simulink model "RB_KAIROS_ArmOnly"  (R2020b)
(part 7 of 17)

t16181 = t3764+t3803+t3810+t3948+t4046+t4050+t4085+t4119+t4165+t4176+t4208+t4212+t4219+t4891+t4926+t4971+t5056+t5175+t5372+t5398+t5435+t5678+t5816+t5817+t6021+t6040+t6076+t6086+t6176+t6724+t6737+t6766+t6881+t6904+t7297+t7298+t7325+t7333+t7439+t7441+t7695+t7716+t7729+t7766+t7770+t7775+t8247+t8476+t8744+t9023+t9032+t9189+t9280+t9289+t9472+t9487+t9501+t9516+t9517+t9646+t9671+t9683+t10139+t10140;
t16199 = q2d.*t16197;
t16214 = t3314+t3315+t3427+t3482+t4058+t4077+t4567+t4627+t4680+t4712+t5459+t5460+t5960+t5966+t5967+t5982+t5983+t5985+t6049+t6067+t6799+t6800+t6849+t6850+t6973+t7051+t7182+t7187+t7194+t7196+t7830+t7883+t8123+t8126+t8203+t8215+t9704+t9713+t9722+t9734+t9976+t9977+t11086+t11087+t11091+t11095+t11106+t11107+t12225+t12226+t12670+t12678+t12680+t12681;
t16218 = q2d.*t16217;
t16236 = t3357+t3450+t3475+t3557+t3579+t3599+t3661+t3722+t3729+t3737+t3906+t3994+t4041+t4051+t4096+t4548+t4568+t4707+t4734+t4818+t4820+t4827+t4853+t4866+t4875+t4912+t4918+t4919+t4920+t5000+t5060+t5416+t5432+t5743+t5753+t5962+t5968+t5970+t5992+t6010+t6020+t6022+t6028+t6093+t6094+t6098+t6127+t6144+t6178+t6189+t6201+t6208+t6279+t6296+t6531+t6656+t6659+t6736+t6765+t6785+t6817+t6954+t7044+t7146+t7222+t7244+t7331+t7334+t7466+t7560+t7689+t7701+t7707+t7713+t8133+t8154+t8198+t8248+t8665+t8757+t8764+t9071+t9188+t9731+t9735+t9782+t9816+t9847+t9867+t10001+t10004+t10038+t10117+t10134+t10178+t10374+t10396;
t16238 = q3d.*t16237;
t16242 = t7826+t8162+t8296+t9175+t9204+t15016+t15218+t16107+t16108+t16109+t16111;
t16254 = t4446+t4631+t4668+t4758+t4768+t5004+t5033+t5197+t5236+t5240+t5250+t7135+t7185+t8618+t8671+t9067+t9259+t13711+t13717+t14544+t14866+t15496+t15502+t15557+t15559+t15561+t15564+t15663+t15664;
t16255 = t4446+t4631+t4668+t4758+t4796+t5004+t5033+t5186+t5242+t5249+t5260+t7125+t7190+t8614+t8666+t9074+t9268+t13711+t13717+t14543+t14862+t15500+t15501+t15556+t15560+t15562+t15563+t15662+t15665;
t16256 = -phid.*(-t4446-t4631-t4668-t4758+t4796+t5014+t5186+t5242+t5249+t5260+t7125+t7190+t8614+t8666+t9074+t9268-t13711+t13715+t14543+t14862+t15500+t15501+t15556+t15560+t15562+t15563+t15662+t15665+t9.*(t348-t525).*8.36241330891889e-4);
t16257 = t4001+t4040+t4652+t4658+t4762+t4785+t4804+t4825+t5253+t5305+t5766+t5791+t7139+t7199+t7204+t8632+t8677+t8904+t9266+t12013+t12015+t12020+t12023+t14555+t14872+t15553+t15555+t15600+t15602+t15607+t15609+t15671+t15672;
t16262 = q2d.*t16261;
t16264 = phid.*t16263;
t16265 = t4407+t4421+t4425+t4429+t4481+t4483+t4903+t4904+t6045+t6411+t6493+t6980+t7029+t7229+t7257+t7327+t8679+t8729+t9991+t9999+t10137+t10723+t12542+t12543+t14808+t14997+t15641+t15646+t15655+t15657+t15682+t15684+t15712+t15714;
t16270 = t4279+t4301+t4305+t4485+t4490+t4518+t4805+t4821+t6374+t6610+t6717+t7397+t7407+t7467+t7795+t7880+t8771+t8847+t10399+t10786+t10943+t10951+t12578+t12579+t14854+t15028+t15692+t15694+t15717+t15718+t15730+t15731+t15751+t15756;
t16271 = phid.*t16269;
t16284 = t3023+t3028+t3789+t3832+t3838+t3847+t3862+t3952+t3954+t3962+t4074+t4086+t4088+t4114+t4156+t4256+t4304+t4824+t4869+t4965+t5075+t5155+t5189+t5271+t5301+t5332+t5335+t5388+t5710+t5794+t5863+t5878+t5886+t6132+t6219+t6237+t6421+t6617+t6657+t6791+t6880+t6898+t6940+t6942+t6963+t6986+t7009+t7100+t7180+t7242+t7299+t7471+t7508+t7570+t7578+t7688+t7733+t7813+t7862+t7863+t7994+t8010+t8089+t8261+t8305+t8565+t8567+t8581+t8839+t8853+t9132+t9211+t9234+t9241+t9250+t9260+t9299+t9328+t9357+t9385+t9409+t9786+t9798+t9947+t10016+t10021+t10168+t10239+t10256+t10679+t10848+t11021+t11028+t11033+t11124+t11334+t11342+t11499+t11500+t11512+t11558+t11577+t11788+t11807;
t16285 = t2955+t2968+t3789+t3801+t3811+t3834+t3896+t3931+t3952+t3962+t4069+t4098+t4107+t4147+t4195+t4280+t4287+t4824+t4869+t4965+t5063+t5155+t5189+t5271+t5311+t5335+t5343+t5388+t5710+t5794+t5863+t5878+t5886+t6132+t6219+t6237+t6421+t6617+t6657+t6791+t6898+t6903+t6940+t6942+t6943+t6986+t7009+t7100+t7180+t7242+t7299+t7476+t7495+t7578+t7585+t7688+t7733+t7813+t7862+t7863+t7984+t8029+t8089+t8261+t8305+t8565+t8572+t8581+t8839+t8853+t9132+t9211+t9234+t9241+t9250+t9260+t9299+t9328+t9345+t9392+t9395+t9786+t9798+t9954+t10016+t10021+t10168+t10243+t10247+t10656+t10848+t11026+t11027+t11033+t11124+t11334+t11342+t11499+t11500+t11512+t11558+t11577+t11788+t11807;
t16325 = t2162+t2193+t2295+t2486+t2503+t2521+t3273+t3298+t3526+t3558+t3662+t3664+t3705+t3754+t3946+t4045+t4647+t4661+t4710+t4733+t4735+t4761+t4789+t4791+t4811+t4815+t4833+t4839+t4850+t4858+t4871+t4979+t4986+t5073+t5103+t5247+t5304+t5650+t5665+t5779+t5809+t5857+t5887+t5945+t6034+t6148+t6171+t6232+t6235+t6313+t6315+t6320+t6330+t6333+t6335+t6351+t6490+t6512+t6536+t6567+t6581+t6777+t6789+t6926+t6977+t7028+t7053+t7077+t7119+t7163+t7168+t7202+t7206+t7209+t7359+t7404+t7480+t7517+t7629+t7685+t7704+t7730+t7866+t7922+t8011+t8012+t8066+t8084+t8088+t8328+t8330+t8541+t8556+t8975+t9053+t9059+t9135+t9137+t9220+t9224+t9373+t9423+t9533+t9535+t9781+t9832+t9907+t9913+t10045+t10054+t10087+t10107+t10205+t10225+t10669+t10781+t10918+t11072+t11151+t11292+t11298+t11311+t11493+t11495+t11514+t11582+t11590+t11612+t11613+t11957+t11963+t11971+t11973;
t16327 = t2162+t2193+t2295+t2502+t2526+t2555+t3273+t3298+t3454+t3606+t3609+t3691+t3705+t3754+t3946+t4027+t4610+t4678+t4694+t4709+t4750+t4790+t4807+t4810+t4819+t4828+t4829+t4842+t4848+t4858+t4859+t4977+t4991+t5073+t5103+t5259+t5295+t5663+t5677+t5779+t5793+t5857+t5876+t5921+t6015+t6128+t6152+t6244+t6248+t6314+t6318+t6320+t6329+t6331+t6350+t6366+t6490+t6523+t6536+t6567+t6581+t6789+t6790+t6926+t6977+t7034+t7047+t7063+t7127+t7147+t7177+t7212+t7218+t7221+t7378+t7416+t7473+t7517+t7629+t7670+t7687+t7730+t7881+t7934+t8030+t8031+t8083+t8084+t8106+t8323+t8338+t8541+t8556+t8975+t9045+t9064+t9130+t9135+t9227+t9238+t9373+t9423+t9545+t9546+t9794+t9821+t9907+t9913+t10033+t10054+t10072+t10093+t10211+t10220+t10647+t10785+t10926+t11072+t11158+t11292+t11298+t11311+t11493+t11495+t11518+t11589+t11597+t11607+t11608+t11952+t11955+t11958+t11964;
t10434 = -t10423;
t10522 = -t10515;
t10601 = -t10592;
t10636 = -t10625;
t10855 = -t10853;
t11011 = -t11004;
t11169 = -t11156;
t11289 = -t11280;
t11406 = -t11395;
t11656 = -t11643;
t11703 = -t11695;
t11828 = -t11823;
t11879 = -t11876;
t11936 = -t11932;
t11998 = -t11992;
t12085 = -t12081;
t12099 = -t12096;
t12121 = -t12115;
t12156 = -t12149;
t12172 = -t12166;
t12285 = -t12282;
t12383 = -t12381;
t12428 = -t12424;
t12434 = t12332.*7.35522e-1;
t12435 = t12333.*7.35522e-1;
t12444 = -t12440;
t12481 = -t12478;
t12488 = t8533+t10393;
t12491 = t8539+t10395;
t12497 = -t12494;
t12498 = -t12495;
t12499 = -t12496;
t12521 = t12333.*3.867742437e-3;
t12523 = t12332.*1.563719772e-3;
t12526 = -t12522;
t12580 = -t12570;
t12581 = -t12571;
t12592 = t16.*t12487.*2.62925e-3;
t12610 = t8.*t12508.*2.62925e-3;
t12611 = -t12607;
t12663 = -t12653;
t12666 = -t12656;
t12684 = (t2501.*t12487)./4.0;
t12723 = -t12720;
t12726 = (t2520.*t12508)./4.0;
t12754 = -t12748;
t12767 = -t12762;
t12769 = t12484.*(t701-t775).*(-1.0./4.0);
t12770 = -t12765;
t12771 = -t12766;
t12777 = (t3365.*t12484)./4.0;
t12778 = (t3455.*t12484)./4.0;
t12779 = (t3421.*t12484)./4.0;
t12785 = (t3489.*t12484)./4.0;
t12797 = -t12794;
t12799 = -t12795;
t12802 = -t12798;
t12803 = (t3732.*t12487)./4.0;
t12804 = -t12800;
t12805 = -t12801;
t12806 = (t3421.*t12506)./4.0;
t12817 = -t12812;
t12831 = -t12829;
t12840 = (t3780.*t12508)./4.0;
t12846 = (t4021.*t12487)./4.0;
t12847 = (t4024.*t12487)./4.0;
t12861 = -t12851;
t12875 = (t4152.*t12484)./4.0;
t12876 = -t12873;
t12877 = (t4021.*t12508)./4.0;
t12879 = -t12874;
t12880 = (t4024.*t12508)./4.0;
t12896 = -t12892;
t12912 = -t12907;
t12913 = -t12908;
t12918 = (t4489.*t12487)./4.0;
t12921 = (t4498.*t12487)./4.0;
t12942 = -t12938;
t12949 = -t12941;
t12957 = (t4509.*t12508)./4.0;
t12959 = (t4514.*t12508)./4.0;
t12989 = -t12984;
t12994 = -t12990;
t12999 = -t12995;
t13003 = -t12997;
t13009 = -t13004;
t13020 = (t4964.*t12484)./4.0;
t13037 = -t13033;
t13041 = (t5007.*t12487)./4.0;
t13046 = -t13044;
t13061 = -t13057;
t13066 = (t5050.*t12508)./4.0;
t13069 = -t13062;
t13070 = -t13063;
t13071 = -t13064;
t13078 = -t13075;
t13081 = (t5234.*t12487)./4.0;
t13082 = (t5235.*t12487)./4.0;
t13096 = t9.*t12945.*1.539925e-2;
t13097 = -t13094;
t13100 = t17.*t12953.*1.539925e-2;
t13102 = -t13099;
t13105 = (t5290.*t12484)./4.0;
t13109 = -t13104;
t13110 = (t5234.*t12508)./4.0;
t13111 = -t13106;
t13112 = (t5235.*t12508)./4.0;
t13160 = (t5524.*t12484)./4.0;
t13166 = (t5552.*t12484)./4.0;
t13172 = t10161+t10206;
t13178 = t9248+t10989;
t13179 = -t13176;
t13180 = (t5696.*t12484)./4.0;
t13193 = -t13192;
t13194 = (t5696.*t12506)./4.0;
t13206 = -t13204;
t13222 = (t5929.*t12487)./4.0;
t13225 = (t5947.*t12487)./4.0;
t13226 = (t5951.*t12487)./4.0;
t13238 = (t3738.*t12945)./4.0;
t13244 = (t3743.*t12953)./4.0;
t13246 = -t13239;
t13247 = -t13241;
t13249 = (t5923.*t12508)./4.0;
t13258 = -t13250;
t13259 = -t13253;
t13260 = (t5952.*t12508)./4.0;
t13263 = (t6096.*t12484)./4.0;
t13272 = (t6014.*t12508)./4.0;
t13283 = (t6158.*t12484)./4.0;
t13286 = -t13282;
t13292 = -t13287;
t13294 = -t13289;
t13299 = -t13298;
t13303 = -t13300;
t13304 = t12484.*(-t2149+t2205+t693.*(t48-t349)+t784.*(t48-t349)).*(-1.0./4.0);
t13306 = (t12484.*(-t2149+t2205+t693.*(t48-t349)+t784.*(t48-t349)))./4.0;
t13308 = (t6302.*t12484)./4.0;
t13318 = -t13316;
t13319 = (t6302.*t12506)./4.0;
t13325 = -t13322;
t13328 = -t13324;
t13329 = t12484.*(t624+t2511-t3502-t9.*t439.*4.252e-3).*(-1.0./4.0);
t13330 = -t13327;
t13332 = (t12484.*(t624+t2511-t3502-t9.*t439.*4.252e-3))./4.0;
t13334 = -t13331;
t13357 = t10379+t10410;
t13371 = t9554+t11157;
t13375 = t17.*t13167.*1.13264871585e-2;
t13389 = t17.*t13175.*1.13264871585e-2;
t13403 = -t13400;
t13418 = -t13417;
t13421 = -t13419;
t13425 = (t6729.*t12487)./4.0;
t13426 = -t13422;
t13434 = -t13429;
t13435 = -t13430;
t13450 = -t13447;
t13455 = (t6744.*t12508)./4.0;
t13457 = t12487.*(-t1540+t2091+t2579+t8.*(t260+t468+t570+t2298)).*(-1.0./4.0);
t13461 = (t12487.*(-t1540+t2091+t2579+t8.*(t260+t468+t570+t2298)))./4.0;
t13473 = -t13468;
t13474 = -t13469;
t13475 = (t6995.*t12487)./4.0;
t13493 = -t13489;
t13494 = (t6957.*t12508)./4.0;
t13499 = (t7066.*t12487)./4.0;
t13506 = (t7079.*t12487)./4.0;
t13511 = -t13505;
t13516 = t9.*t13386.*1.539925e-2;
t13517 = -t13510;
t13525 = -t13520;
t13526 = t12508.*(t1492+t2158+t2696-t4727).*(-1.0./4.0);
t13527 = (t7116.*t12487)./4.0;
t13534 = (t7128.*t12484)./4.0;
t13535 = (t7130.*t12484)./4.0;
t13546 = -t13544;
t13547 = (t7079.*t12508)./4.0;
t13550 = (t7105.*t12508)./4.0;
t13553 = -t13549;
t13554 = (t7116.*t12508)./4.0;
t13556 = -t13552;
t13561 = -t13558;
t13589 = -t13583;
t13598 = (t7336.*t12484)./4.0;
t13601 = (t7402.*t12487)./4.0;
t13626 = (t7434.*t12508)./4.0;
t13643 = -t13642;
t13646 = -t13644;
t13647 = (t7654.*t12484)./4.0;
t13663 = -t13659;
t13666 = -t13662;
t13671 = -t13667;
t13681 = (t3738.*t13386)./4.0;
t13682 = -t13677;
t13695 = -t13690;
t13696 = -t13691;
t13744 = (t8063.*t12484)./4.0;
t13757 = (t5433.*t13175)./4.0;
t13767 = (t8178.*t12487)./4.0;
t13776 = (t8191.*t12484)./4.0;
t13789 = -t13777;
t13790 = (t8227.*t12487)./4.0;
t13799 = t12487.*(-t1476-t1540+t2091+t2165+t2579+t8.*(t260+t468+t570+t2298)).*(-1.0./4.0);
t13803 = (t12487.*(-t1476-t1540+t2091+t2165+t2579+t8.*(t260+t468+t570+t2298)))./4.0;
t13810 = -t13804;
t13819 = -t13815;
t13820 = (t8191.*t12506)./4.0;
t13825 = -t13821;
t13826 = (t8227.*t12508)./4.0;
t13832 = t12508.*(-t1476-t1540+t2091+t2165+t2579+t8.*(t260+t468+t570+t2298)).*(-1.0./4.0);
t13836 = (t8253.*t12508)./4.0;
t13838 = (t12508.*(-t1476-t1540+t2091+t2165+t2579+t8.*(t260+t468+t570+t2298)))./4.0;
t13850 = (t8433.*t12484)./4.0;
t13856 = -t13854;
t13860 = -t13858;
t13868 = -t13865;
t13873 = (t6761.*t12953)./4.0;
t13877 = (t6811.*t12945)./4.0;
t13890 = (t8628.*t12484)./4.0;
t13896 = -t13892;
t13897 = -t13893;
t13904 = -t13900;
t13911 = -t13907;
t13913 = -t13910;
t13925 = -t13922;
t13927 = -t13923;
t13935 = (t8693.*t12484)./4.0;
t13950 = (t5329.*t13386)./4.0;
t13955 = -t13951;
t13957 = -t13952;
t13966 = -t13958;
t13968 = -t13962;
t13970 = -t13965;
t13998 = -t13995;
t14001 = -t14000;
t14040 = (t9196.*t12484)./4.0;
t14062 = t12484.*(t249-t391.*(1.1e+1./1.25e+2)-t1912.*4.252e-3+t3505+t5357+t693.*(t71-t391)+t784.*(t71-t391)).*(-1.0./4.0);
t14070 = -t14065;
t14081 = -t14076;
t14092 = t12506.*(t249-t391.*(1.1e+1./1.25e+2)-t1912.*4.252e-3+t3505+t5357+t693.*(t71-t391)+t784.*(t71-t391)).*(-1.0./4.0);
t14093 = (t12506.*(t249-t391.*(1.1e+1./1.25e+2)-t1912.*4.252e-3+t3505+t5357+t693.*(t71-t391)+t784.*(t71-t391)))./4.0;
t14116 = (t7797.*t13167)./4.0;
t14120 = -t14117;
t14128 = (t7797.*t13175)./4.0;
t14130 = -t14127;
t14144 = -t14141;
t14165 = -t14163;
t14178 = -t14176;
t14184 = -t14183;
t14207 = -t14203;
t14209 = t10208+t12333;
t14213 = t10218+t12332;
t14217 = (t8979.*t12945)./4.0;
t14219 = (t8981.*t12953)./4.0;
t14232 = -t14229;
t14238 = -t14233;
t14245 = -t14242;
t14251 = -t14249;
t14252 = -t14250;
t14283 = t10407+t12414;
t14289 = t17.*t14185.*1.13264871585e-2;
t14345 = t17.*t14280.*1.539925e-2;
t14361 = (t4300.*t14185)./4.0;
t14368 = (t9185.*t13167)./4.0;
t14369 = (t2054.*t14280)./4.0;
t14424 = (t8979.*t13386)./4.0;
t14426 = -t14423;
t14431 = -t14428;
t14434 = -t14430;
t14446 = (t3738.*t14280)./4.0;
t14447 = (t3743.*t14280)./4.0;
t14452 = (t3767.*t14280)./4.0;
t14462 = -t14460;
t14478 = -t14473;
t14482 = -t14480;
t14483 = -t14481;
t14492 = (t5433.*t14185)./4.0;
t14493 = (t5434.*t14185)./4.0;
t14496 = (t5448.*t14185)./4.0;
t14506 = -t14504;
t14508 = (t10149.*t12953)./4.0;
t14510 = (t4517.*t14280)./4.0;
t14511 = t12945.*(t1987-t2621+t3452-t4730+t5359+t9.*(t71-t391).*6.1597e-2+t17.*(t426-t581)).*(-1.0./4.0);
t14530 = (t4772.*t14280)./4.0;
t14566 = -t14563;
t14570 = -t14569;
t14579 = -t14576;
t14584 = (t5217.*t14280)./4.0;
t14589 = (t3738.*t14413)./4.0;
t14591 = -t14588;
t14599 = (t5329.*t14280)./4.0;
t14605 = (t5345.*t14280)./4.0;
t14618 = (t6408.*t14185)./4.0;
t14622 = -t14619;
t14649 = (t5719.*t14280)./4.0;
t14653 = (t5760.*t14280)./4.0;
t14664 = -t14661;
t14684 = (t6781.*t14185)./4.0;
t14690 = (t6038.*t14280)./4.0;
t14699 = (t10469.*t13167)./4.0;
t14711 = (t10469.*t13175)./4.0;
t14720 = -t14718;
t14730 = (t5329.*t14413)./4.0;
t14737 = t13386.*(t1987-t2621+t3452-t4730+t5359+t9.*(t71-t391).*6.1597e-2+t17.*(t426-t581)).*(-1.0./4.0);
t14738 = (t6526.*t14280)./4.0;
t14754 = (t7540.*t14185)./4.0;
t14767 = -t14761;
t14768 = -t14765;
t14774 = -t14771;
t14775 = (t6761.*t14280)./4.0;
t14784 = (t6811.*t14280)./4.0;
t14797 = (t7796.*t14185)./4.0;
t14798 = (t7797.*t14185)./4.0;
t14819 = (t7856.*t14185)./4.0;
t14828 = (t7901.*t14185)./4.0;
t14859 = (t7348.*t14280)./4.0;
t14867 = -t14863;
t14881 = t11165+t13148;
t14884 = (t8464.*t14185)./4.0;
t14885 = -t14883;
t14905 = -t14903;
t14910 = (t14280.*(t2056+t2203+t2351+t3433+t3503+t16.*t389.*(1.1e+1./1.25e+2)))./4.0;
t14932 = (t6811.*t14413)./4.0;
t14934 = (t7940.*t14280)./4.0;
t14941 = (t7982.*t14280)./4.0;
t14949 = t17.*t14879.*1.539925e-2;
t14978 = t12487.*(t1292+t2073+t2694+t11671).*(-1.0./4.0);
t14979 = (t11470.*t13167)./4.0;
t14980 = (t12487.*(t1292+t2073+t2694+t11671))./4.0;
t14984 = (t11470.*t13175)./4.0;
t14991 = (t12392.*t12508)./4.0;
t14995 = (t9049.*t14185)./4.0;
t14996 = (t9050.*t14185)./4.0;
t15020 = (t3743.*t14879)./4.0;
t15027 = (t9185.*t14185)./4.0;
t15030 = (t9194.*t14185)./4.0;
t15034 = (t8725.*t14280)./4.0;
t15068 = -t15067;
t15069 = (t9362.*t14185)./4.0;
t15070 = (t8979.*t14280)./4.0;
t15072 = (t8981.*t14280)./4.0;
t15084 = (t9001.*t14280)./4.0;
t15111 = -t15105;
t15116 = (t9538.*t14185)./4.0;
t15134 = t14280.*(-t2550+t2696+t2698+t4771+t9.*(t260+t468+t570+t2298)+t147.*(t71-t391)).*(-1.0./4.0);
t15135 = (t14280.*(-t2550+t2696+t2698+t4771+t9.*(t260+t468+t570+t2298)+t147.*(t71-t391)))./4.0;
t15137 = (t12487.*t12667)./4.0;
t15143 = (t9197.*t14280)./4.0;
t15147 = -t15146;
t15149 = (t9233.*t14280)./4.0;
t15153 = (t12508.*t12696)./4.0;
t15162 = (t5345.*t14879)./4.0;
t15165 = t14280.*(t3452-t4730+t5359+t9.*(t71-t391).*6.1597e-2+t17.*(t426-t581)).*(-1.0./4.0);
t15167 = (t14280.*(t3452-t4730+t5359+t9.*(t71-t391).*6.1597e-2+t17.*(t426-t581)))./4.0;
t15171 = (t9887.*t14185)./4.0;
t15185 = (t9922.*t14185)./4.0;
t15199 = (t8979.*t14413)./4.0;
t15211 = (t12487.*t12860)./4.0;
t15212 = (t12484.*t12866)./4.0;
t15226 = -t15224;
t15227 = (t12508.*t12867)./4.0;
t15232 = (t12487.*t13005)./4.0;
t15234 = (t12484.*t13005)./4.0;
t15246 = (t12487.*t13019)./4.0;
t15252 = -t15247;
t15254 = -t15249;
t15259 = (t12508.*t13013)./4.0;
t15263 = -t15260;
t15265 = (t12508.*t13038)./4.0;
t15271 = t14185.*(t4324-t5228+t5802+t9.*(t71-t391).*4.5305948634e-2+t17.*(t426-t581).*7.35522e-1).*(-1.0./4.0);
t15272 = (t14185.*(t4324-t5228+t5802+t9.*(t71-t391).*4.5305948634e-2+t17.*(t426-t581).*7.35522e-1))./4.0;
t15274 = (t10468.*t14185)./4.0;
t15275 = (t10469.*t14185)./4.0;
t15283 = (t10485.*t14185)./4.0;
t15285 = t14185.*(-t3823+t3970+t5243+t9.*(t260+t468+t570+t2298).*7.35522e-1+t972.*(t71-t391)+t2777.*(t71-t391)).*(-1.0./4.0);
t15288 = (t14185.*(-t3823+t3970+t5243+t9.*(t260+t468+t570+t2298).*7.35522e-1+t972.*(t71-t391)+t2777.*(t71-t391)))./4.0;
t15294 = (t6761.*t14879)./4.0;
t15299 = (t12484.*t13150)./4.0;
t15316 = -t15313;
t15318 = -t15314;
t15327 = (t10149.*t14280)./4.0;
t15328 = t14280.*(t1987-t2621+t3452-t4730+t5359+t9.*(t71-t391).*6.1597e-2+t17.*(t426-t581)).*(-1.0./4.0);
t15338 = -t15334;
t15344 = (t10180.*t14280)./4.0;
t15378 = (t10763.*t14185)./4.0;
t15380 = (t10783.*t14185)./4.0;
t15390 = (t12484.*t13273)./4.0;
t15399 = (t12484.*t13313)./4.0;
t15404 = -t15403;
t15407 = -t15405;
t15421 = -t15420;
t15434 = -t15432;
t15437 = t14413.*(t1987-t2621+t3452-t4730+t5359+t9.*(t71-t391).*6.1597e-2+t17.*(t426-t581)).*(-1.0./4.0);
t15440 = (t14413.*(t1987-t2621+t3452-t4730+t5359+t9.*(t71-t391).*6.1597e-2+t17.*(t426-t581)))./4.0;
t15443 = -t15442;
t15453 = -t15452;
t15456 = -t15454;
t15464 = t14185.*(t3418-t3879+t4324-t5228+t5802+t9.*(t71-t391).*4.5305948634e-2+t17.*(t426-t581).*7.35522e-1).*(-1.0./4.0);
t15465 = (t11470.*t14185)./4.0;
t15469 = (t11484.*t14185)./4.0;
t15480 = (t8981.*t14879)./4.0;
t15516 = (t12487.*t13876)./4.0;
t15521 = -t15520;
t15522 = (t12508.*t13879)./4.0;
t15537 = t12484.*(t3625+t3660+t9166-t11658).*(-1.0./4.0);
t15538 = (t12484.*(t3625+t3660+t9166-t11658))./4.0;
t15540 = -t15539;
t15548 = -t15547;
t15565 = (t12487.*t14057)./4.0;
t15566 = (t12487.*(-t1476+t2165+t13876))./4.0;
t15574 = -t15571;
t15579 = (t12508.*t14057)./4.0;
t15581 = -t15578;
t15582 = (t12508.*(-t1476+t2165+t13876))./4.0;
t15624 = -t15622;
t15625 = -t15623;
t15630 = t12484.*(t249-t391.*(1.1e+1./1.25e+2)-t1912.*4.252e-3+t3505+t13496+t693.*(t71-t391)+t784.*(t71-t391)).*(-1.0./4.0);
t15633 = (t12484.*(t249-t391.*(1.1e+1./1.25e+2)-t1912.*4.252e-3+t3505+t13496+t693.*(t71-t391)+t784.*(t71-t391)))./4.0;
t15636 = -t15634;
t15639 = -t15637;
t15642 = t12506.*(t249-t391.*(1.1e+1./1.25e+2)-t1912.*4.252e-3+t3505+t13496+t693.*(t71-t391)+t784.*(t71-t391)).*(-1.0./4.0);
t15644 = (t12506.*(t249-t391.*(1.1e+1./1.25e+2)-t1912.*4.252e-3+t3505+t13496+t693.*(t71-t391)+t784.*(t71-t391)))./4.0;
t15675 = -t15673;
t15679 = -t15676;
t15723 = -t15722;
t15867 = (t14156.*t14280)./4.0;
t15882 = (t14185.*t14411)./4.0;
t15884 = t14413.*(t10174+t9.*(t10158+t16.*(t4542-t6448))).*(-1.0./4.0);
t15885 = (t14413.*(t10174+t9.*(t10158+t16.*(t4542-t6448))))./4.0;
t15894 = t14280.*(t2189+t2495+t2635+t2646+t3580+t9.*(t258+t2289+t5392+t7559)+t17.*(t7693+t9904)).*(-1.0./4.0);
t15895 = (t14280.*(t2189+t2495+t2635+t2646+t3580+t9.*(t258+t2289+t5392+t7559)+t17.*(t7693+t9904)))./4.0;
t15901 = (t14280.*t14542)./4.0;
t15921 = (t14280.*t14752)./4.0;
t15922 = (t14185.*t14879)./4.0;
t15927 = t14280.*(-t2550+t2696+t2698+t11659+t8.*t11672+t147.*(t71-t391)).*(-1.0./4.0);
t15929 = (t14280.*(-t2550+t2696+t2698+t11659+t8.*t11672+t147.*(t71-t391)))./4.0;
t15933 = t14185.*(t3471+t3796+t3914+t3942+t4358+t9.*(t258+t2289+t5392+t7559).*7.35522e-1+t17.*(t7693+t9904).*7.35522e-1).*(-1.0./4.0);
t15936 = (t14185.*(t3471+t3796+t3914+t3942+t4358+t9.*(t258+t2289+t5392+t7559).*7.35522e-1+t17.*(t7693+t9904).*7.35522e-1))./4.0;
t15947 = (t14280.*t14823)./4.0;
t15949 = (t14185.*t14919)./4.0;
t15962 = t12953.*(t2091+t2497+t2579+t2680+t3516+t9.*(t210+t2107+t7423+t9121)+t17.*(t9166-t11658)).*(-1.0./4.0);
t15963 = t12945.*(t1987-t2621+t3452+t11654+t9.*(t71-t391).*6.1597e-2+t17.*(t426-t581)+t9.*(t9166-t11658)).*(-1.0./4.0);
t15976 = t14185.*(-t3823+t3970+t11861+t8.*t11864+t972.*(t71-t391)+t2777.*(t71-t391)).*(-1.0./4.0);
t15977 = (t14185.*(-t3823+t3970+t11861+t8.*t11864+t972.*(t71-t391)+t2777.*(t71-t391)))./4.0;
t15988 = (t14185.*t15156)./4.0;
t16003 = t13386.*(t1987-t2621+t3452+t11654+t9.*(t71-t391).*6.1597e-2+t17.*(t426-t581)+t9.*(t9166-t11658)).*(-1.0./4.0);
t16014 = t13167.*(t3423+t3845+t3888+t3925+t4339+t9.*(t210+t2107+t7423+t9121).*7.35522e-1+t17.*(t9166-t11658).*7.35522e-1).*(-1.0./4.0);
t16015 = (t13167.*(t3423+t3845+t3888+t3925+t4339+t9.*(t210+t2107+t7423+t9121).*7.35522e-1+t17.*(t9166-t11658).*7.35522e-1))./4.0;
t16017 = t13175.*(t3423+t3845+t3888+t3925+t4339+t9.*(t210+t2107+t7423+t9121).*7.35522e-1+t17.*(t9166-t11658).*7.35522e-1).*(-1.0./4.0);
t16019 = (t13175.*(t3423+t3845+t3888+t3925+t4339+t9.*(t210+t2107+t7423+t9121).*7.35522e-1+t17.*(t9166-t11658).*7.35522e-1))./4.0;
t16029 = t14280.*(t3452+t11654+t9.*(t71-t391).*6.1597e-2+t17.*(t426-t581)+t9.*(t9166-t11658)).*(-1.0./4.0);
t16030 = (t14280.*(t3452+t11654+t9.*(t71-t391).*6.1597e-2+t17.*(t426-t581)+t9.*(t9166-t11658)))./4.0;
t16034 = t14185.*(t4324+t11855+t9.*(t71-t391).*4.5305948634e-2+t17.*(t426-t581).*7.35522e-1+t9.*(t9166-t11658).*7.35522e-1).*(-1.0./4.0);
t16036 = (t14185.*(t4324+t11855+t9.*(t71-t391).*4.5305948634e-2+t17.*(t426-t581).*7.35522e-1+t9.*(t9166-t11658).*7.35522e-1))./4.0;
t16040 = t14280.*(t2091+t2497+t2579+t2680+t3516+t9.*(t210+t2107+t7423+t9121)+t17.*(t9166-t11658)).*(-1.0./4.0);
t16041 = t14280.*(t1987-t2621+t3452+t11654+t9.*(t71-t391).*6.1597e-2+t17.*(t426-t581)+t9.*(t9166-t11658)).*(-1.0./4.0);
t16043 = (t14280.*(t2091+t2497+t2579+t2680+t3516+t9.*(t210+t2107+t7423+t9121)+t17.*(t9166-t11658)))./4.0;
t16045 = -t16042;
t16046 = -t16044;
t16053 = t14413.*(t1987-t2621+t3452+t11654+t9.*(t71-t391).*6.1597e-2+t17.*(t426-t581)+t9.*(t9166-t11658)).*(-1.0./2.0);
t16054 = (t14413.*(t1987-t2621+t3452+t11654+t9.*(t71-t391).*6.1597e-2+t17.*(t426-t581)+t9.*(t9166-t11658)))./2.0;
t16058 = t14185.*(t3423+t3845+t3888+t3925+t4339+t9.*(t210+t2107+t7423+t9121).*7.35522e-1+t17.*(t9166-t11658).*7.35522e-1).*(-1.0./4.0);
t16059 = t14185.*(t3418-t3879+t4324+t11855+t9.*(t71-t391).*4.5305948634e-2+t17.*(t426-t581).*7.35522e-1+t9.*(t9166-t11658).*7.35522e-1).*(-1.0./4.0);
t16060 = (t14185.*(t3423+t3845+t3888+t3925+t4339+t9.*(t210+t2107+t7423+t9121).*7.35522e-1+t17.*(t9166-t11658).*7.35522e-1))./4.0;
t16073 = t12511+t12518+t12774+t12790;
t16074 = t12513+t12515+t12774+t12790;
t16076 = t14879.*(t2091+t2497+t2579+t2680+t3516+t9.*(t210+t2107+t7423+t9121)+t17.*(t9166-t11658)).*(-1.0./2.0);
t16077 = (t14879.*(t2091+t2497+t2579+t2680+t3516+t9.*(t210+t2107+t7423+t9121)+t17.*(t9166-t11658)))./2.0;
t16105 = q3d.*t16104;
t16135 = t7826+t8162+t8296+t9175+t9204+t11975+t12458+t13276+t13278+t13456+t13466;
t16136 = -q1d.*(t7842+t8174+t8286+t9182+t9210+t11967+t12455+t13269+t13460+(t9292.*(t3418-t3879+t4324-t5228+t5802+t9.*(t71-t391).*4.5305948634e-2+t17.*(t426-t581).*7.35522e-1))./2.0+(t10446.*(t1987-t2621+t3452-t4730+t5359+t9.*(t71-t391).*6.1597e-2+t17.*(t426-t581)))./2.0);
t16139 = q3d.*t16138;
t16145 = t4446+t4631+t4668+t4758+t4768+t5004+t5033+t5197+t5236+t5240+t5250+t6377+t6404+t7135+t7185+t8618+t8671+t9067+t9259+t9893+t9895+t10310+t10592+t10596+t10715+t10718+t11444+t11694+t11695;
t16156 = t4001+t4040+t4652+t4658+t4762+t4785+t4804+t4825+t5253+t5305+t5649+t5661+t5698+t5701+t5766+t5791+t7139+t7199+t7204+t8632+t8677+t8904+t9266+t10330+t10589+t10591+t10853+t10861+t10967+t10977+t11455+t11823+t11832;
t16163 = q2d.*t16162;
t16166 = t4407+t4421+t4425+t4429+t4481+t4483+t4903+t4904+t5100+t5108+t5590+t5596+t6045+t6411+t6493+t6980+t7029+t7229+t7257+t7327+t8679+t8729+t10137+t10723+t11197+t11467+t11468+t11605+t11609+t11876+t11887+t11909+t12115+t12123;
t16173 = t4279+t4301+t4305+t4485+t4490+t4518+t4805+t4821+t5206+t5225+t5813+t5844+t6374+t6610+t6717+t7397+t7407+t7467+t7795+t7880+t8771+t8847+t10399+t10786+t11350+t12022+t12035+t12047+t12143+t12149+t12294+t12304+t12421+t12424;
t16179 = -q1d.*(t4484+t4576+t4580+t4749+t4773+t4786+t5002+t5030+t5643+t5658+t6384+t6387-t6965+t7258-t7472-t7744-t8540-t8593+t9003-t11218+t11611-t11933+t12178-t12640+t12643+t12748-t12895+t12899+t12984+(t6276.*(t1918+t9.*(t71-t391)))./4.0+(t8622.*(t395+t9.*(t48-t349)))./4.0+(t7949.*(t3418-t3879+t4324-t5228+t5802+t9.*(t71-t391).*4.5305948634e-2+t17.*(t426-t581).*7.35522e-1))./4.0+(t9361.*(t1987-t2621+t3452-t4730+t5359+t9.*(t71-t391).*6.1597e-2+t17.*(t426-t581)))./4.0+(t1907.*(t1912.*(-1.0027e-2)+t2709+t3492+t751.*(t71-t391)))./4.0);
t16206 = t5871+t5932+t6011+t6547+t6771+t6825+t7106+t7173+t7872+t7979+t7989+t8234+t8523+t8627+t8915+t9073+t9097+t9579+t10144+t10314+t10343+t10747+t10764+t11189+t11200+t11212+t11544+t11561+t11587+t12768+t12889+t13302+t13305+t13407+t13409;
t16215 = q2d.*t16214;
t16245 = t3953+t4000+t4379+t4397+t4412+t4427+t4435+t4440+t4492+t4826+t4836+t4921+t4940+t5074+t5099+t5338+t5379+t5403+t5811+t5893+t6326+t6378+t6416+t6528+t6532+t6575+t7027+t7140+t7189+t7610+t7619+t8021+t8164+t8580+t8645+t8663+t8691+t8880+t9199+t9283+t9291+t9324+t9330+t9544+t9558+t9714+t9751+t9840+t10186+t10200+t10440+t10525+t10672+t10841+t10889+t10894+t10915+t11004+t11007+t11123+t11136+t11573+t11639+t11643+t12089+t12096;
t16266 = t4225+t4232+t4268+t4409+t4413+t4417+t4698+t4715+t4813+t5184+t5238+t5651+t5684+t6075+t6379+t6394+t6485+t6572+t6618+t6635+t7123+t7183+t7243+t7432+t7449+t7565+t7640+t7921+t7941+t8134+t8184+t8284+t8579+t8659+t8767+t8814+t8909+t10120+t10431+t10482+t10638+t10645+t10739+t10749+t10790+t10796+t10856+t11051+t11054+t11105+t11115+t11137+t11423+t11491+t11699+t11718+t11725+t12093+t12254+t12431+t12432+t12572+t12585+t12594+t12599+t12815+t12821;
t16268 = t4253+t4259+t4288+t4380+t4434+t4441+t4663+t4685+t4794+t5160+t5245+t5664+t5673+t6075+t6379+t6394+t6485+t6572+t6618+t6635+t7123+t7183+t7243+t7432+t7449+t7565+t7640+t7921+t7941+t8134+t8184+t8284+t8601+t8652+t8767+t8814+t8909+t10120+t10431+t10487+t10628+t10666+t10739+t10749+t10790+t10796+t10856+t11051+t11054+t11105+t11115+t11137+t11430+t11491+t11699+t11717+t11726+t12093+t12254+t12431+t12432+t12572+t12585+t12594+t12599+t12815+t12821;
t16278 = t7842+t8174+t8286+t9182+t9210+t11388+t11398+t11968+t12456+t13211+t13217+t15013+t15216+t15822+t15824+t15826+t15829+t15860+t15862+t15864+t15865;
t16279 = t7826+t8162+t8296+t9175+t9204+t11388+t11398+t11976+t12459+t13211+t13217+t15017+t15219+t15823+t15825+t15827+t15828+t15859+t15861+t15863+t15866;
t16280 = -phid.*(t7842+t8174+t8286+t9182+t9210+t11968+t12456-t13211+t13214+t15013+t15216+t15822+t15824+t15826+t15829+t15860+t15862+t15864+t15865+t9.*(t8963+t7.*(t5026+t5.*(t2959-t2967))).*3.867742437e-3+t17.*(t8963+t7.*(t5026+t5.*(t2959-t2967))).*1.563719772e-3);
t16286 = q2d.*t16284;
t16316 = t3193+t3197+t3929+t3935+t3975+t3984+t4022+t4053+t4109+t4131+t4172+t4179+t4222+t4284+t4297+t4311+t4377+t4996+t5037+t5090+t5171+t5409+t5425+t5431+t5493+t5607+t5700+t5738+t6263+t6322+t6415+t6422+t6434+t6468+t6628+t6734+t6792+t7069+t7093+t7096+t7169+t7171+t7525+t7534+t7555+t7598+t7631+t7662+t7780+t7819+t7892+t7902+t7936+t7973+t8121+t8342+t8377+t8410+t8673+t8700+t8714+t8752+t8766+t8813+t8949+t8993+t9043+t9052+t9338+t9604+t9606+t9715+t9849+t9850+t9866+t9870+t9871+t9878+t9956+t9958+t9962+t10105+t10248+t10257+t10536+t10544+t10549+t10555+t10777+t10881+t11306+t11321+t11505+t11696+t11899+t12063+t12074+t12116+t12207+t12213+t12381+t12389+t12477+t12478;
t16326 = q2d.*t16325;
t16330 = -q1d.*(t3806+t3818+t3974+t3983+t4108+t4155+t4171+t4184+t4245+t4316+t4343+t4431+t4439+t4766+t4803+t5368+t5520+t5548+t5627+t5717+t5768+t5770+t5792+t5799+t6059+t6157+t6266+t6389+t6426+t6429+t6557+t6564+t6945+t7035+t7143+t7203+t7211+t7375+t7592+t7616+t7706+t7711+t7812+t7816+t7843+t7906+t7924+t8200+t8257+t8359+t8409+t8611+t8625+t8664+t8726+t8901+t8924+t8965+t9004+t9192+t9308-t9352+t9672+t9676+t9883+t9900+t9927+t9937+t9938-t9969+t9990+t10015+t10281+t10347+t10366+t10516+t10717-t10751+t10788-t10805+t11029-t11060+t11104-t11133+t11302+t11310+t11411+t12001+t12003-t12356+t12404-t12460+t12490+t12812+t12813+t12938+t12940+(t8979.*(t2740+t3849+t3968+t3972-t5255+t17.*(t260+t468+t570+t2298).*7.35522e-1))./4.0+(t7646.*(-t1476-t1540+t2091+t2165+t2579+t8.*(t260+t468+t570+t2298)))./4.0+(t8981.*(-t3823+t3970+t5243+t9.*(t260+t468+t570+t2298).*7.35522e-1+t972.*(t71-t391)+t2777.*(t71-t391)))./4.0+(t9112.*(t1492+t2158+t2696-t4727))./4.0+(t7116.*(t3063+t3528+t3966-t5230))./4.0+(t6014.*(-t3045-t3218+t3458+t3539+t3878+t8.*(t260+t468+t570+t2298).*1.666555))./4.0+(t10468.*(t824+t2543+t2699+t2707-t4767+t17.*(t260+t468+t570+t2298)))./4.0+(t10469.*(-t2550+t2696+t2698+t4771+t9.*(t260+t468+t570+t2298)+t147.*(t71-t391)))./4.0);
t16341 = t2321+t2334+t2385+t2808+t2986+t3332+t3401+t3586+t3769+t3843+t3927+t3947+t3987+t4516+t4847+t4867+t4868+t4897+t4937+t4984+t4995+t5133+t5173+t5246+t5326+t5412+t5419+t5507+t5614+t5626+t5636+t5656+t5672+t5722+t5870+t5936+t6013+t6170+t6185+t6349+t6381+t6467+t6518+t6568+t6576+t6616+t6644+t6651+t6662+t6721+t6726+t6735+t6747+t6772+t6813+t6835+t6933+t6968+t7048+t7112+t7126+t7193+t7230+t7301+t7307+t7435+t7484+t7500+t7550+t7584+t7765+t7784+t7824+t7919+t7981+t8051+t8091+t8136+t8299+t8301+t8324+t8434+t8675+t8692+t8705+t8798+t8873+t8912+t8945+t9041+t9093+t9129+t9131+t9154+t9201+t9341+t9597+t9615+t9695+t9709+t9942+t9943+t10024+t10059+t10068+t10075+t10155+t10342+t10361+t10510+t10513+t10624+t10772+t10782+t11148+t11347+t11381+t11516+t11536+t11556+t11568+t11816+t11820+t11915+t12125+t12232+t12236+t12239+t12241+t12570+t12571+t12574+t12575;
t16352 = t5882+t5909+t5994+t6543+t6782+t6854+t7120+t7165+t7889+t7975+t7991+t8246+t8535+t8621+t8894+t9066+t9109+t12223+t12606+t15040+t15046+t15138+t15142+t15243+t15374+t15616+t15617+t15653+t15654+t15785+t15793+t16091+t16092+t16096+t16097;
t16357 = t2320+t2333+t2384+t3146+t3288+t3303+t3305+t3351+t3740+t4007+t4025+t4048+t4164+t4320+t4571+t4863+t4946+t4985+t5104+t5114+t5279+t5328+t5355+t5375+t5406+t5521+t5645+t5747+t5771+t5790+t5907+t5980+t6061+t6136+t6292+t6454+t6571+t6648+t6666+t6668+t6700+t6760+t6829+t6845+t6891+t6895+t6922+t6936+t7006+t7013+t7091+t7110+t7220+t7253+t7256+t7267+t7273+t7291+t7340+t7554+t7564+t7566+t7626+t7664+t7714+t7737+t7825+t7850+t7885+t7910+t7986+t8001+t8122+t8346+t8375+t8385+t8429+t8598+t8639+t8649+t8684+t8718+t8737+t8827+t8874+t8959+t8997+t9313+t9527+t9568+t9570+t9572+t9592+t9645+t9667+t9720+t9739+t9916+t9929+t9987+t10026+t10246+t10253+t10450+t10465+t10614+t10818+t10827+t10879+t10932+t10933+t10984+t10991+t11031+t11114+t11118+t11257+t11410+t11849+t12019+t12145+t12152+t12222+t12352+t12357+t12372+t12376+t12462+t12833+t12834+t12848+t12849+t12990+t12995+t13007+t13008;
t16391 = t3629+t3663+t3770+t4422+t4525+t4674+t4812+t4968+t5288+t5896+t5946+t6260+t6362+t6406+t6948+t7038+t7050+t7350+t7627+t7673+t7788+t7971+t8014+t8104+t8469+t8491+t8722+t8777+t8891+t9042+t9080+t11315+t11333+t11478+t11480+t11759+t12146+t12534+t12538+t12756+t12757+t13622+t13709+t14858+t14868+t14900+t14916+t15186+t15187+t15748+t15750+t15757+t15758+t15842+t15843+t16099+t16100+t16101+t16103;
t16393 = t559+t568+t2420+t2424+t4026+t4032+t4549+t4563+t4638+t4673+t5341+t5378+t5895+t5897+t6074+t6111+t6987+t7068+t7073+t7092+t7094+t7152+t7260+t7860+t7951+t8119+t8250+t8264+t8274+t8289+t9014+t9026+t9160+t9162+t9205+t9208+t9643+t9644+t10692+t10710+t10840+t10842+t11476+t11685+t12917+t12919+t12920+t12924+t13785+t13786+t14785+t14786+t14804+t14805+t15063+t15066+t15696+t15697+t15698+t15699+t15815+t15816+t16080+t16082+t16083+t16084;
t16425 = t3933+t4005+t4112+t4113+t4134+t4154+t4229+t4246+t4307+t4325+t4454+t4458+t4463+t4523+t5038+t5089+t5148+t5157+t5202+t5353+t5381+t5473+t5512+t5567+t5662+t6241+t6342+t6347+t6369+t6562+t6652+t6708+t6712+t6714+t6723+t6769+t6919+t7058+t7523+t7596+t7597+t7609+t7679+t7760+t7988+t8037+t8078+t8196+t8425+t8662+t8680+t8736+t9599+t9605+t11358+t11735+t12249+t12295+t12362+t12366+t12573+t12590+t12742+t12746+t12897+t13126+t13129+t13162+t13163+t13169+t13171+t13201+t13205+t13228+t13236+t13512+t13515+t13726+t13750+t14080+t14089+t14100+t14374+t14379+t14569+t14572+t14860+t14864+t14940+t15021+t15061+t15064+t15335+t15343+t15347+t15353+t15701+t15702+t15727+t15728;
t16428 = t3929+t3935+t4022+t4053+t4109+t4131+t4172+t4179+t4222+t4284+t4297+t4311+t4377+t4996+t5037+t5090+t5171+t5409+t5425+t5431+t5493+t5607+t5700+t5738+t6263+t6322+t6415+t6422+t6434+t6468+t6628+t6734+t6792+t7069+t7093+t7096+t7169+t7171+t7525+t7534+t7555+t7598+t7631+t7662+t7780+t7819+t7892+t7902+t7936+t7973+t8228+t8236+t8394+t8410+t8412+t8673+t8714+t8752+t11389+t12269+t12377+t12890+t12905+t12939+t12961+t13002+t13025+t13039+t13219+t13231+t13335+t13337+t13343+t13346+t13347+t13355+t13410+t13585+t13590+t13734+t13738+t13828+t13846+t14097+t14150+t14187+t14436+t14444+t14619+t14628+t14990+t15106+t15120+t15121+t15269+t15270+t15446+t15448+t15461+t15462+t15743+t15744+t15764+t15765;
t16441 = t4108+t4155+t4171+t4184+t4245+t4316+t4343+t4431+t4439+t4766+t4803+t5368+t5520+t5548+t5627+t5717+t5768+t5770+t5792+t5799+t6059+t6157+t6266+t6383+t6389+t6391+t6426+t6429+t6557+t6564+t6945+t7035+t7143+t7203+t7211+t7375+t7592+t7616+t7706+t7711+t7812+t7816+t7843+t7906+t7924+t8200+t8257+t8359+t8409+t8432+t8436+t8611+t8625+t8664+t8726+t8924+t9004+t9308+t9937+t12038+t12101+t12539+t12692+t12954+t12980+t13284+t13285+t13358+t13365+t13396+t13406+t13451+t13462+t13610+t13618+t13630+t13780+t13816+t13824+t13852+t13980+t13993+t13994+t14010+t14069+t14397+t14459+t14673+t14678+t14761+t14773+t14853+t14856+t15044+t15045+t15194+t15228+t15549+t15552+t15580+t15586+t15788+t15789+t15799+t15800;
t16447 = t2262+t2305+t2385+t2808+t2986+t3332+t3401+t3586+t3769+t3843+t3927+t3947+t3987+t4516+t4847+t4867+t4868+t4897+t4937+t4984+t4995+t5133+t5173+t5246+t5326+t5614+t5626+t5636+t5722+t5870+t5936+t6013+t6170+t6185+t6349+t6381+t6467+t6518+t6568+t6576+t6616+t6644+t6721+t6747+t6813+t6835+t6933+t6968+t7048+t7112+t7126+t7230+t7435+t7500+t7550+t7584+t7765+t7784+t7824+t7845+t7847+t7919+t7981+t8051+t8091+t8301+t8324+t8434+t8705+t8798+t8912+t9087+t10154+t10157+t10267+t10277+t10444+t10524+t10804+t10921+t10922+t11208+t11214+t11221+t11331+t11397+t11650+t11676+t11798+t11830+t11953+t11982+t12272+t12378+t12379+t12483+t12665+t12674+t13052+t13067+t13090+t13437+t13448+t13732+t13742+t13746+t13835+t13843+t13902+t13905+t13959+t13964+t14013+t14302+t14304+t14355+t14364+t14559+t14561+t14661+t14668+t15001+t15115+t15356+t15360+t15363+t15364+t15375+t15376+t15400+t15401+t15767+t15770+t15772+t15773;
t16455 = t2261+t2304+t2384+t3029+t3288+t3303+t3305+t3351+t3761+t4007+t4008+t4048+t4164+t4338+t4556+t4877+t4955+t4985+t5098+t5102+t5269+t5340+t5367+t5375+t5406+t5629+t5632+t5660+t5757+t5762+t5800+t5808+t5825+t5891+t5997+t6079+t6156+t6307+t6463+t6571+t6648+t6660+t6676+t6700+t6770+t6867+t6871+t6891+t6947+t6998+t7006+t7101+t7102+t7312+t7365+t7564+t7571+t7580+t7626+t7664+t7810+t7836+t7972+t8018+t8139+t8335+t8376+t8384+t8575+t8639+t8657+t8684+t8718+t8731+t8807+t8951+t9113+t10461+t10686+t10825+t10829+t10978+t11001+t11184+t11194+t11263+t11287+t11408+t11418+t11513+t11868+t11983+t12157+t12196+t12202+t12209+t12308+t12319+t12380+t12390+t12406+t12759+t12937+t13159+t13262+t13275+t13449+t13471+t13579+t13588+t13670+t13684+t13981+t14044+t14159+t14168+t14221+t14225+t14228+t14262+t14635+t14682+t14726+t14727+t14762+t14764+t15126+t15130+t15168+t15176+t15180+t15217+t15490+t15491+t15498+t15499+t15804+t15805+t15806+t15807;
t16456 = t2175+t2228+t2411+t3029+t3272+t3322+t3325+t3397+t3761+t3986+t4008+t4068+t4200+t4338+t4556+t4877+t4955+t4999+t5098+t5102+t5269+t5340+t5364+t5367+t5397+t5610+t5615+t5660+t5757+t5762+t5800+t5812+t5819+t5891+t5997+t6079+t6156+t6307+t6463+t6563+t6660+t6661+t6676+t6686+t6770+t6865+t6867+t6871+t6947+t6998+t7026+t7101+t7102+t7312+t7365+t7548+t7571+t7580+t7644+t7649+t7810+t7836+t7972+t8018+t8139+t8335+t8376+t8384+t8575+t8647+t8657+t8688+t8712+t8731+t8807+t8951+t9113+t10461+t10691+t10825+t10829+t10978+t11001+t11184+t11194+t11256+t11296+t11408+t11418+t11515+t11868+t11983+t12157+t12195+t12203+t12216+t12308+t12319+t12380+t12390+t12406+t12761+t12937+t13159+t13262+t13275+t13454+t13463+t13579+t13588+t13675+t13679+t13981+t14044+t14159+t14168+t14223+t14225+t14228+t14264+t14635+t14682+t14726+t14727+t14762+t14764+t15124+t15128+t15168+t15174+t15178+t15217+t15490+t15491+t15498+t15499+t15804+t15805+t15806+t15807;
t16457 = -phid.*(t2261+t2304+t2384+t3146+t3288+t3303+t3305+t3351+t3740+t4007+t4025+t4048+t4164+t4320+t4571+t4863+t4946+t4985+t5104+t5114+t5279+t5328+t5355+t5375+t5406+t5629+t5632+t5645+t5747+t5771+t5790+t5808+t5825+t5907+t5980+t6061+t6136+t6292+t6454+t6571+t6648+t6666+t6668+t6700+t6760+t6829+t6891+t6895+t6922+t7006+t7013+t7091+t7110+t7291+t7340+t7554+t7564+t7566+t7626+t7664+t7825+t7850+t7986+t8001+t8122+t8346+t8375+t8385+t8598+t8639+t8649+t8684+t8718+t8737+t8827+t8959+t9105+t10453+t10686-t10825-t10829-t10978+t10993-t11184+t11191+t11263+t11287-t11408-t11418+t11513-t11868+t11980+t12150+t12196+t12202+t12209-t12308-t12319-t12380-t12390-t12406+t12759+t12934+t13157-t13262-t13275+t13449+t13471-t13579-t13588+t13670+t13684+t13978+t14042-t14159+t14166+t14221-t14225+t14226+t14262-t14635-t14682-t14726-t14727-t14762-t14764+t15126+t15130+t15176+t15180+t15488+t15489+t15494+t15495+(t7987.*(t3418-t3879+t4324+t11855+t9.*(t71-t391).*4.5305948634e-2+t17.*(t426-t581).*7.35522e-1+t9.*(t9166-t11658).*7.35522e-1))./4.0+(t7130.*(t1589-t2213-t4346+t4355+t9454+t11863+t2772.*(t71-t391)+t2775.*(t71-t391)))./4.0+(t7982.*(t3423+t3845+t3888+t3925+t4339+t9.*(t210+t2107+t7423+t9121).*7.35522e-1+t17.*(t9166-t11658).*7.35522e-1))./4.0+(t9310.*(t249-t391.*(1.1e+1./1.25e+2)-t1912.*4.252e-3+t3505+t13496+t693.*(t71-t391)+t784.*(t71-t391)))./4.0+(t9887.*(t2091+t2497+t2579+t2680+t3516+t9.*(t210+t2107+t7423+t9121)+t17.*(t9166-t11658)))./4.0+(t9896.*(t1987-t2621+t3452+t11654+t9.*(t71-t391).*6.1597e-2+t17.*(t426-t581)+t9.*(t9166-t11658)))./4.0);
t16476 = t2886+t3390+t3442+t3518+t3568+t3602+t3605+t3642+t3707+t3844+t4095+t4100+t4148+t4224+t4241+t4293+t4497+t4606+t4626+t4665+t4736+t4742+t4834+t4901+t4911+t4963+t4998+t5222+t5278+t5873+t5881+t5890+t5935+t5943+t5998+t6065+t6071+t6072+t6088+t6118+t6120+t6153+t6186+t6192+t6231+t6305+t6585+t6594+t6669+t6728+t6755+t6894+t6946+t7015+t7059+t7179+t7184+t7208+t7239+t7349+t7403+t7421+t7465+t7499+t7607+t7712+t7747+t7787+t7793+t7898+t7923+t7946+t7953+t8035+t8060+t8157+t8197+t8322+t8345+t8441+t8456+t8493+t8503+t8550+t8577+t8607+t8695+t8727+t8832+t8840+t8928+t8940+t9006+t9030+t9055+t9061+t9116+t9170+t9190+t9195+t9455+t9577+t9586+t9616+t9909+t9914+t9917+t9919+t10315+t10320+t10483+t10500+t11078+t11079+t11465+t11469+t11510+t11893+t11905+t12102+t12108+t12474+t12482+t12530+t12630+t12869+t12882+t12887+t12891+t12926+t13154+t13604+t13607+t13631+t13640+t13654+t13674+t13730+t13753+t13874+t13881+t14124+t14126+t14244+t14274+t14275+t14284+t14285+t14337+t14709+t14710+t14917+t14920+t14922+t14923+t15286+t15292+t15324+t15325+t15336+t15337+t15589+t15590+t15591+t15592+t15830+t15831+t15832+t15833;
t16478 = t2987+t3390+t3442+t3518+t3568+t3602+t3605+t3679+t3707+t3892+t4100+t4115+t4126+t4224+t4264+t4293+t4497+t4606+t4626+t4665+t4736+t4742+t4834+t4898+t4901+t4972+t5018+t5237+t5278+t5873+t5890+t5892+t5953+t5963+t5998+t6065+t6071+t6072+t6088+t6118+t6120+t6153+t6186+t6192+t6231+t6291+t6584+t6596+t6678+t6741+t6745+t6894+t6946+t7015+t7059+t7179+t7184+t7208+t7239+t7349+t7403+t7410+t7465+t7499+t7593+t7712+t7757+t7801+t7811+t7878+t7923+t7946+t7953+t8035+t8079+t8157+t8197+t8322+t8345+t8441+t8456+t8493+t8503+t8550+t8577+t8607+t8703+t8732+t8832+t8858+t8928+t8940+t9006+t9030+t9055+t9061+t9116+t9178+t9184+t9200+t9455+t9577+t9586+t9616+t9909+t9914+t9917+t9919+t10313+t10322+t10478+t10500+t11078+t11079+t11465+t11469+t11506+t11893+t11905+t12100+t12106+t12472+t12480+t12530+t12630+t12869+t12882+t12887+t12891+t12931+t13155+t13604+t13607+t13631+t13640+t13657+t13680+t13730+t13753+t13878+t13883+t14124+t14126+t14247+t14274+t14275+t14284+t14285+t14340+t14709+t14710+t14917+t14920+t14922+t14923+t15286+t15292+t15320+t15321+t15332+t15333+t15589+t15590+t15591+t15592+t15830+t15831+t15832+t15833;
t12525 = -t12521;
t12527 = -t12523;
t12596 = -t12592;
t12615 = -t12610;
t12691 = -t12684;
t12731 = -t12726;
t12780 = -t12777;
t12782 = -t12778;
t12783 = -t12779;
t12809 = -t12806;
t12853 = -t12846;
t12855 = -t12847;
t12881 = -t12875;
t12883 = -t12877;
t12885 = -t12880;
t12923 = -t12918;
t12963 = -t12957;
t12964 = -t12959;
t13086 = -t13081;
t13088 = -t13082;
t13116 = -t13112;
t13168 = -t13166;
t13184 = -t13180;
t13195 = -t13194;
t13230 = -t13225;
t13232 = -t13226;
t13243 = -t13238;
t13251 = -t13244;
t13257 = -t13249;
t13265 = -t13260;
t13267 = -t13263;
t13309 = -t13308;
t13362 = t10383+t10434;
t13377 = t9557+t11169;
t13379 = -t13375;
t13384 = t9.*t13172.*1.13264871585e-2;
t13392 = -t13389;
t13393 = t9.*t13178.*1.13264871585e-2;
t13476 = t17.*t13357.*1.539925e-2;
t13477 = -t13475;
t13498 = t17.*t13371.*1.539925e-2;
t13500 = -t13494;
t13513 = -t13506;
t13524 = -t13516;
t13536 = -t13527;
t13541 = -t13535;
t13548 = -t13547;
t13557 = -t13554;
t13628 = -t13626;
t13649 = -t13647;
t13668 = (t3743.*t13371)./4.0;
t13686 = -t13681;
t13761 = -t13757;
t13764 = (t5434.*t13178)./4.0;
t13787 = -t13776;
t13823 = -t13820;
t13830 = -t13826;
t13880 = -t13877;
t13928 = (t5345.*t13357)./4.0;
t13940 = -t13935;
t13946 = (t5345.*t13371)./4.0;
t13954 = -t13950;
t14108 = (t6761.*t13357)./4.0;
t14119 = -t14116;
t14121 = (t7796.*t13172)./4.0;
t14131 = -t14128;
t14134 = (t7796.*t13178)./4.0;
t14218 = -t14217;
t14220 = -t14219;
t14297 = t10435+t12435;
t14299 = t10443+t12434;
t14301 = t17.*t14209.*1.13264871585e-2;
t14305 = t9.*t14213.*1.13264871585e-2;
t14362 = -t14361;
t14370 = -t14368;
t14373 = -t14369;
t14383 = (t9194.*t13172)./4.0;
t14385 = (t4300.*t14209)./4.0;
t14391 = (t4298.*t14213)./4.0;
t14410 = (t8981.*t13357)./4.0;
t14416 = (t8981.*t13371)./4.0;
t14427 = -t14424;
t14449 = -t14446;
t14451 = -t14447;
t14456 = -t14452;
t14494 = -t14492;
t14495 = -t14493;
t14499 = -t14496;
t14512 = -t14508;
t14513 = -t14510;
t14514 = (t5433.*t14209)./4.0;
t14515 = (t5434.*t14209)./4.0;
t14518 = (t5448.*t14209)./4.0;
t14519 = (t5433.*t14213)./4.0;
t14520 = (t5434.*t14213)./4.0;
t14525 = (t5449.*t14213)./4.0;
t14536 = -t14530;
t14586 = -t14584;
t14592 = -t14589;
t14610 = -t14605;
t14621 = -t14618;
t14636 = (t6408.*t14209)./4.0;
t14638 = (t6397.*t14213)./4.0;
t14651 = -t14649;
t14686 = -t14684;
t14693 = -t14690;
t14697 = (t6781.*t14209)./4.0;
t14700 = (t6780.*t14213)./4.0;
t14701 = -t14699;
t14703 = (t10468.*t13172)./4.0;
t14712 = -t14711;
t14713 = (t10468.*t13178)./4.0;
t14728 = (t10149.*t13357)./4.0;
t14732 = (t10149.*t13371)./4.0;
t14739 = -t14738;
t14756 = -t14754;
t14778 = -t14775;
t14780 = (t7540.*t14209)./4.0;
t14787 = (t7538.*t14213)./4.0;
t14789 = -t14784;
t14803 = -t14798;
t14824 = -t14819;
t14831 = (t7796.*t14209)./4.0;
t14832 = (t7797.*t14209)./4.0;
t14836 = (t7796.*t14213)./4.0;
t14837 = (t7797.*t14213)./4.0;
t14841 = (t7828.*t14213)./4.0;
t14842 = (t7856.*t14209)./4.0;
t14846 = (t7901.*t14209)./4.0;
t14848 = (t7913.*t14213)./4.0;
t14861 = -t14859;
t14886 = -t14884;
t14906 = (t8464.*t14209)./4.0;
t14911 = (t8460.*t14213)./4.0;
t14912 = -t14910;
t14937 = -t14934;
t14943 = -t14941;
t14953 = -t14949;
t14982 = t13172.*(t3418-t3879+t4324-t5228+t5802+t9.*(t71-t391).*4.5305948634e-2+t17.*(t426-t581).*7.35522e-1).*(-1.0./4.0);
t14989 = t13178.*(t3418-t3879+t4324-t5228+t5802+t9.*(t71-t391).*4.5305948634e-2+t17.*(t426-t581).*7.35522e-1).*(-1.0./4.0);
t14993 = -t14991;
t14998 = -t14995;
t14999 = -t14996;
t15007 = (t9049.*t14209)./4.0;
t15008 = (t9050.*t14209)./4.0;
t15014 = (t9048.*t14213)./4.0;
t15015 = t14213.*(t3085-t3419-t3773+t5128+t17.*(t208-t427).*7.35522e-1).*(-1.0./4.0);
t15018 = (t14213.*(t3085-t3419-t3773+t5128+t17.*(t208-t427).*7.35522e-1))./4.0;
t15023 = -t15020;
t15029 = -t15027;
t15032 = -t15030;
t15036 = -t15034;
t15051 = (t9185.*t14209)./4.0;
t15053 = (t9194.*t14209)./4.0;
t15054 = (t9185.*t14213)./4.0;
t15058 = (t9194.*t14213)./4.0;
t15073 = -t15069;
t15075 = -t15070;
t15078 = -t15072;
t15092 = (t9362.*t14209)./4.0;
t15102 = (t9361.*t14213)./4.0;
t15118 = -t15116;
t15125 = (t9538.*t14209)./4.0;
t15129 = (t9537.*t14213)./4.0;
t15144 = -t15143;
t15157 = -t15153;
t15164 = -t15162;
t15173 = -t15171;
t15188 = -t15185;
t15189 = (t9887.*t14209)./4.0;
t15193 = (t9896.*t14213)./4.0;
t15202 = (t9922.*t14209)./4.0;
t15206 = (t9926.*t14213)./4.0;
t15213 = -t15212;
t15262 = -t15259;
t15266 = -t15265;
t15277 = -t15274;
t15278 = -t15275;
t15289 = t14209.*(t4324-t5228+t5802+t9.*(t71-t391).*4.5305948634e-2+t17.*(t426-t581).*7.35522e-1).*(-1.0./4.0);
t15291 = (t14209.*(t4324-t5228+t5802+t9.*(t71-t391).*4.5305948634e-2+t17.*(t426-t581).*7.35522e-1))./4.0;
t15293 = (t10446.*t14213)./4.0;
t15295 = (t10468.*t14209)./4.0;
t15296 = (t10469.*t14209)./4.0;
t15298 = -t15294;
t15303 = (t10468.*t14213)./4.0;
t15304 = (t10469.*t14213)./4.0;
t15308 = (t10485.*t14209)./4.0;
t15310 = (t10480.*t14213)./4.0;
t15312 = t14209.*(-t3823+t3970+t5243+t9.*(t260+t468+t570+t2298).*7.35522e-1+t972.*(t71-t391)+t2777.*(t71-t391)).*(-1.0./4.0);
t15315 = (t14209.*(-t3823+t3970+t5243+t9.*(t260+t468+t570+t2298).*7.35522e-1+t972.*(t71-t391)+t2777.*(t71-t391)))./4.0;
t15319 = t14213.*(t2740+t3849+t3968+t3972-t5255+t17.*(t260+t468+t570+t2298).*7.35522e-1).*(-1.0./4.0);
t15330 = -t15327;
t15379 = -t15378;
t15383 = (t10753.*t14213)./4.0;
t15384 = (t10763.*t14209)./4.0;
t15393 = (t10783.*t14209)./4.0;
t15395 = (t10787.*t14213)./4.0;
t15466 = -t15465;
t15472 = t14209.*(t3418-t3879+t4324-t5228+t5802+t9.*(t71-t391).*4.5305948634e-2+t17.*(t426-t581).*7.35522e-1).*(-1.0./4.0);
t15473 = (t11470.*t14209)./4.0;
t15475 = t14213.*(t3418-t3879+t4324-t5228+t5802+t9.*(t71-t391).*4.5305948634e-2+t17.*(t426-t581).*7.35522e-1).*(-1.0./4.0);
t15476 = (t11470.*t14213)./4.0;
t15478 = (t14213.*(t3418-t3879+t4324-t5228+t5802+t9.*(t71-t391).*4.5305948634e-2+t17.*(t426-t581).*7.35522e-1))./4.0;
t15479 = (t11484.*t14209)./4.0;
t15482 = -t15480;
t15483 = (t11483.*t14213)./4.0;
t15517 = -t15516;
t15523 = -t15522;
t15567 = -t15565;
t15569 = -t15566;
t15583 = -t15579;
t15868 = -t15867;
t15883 = -t15882;
t15886 = (t14209.*t14411)./4.0;
t15888 = (t14213.*t14413)./4.0;
t15903 = -t15901;
t15923 = -t15921;
t15924 = -t15922;
t15932 = (t14209.*t14879)./4.0;
t15939 = t14213.*(t13145+t17.*(t8963+t7.*(t5026+t5.*(t2959-t2967))).*7.35522e-1).*(-1.0./4.0);
t15941 = (t14213.*(t13145+t17.*(t8963+t7.*(t5026+t5.*(t2959-t2967))).*7.35522e-1))./4.0;
t15946 = t14209.*(t3471+t3796+t3914+t3942+t4358+t9.*(t258+t2289+t5392+t7559).*7.35522e-1+t17.*(t7693+t9904).*7.35522e-1).*(-1.0./4.0);
t15950 = (t14209.*(t3471+t3796+t3914+t3942+t4358+t9.*(t258+t2289+t5392+t7559).*7.35522e-1+t17.*(t7693+t9904).*7.35522e-1))./4.0;
t15952 = -t15949;
t15953 = t14213.*(t3543+t3820+t3911+t3949+t4360+t12067+t17.*(t258+t2289+t5392+t7559).*7.35522e-1).*(-1.0./4.0);
t15955 = (t14213.*(t3543+t3820+t3911+t3949+t4360+t12067+t17.*(t258+t2289+t5392+t7559).*7.35522e-1))./4.0;
t15957 = (t14213.*t14918)./4.0;
t15958 = (t14209.*t14919)./4.0;
t15981 = t14209.*(-t3823+t3970+t11861+t8.*t11864+t972.*(t71-t391)+t2777.*(t71-t391)).*(-1.0./4.0);
t15984 = (t14209.*(-t3823+t3970+t11861+t8.*t11864+t972.*(t71-t391)+t2777.*(t71-t391)))./4.0;
t15986 = (t14213.*t15088)./4.0;
t15991 = (t14209.*t15156)./4.0;
t15992 = (t14213.*t15155)./4.0;
t15994 = t13357.*(t2091+t2497+t2579+t2680+t3516+t9.*(t210+t2107+t7423+t9121)+t17.*(t9166-t11658)).*(-1.0./4.0);
t15995 = (t13357.*(t2091+t2497+t2579+t2680+t3516+t9.*(t210+t2107+t7423+t9121)+t17.*(t9166-t11658)))./4.0;
t15998 = t13371.*(t2091+t2497+t2579+t2680+t3516+t9.*(t210+t2107+t7423+t9121)+t17.*(t9166-t11658)).*(-1.0./4.0);
t15999 = (t13371.*(t2091+t2497+t2579+t2680+t3516+t9.*(t210+t2107+t7423+t9121)+t17.*(t9166-t11658)))./4.0;
t16016 = t13172.*(t3418-t3879+t4324+t11855+t9.*(t71-t391).*4.5305948634e-2+t17.*(t426-t581).*7.35522e-1+t9.*(t9166-t11658).*7.35522e-1).*(-1.0./4.0);
t16018 = (t13172.*(t3418-t3879+t4324+t11855+t9.*(t71-t391).*4.5305948634e-2+t17.*(t426-t581).*7.35522e-1+t9.*(t9166-t11658).*7.35522e-1))./4.0;
t16021 = t13178.*(t3418-t3879+t4324+t11855+t9.*(t71-t391).*4.5305948634e-2+t17.*(t426-t581).*7.35522e-1+t9.*(t9166-t11658).*7.35522e-1).*(-1.0./4.0);
t16037 = t14209.*(t4324+t11855+t9.*(t71-t391).*4.5305948634e-2+t17.*(t426-t581).*7.35522e-1+t9.*(t9166-t11658).*7.35522e-1).*(-1.0./4.0);
t16038 = t14213.*(t3845+t3925+t4339+t9.*(t210+t2107+t7423+t9121).*7.35522e-1+t17.*(t9166-t11658).*7.35522e-1).*(-1.0./4.0);
t16039 = (t14209.*(t4324+t11855+t9.*(t71-t391).*4.5305948634e-2+t17.*(t426-t581).*7.35522e-1+t9.*(t9166-t11658).*7.35522e-1))./4.0;
t16065 = t14209.*(t3423+t3845+t3888+t3925+t4339+t9.*(t210+t2107+t7423+t9121).*7.35522e-1+t17.*(t9166-t11658).*7.35522e-1).*(-1.0./4.0);
t16066 = t14209.*(t3418-t3879+t4324+t11855+t9.*(t71-t391).*4.5305948634e-2+t17.*(t426-t581).*7.35522e-1+t9.*(t9166-t11658).*7.35522e-1).*(-1.0./4.0);
t16067 = t14213.*(t3423+t3845+t3888+t3925+t4339+t9.*(t210+t2107+t7423+t9121).*7.35522e-1+t17.*(t9166-t11658).*7.35522e-1).*(-1.0./4.0);
t16068 = t14213.*(t3418-t3879+t4324+t11855+t9.*(t71-t391).*4.5305948634e-2+t17.*(t426-t581).*7.35522e-1+t9.*(t9166-t11658).*7.35522e-1).*(-1.0./4.0);
t16069 = (t14213.*(t3423+t3845+t3888+t3925+t4339+t9.*(t210+t2107+t7423+t9121).*7.35522e-1+t17.*(t9166-t11658).*7.35522e-1))./4.0;
t16070 = t12494+t12498+t12750+t12769;
t16071 = t12495+t12497+t12750+t12769;
t16075 = t16073.*yd;
t16146 = t4446+t4631+t4668+t4758+t4796+t5004+t5033+t5186+t5242+t5249+t5260+t6377+t6404+t7125+t7190+t8614+t8666+t9074+t9268+t9882+t9885+t10307+t10601+t10606+t10707+t10708+t11438+t11702+t11703;
t16147 = -q1d.*(-t4446-t4631-t4668-t4758+t4796+t5014+t5186+t5242+t5249+t5260-t6377+t6390+t7125+t7190+t8614+t8666+t9074+t9268+t9882+t9885+t10307+t10601+t10606+t10707+t10708+t11438+t11702+t11703+t9.*(t348-t525).*8.36241330891889e-4);
t16157 = t4001+t4040+t4652+t4658+t4762+t4785+t4804+t4840+t5267+t5296+t5649+t5661+t5698+t5701+t5773+t5803+t7148+t7195+t7207+t8626+t8682+t8881+t9257+t10321+t10578+t10599+t10855+t10857+t10965+t10979+t11452+t11827+t11828;
t16158 = -q1d.*(-t4652-t4658+t4757+t4840+t5267+t5296+t5687-t5698+t5773+t5803+t7148+t7195+t7207+t8626+t8682+t8881+t9257+t10321+t10578+t10599+t10855+t10857+t10965+t10979+t11452+t11827+t11828+t9.*(t260+t468+t570+t2298).*3.867742437e-3+t17.*(t260+t468+t570+t2298).*1.563719772e-3+t2963.*(t71-t391)+t3167.*(t71-t391)+t4080.*(t71-t391)+t4130.*(t71-t391));
t16164 = t4407+t4421+t4425+t4429+t4481+t4483+t4903+t4904+t5100+t5108+t5590+t5596+t6030+t6420+t6486+t6964+t7008+t7213+t7269+t7308+t8685+t8735+t10133+t10713+t11203+t11464+t11472+t11599+t11614+t11879+t11882+t11916+t12120+t12121;
t16170 = t6599+t6875+t6901+t7556+t8004+t8135+t8212+t8251+t9009+t9011+t9036+t10719+t11180+t11182+t11436+t11532+t11534+t12117+t12560+t13037+t13042+t13206+t13212;
t16172 = t4279+t4301+t4305+t4485+t4490+t4518+t4805+t4821+t5206+t5225+t5813+t5844+t6392+t6620+t6696+t7394+t7411+t7474+t7814+t7899+t8762+t8866+t10388+t10784+t11345+t12017+t12040+t12044+t12137+t12156+t12298+t12301+t12417+t12428;
t16177 = t4484+t4576+t4580+t4749+t4773+t4786+t5002+t5030+t5643+t5658+t6384+t6387+t6965+t7270+t7384+t7472+t7744+t7785+t8540+t8593+t9007+t9038+t11218+t11617+t11933+t12186+t12640+t12645+t12754+t12758+t12895+t12902+t12988+t12989;
t16178 = t4503+t4613+t4616+t4732+t4747+t4759+t5010+t5023+t5659+t5674+t6367+t6402+t6965+t7270+t7384+t7472+t7744+t7785+t8540+t8593+t9007+t9038+t11218+t11617+t11933+t12186+t12640+t12645+t12754+t12758+t12895+t12902+t12988+t12989;
t16207 = q1d.*t16206;
t16222 = t4238+t4275+t4310+t4456+t4682+t4725+t4740+t4754+t4769+t4770+t4956+t4962+t5315+t5318+t5347+t5376+t5666+t5685+t5765+t5801+t6341+t6380+t6996+t7011+t7111+t7501+t7568+t7576+t7588+t7870+t7871+t8071+t8630+t8641+t8681+t8715+t8926+t8938+t8941+t8944+t9153+t9186+t9664+t9694+t9696+t10005+t10006+t10017+t10118+t10124+t10338+t10499+t10511+t10515+t10757+t10762+t10808+t11289+t11294+t11456+t11998+t12000;
t16223 = -q1d.*(-t4238+t4295-t4456+t4713+t4744+t4783+t4797+t4947+t5325+t5330+t5336+t5390-t5666+t5675+t5749+t5814+t6360+t6396+t7007+t7031+t7103+t7491+t7572+t7583+t7859+t7884+t8090+t8624+t8648+t8676+t8721+t8929+t8935+t8936+t8947+t9148+t9180+t9653+t9689-t10006+t10009+t10011+t10121+t10130+t10329+t10497+t10518+t10522+t10756-t10808+t11280+t11285+t11454+t11992+t11996+(t9.*(t578.*4.28e-4+t2566-t2597+t905.*(t71-t391)+t1021.*(t71-t391)))./4.0+t17.*(-t3823+t3970+t5243+t9.*(t260+t468+t570+t2298).*7.35522e-1+t972.*(t71-t391)+t2777.*(t71-t391)).*1.539925e-2+t8.*(t71-t391).*5.187945860934245e-5+t16.*(t71-t391).*4.67845486573025e-5+(t2522.*(t689-t740))./4.0+t17.*(-t2550+t2696+t2698+t4771+t9.*(t260+t468+t570+t2298)+t147.*(t71-t391)).*1.13264871585e-2+(t16.*t3286.*(t71-t391))./4.0);
t16224 = t4238+t4295+t4310+t4456+t4713+t4725+t4740+t4744+t4783+t4797+t4956+t4962+t5325+t5330+t5336+t5390+t5666+t5685+t5749+t5814+t6360+t6396+t7007+t7031+t7103+t7501+t7572+t7576+t7583+t7859+t7884+t8090+t8624+t8648+t8676+t8721+t8929+t8935+t8936+t8947+t9148+t9180+t9653+t9694+t9696+t10006+t10009+t10011+t10121+t10130+t10329+t10497+t10518+t10522+t10757+t10762+t10808+t11280+t11285+t11454+t11992+t11996;
t16228 = t4831+t5358+t5377+t5506+t5767+t5926+t5959+t6083+t6860+t6962+t7012+t7072+t7107+t7324+t7380+t7708+t7725+t7907+t7942+t8074+t8098+t8333+t8355+t8629+t8815+t8961+t8990+t9054+t9079+t9089+t9736+t10394+t10429+t10779+t10799+t11327+t11329+t11457+t11481+t11486+t11821+t12642+t12775+t13413+t13415+t13418+t13421;
t16244 = t3953+t4000+t4369+t4379+t4412+t4427+t4435+t4440+t4492+t4808+t4846+t4921+t4940+t5074+t5099+t5348+t5366+t5411+t5798+t5908+t6345+t6395+t6405+t6521+t6541+t6565+t7045+t7150+t7198+t7595+t7599+t8021+t8164+t8602+t8637+t8656+t8687+t8903+t9193+t9284+t9290+t9321+t9334+t9532+t9555+t9714+t9751+t9840+t10179+t10194+t10430+t10517+t10672+t10835+t10885+t10894+t10915+t11011+t11014+t11132+t11142+t11560+t11647+t11656+t12092+t12099;
t16246 = q1d.*t16245;
t16247 = t3629+t3663+t3770+t4422+t4525+t4674+t4812+t4968+t5087+t5101+t5288+t5500+t5510+t5896+t5946+t6123+t6124+t6246+t6260+t6362+t6406+t6948+t7038+t7050+t7350+t7450+t7579+t7581+t7627+t7673+t7788+t7971+t8014+t8020+t8040+t8469+t8722+t8777+t8891+t9042+t9080+t10294+t10295+t10484+t10507+t10738+t10770+t11752+t11761+t11770+t11782+t11786+t11792+t12841+t12843+t13434+t13435+t13444+t13445;
t16249 = t4226+t4231+t4233+t4242+t4269+t4303+t4309+t4452+t4460+t4893+t4902+t5194+t5221+t5736+t6031+t6048+t6325+t6363+t6480+t6482+t6550+t6587+t6670+t6740+t7160+t7232+t7346+t7364+t7382+t7448+t7755+t7783+t7873+t7938+t8698+t8701+t8763+t9649+t9793+t9818+t9823+t9837+t9842+t9843+t9936+t9955+t9964+t10106+t10266+t10552+t10570+t10724+t10880+t10884+t10949+t10971+t11003+t11022+t11630+t11666+t11822+t11978+t11991+t12172+t12182+t12444+t12452;
t16250 = t4203+t4254+t4260+t4266+t4283+t4289+t4317+t4469+t4480+t4880+t4913+t5200+t5214+t5736+t6031+t6048+t6325+t6363+t6480+t6482+t6550+t6587+t6670+t6740+t7160+t7232+t7346+t7364+t7382+t7448+t7755+t7783+t7861+t7950+t8698+t8701+t8763+t9649+t9810+t9818+t9823+t9824+t9842+t9843+t9941+t9955+t9964+t10106+t10266+t10552+t10570+t10724+t10880+t10888+t10953+t10961+t11003+t11022+t11630+t11666+t11822+t11978+t11991+t12172+t12182+t12444+t12452;
t16252 = t559+t568+t2420+t2424+t4026+t4032+t4549+t4563+t4638+t4673+t5320+t5321+t5341+t5378+t5895+t5897+t6074+t6101+t6102+t6111+t6137+t6138+t6145+t6146+t6987+t7068+t7073+t7092+t7094+t7152+t7860+t7951+t8026+t8027+t8250+t8264+t8274+t8289+t8499+t8500+t8508+t8509+t9014+t9026+t9160+t9162+t9205+t9208+t10376+t10377+t11161+t11162+t11192+t11195+t12032+t12033+t12045+t12048+t12059+t12060+t13149+t13151+t13860+t13866+t13867+t13868;
t16267 = q1d.*t16266;
t16294 = t3909+t3938+t3951+t4005+t4089+t4146+t4154+t4166+t4246+t4257+t4307+t4325+t4454+t4458+t4463+t4523+t5019+t5071+t5129+t5136+t5202+t5342+t5369+t5473+t5512+t5549+t5676+t6228+t6321+t6328+t6354+t6553+t6664+t6692+t6702+t6708+t6714+t6757+t6764+t6775+t6944+t7046+t7510+t7582+t7594+t7615+t7696+t7722+t7742+t7752+t7916+t7961+t7974+t8037+t8076+t8078+t8196+t8417+t8449+t8451+t8655+t8686+t8730+t8748+t8788+t9037+t9039+t9304+t9305+t9326+t9351+t9365+t9543+t9548+t9581+t9595+t9607+t9692+t9706+t9716+t10381+t10400+t10493+t10503+t10576+t10667+t11245+t11261+t11450+t11460+t11479+t11482+t11501+t11509+t11675+t12011+t12085+t12088+t12285+t12290;
t16298 = t3909+t3926+t3967+t3977+t4089+t4146+t4166+t4193+t4215+t4257+t4315+t4342+t4430+t4438+t4478+t4552+t5019+t5071+t5129+t5136+t5223+t5342+t5369+t5492+t5519+t5549+t5676+t6228+t6321+t6328+t6354+t6553+t6664+t6692+t6702+t6725+t6731+t6757+t6764+t6775+t6944+t7046+t7510+t7582+t7594+t7615+t7696+t7702+t7752+t7754+t7916+t7961+t7974+t8049+t8076+t8097+t8176+t8417+t8449+t8451+t8655+t8686+t8730+t8756+t8788+t9034+t9040+t9304+t9305+t9326+t9351+t9365+t9543+t9548+t9581+t9595+t9598+t9698+t9706+t9716+t10381+t10400+t10495+t10509+t10576+t10646+t11252+t11271+t11450+t11460+t11479+t11482+t11501+t11509+t11675+t12011+t12085+t12088+t12285+t12290;
t16314 = t6599+t6875+t6901+t7556+t8004+t8135+t8212+t8251+t9009+t9011+t9036+t13794+t14048+t15812+t15814+t15839+t15841+t15875+t15890+t16052+t16054+t16055+t16057;
t16317 = t3193+t3197+t3929+t3935+t3975+t3984+t4039+t4053+t4109+t4131+t4172+t4179+t4222+t4263+t4276+t4311+t4377+t4982+t5057+t5090+t5143+t5417+t5425+t5444+t5493+t5584+t5686+t5752+t6252+t6344+t6401+t6428+t6443+t6459+t6639+t6748+t6779+t7082+t7093+t7096+t7158+t7164+t7514+t7551+t7574+t7617+t7647+t7650+t7767+t7838+t7892+t7902+t7948+t7973+t8138+t8342+t8377+t8422+t8668+t8700+t8707+t8761+t8778+t8800+t8958+t8989+t9044+t9047+t9342+t9604+t9606+t9715+t9841+t9856+t9857+t9869+t9880+t9881+t9961+t9963+t9966+t10105+t10259+t10268+t10536+t10544+t10560+t10564+t10780+t10881+t11306+t11321+t11498+t11689+t11897+t12062+t12069+t12112+t12201+t12206+t12383+t12384+t12475+t12481;
t16328 = t3806+t3818+t3974+t3983+t4108+t4155+t4171+t4184+t4245+t4316+t4343+t4431+t4439+t4766+t4803+t5368+t5513+t5566+t5647+t5717+t5754+t5775+t5799+t5805+t6078+t6177+t6254+t6370+t6418+t6424+t6549+t6555+t6920+t7014+t7136+t7201+t7214+t7353+t7592+t7616+t7691+t7723+t7802+t7827+t7829+t7890+t7914+t8181+t8241+t8369+t8396+t8611+t8625+t8664+t8720+t8901+t8932+t8965+t9000+t9192+t9297+t9352+t9679+t9682+t9894+t9903+t9931+t9933+t9945+t9969+t9990+t10015+t10281+t10355+t10375+t10516+t10725+t10751+t10765+t10791+t10801+t10805+t11035+t11060+t11073+t11112+t11133+t11134+t11302+t11310+t11411+t12001+t12003+t12356+t12409+t12460+t12493+t12683+t12688+t12817+t12818+t12823+t12824+t12942+t12946;
t16329 = t3782+t3792+t3959+t3997+t4139+t4143+t4194+t4214+t4217+t4308+t4326+t4455+t4464+t4779+t4795+t5356+t5513+t5566+t5647+t5727+t5754+t5775+t5789+t5805+t6078+t6177+t6254+t6370+t6418+t6424+t6549+t6555+t6920+t7014+t7136+t7201+t7214+t7353+t7605+t7635+t7691+t7723+t7802+t7827+t7829+t7890+t7914+t8181+t8241+t8369+t8396+t8617+t8631+t8669+t8720+t8919+t8932+t8953+t9000+t9198+t9297+t9352+t9679+t9682+t9894+t9903+t9931+t9933+t9945+t9969+t9998+t10007+t10286+t10355+t10375+t10523+t10725+t10751+t10765+t10791+t10801+t10805+t11035+t11060+t11073+t11112+t11133+t11134+t11307+t11320+t11421+t12009+t12010+t12356+t12409+t12460+t12493+t12683+t12688+t12817+t12818+t12823+t12824+t12942+t12946;
t16340 = t2321+t2334+t2385+t2884+t2885+t3332+t3401+t3647+t3769+t3891+t3927+t3969+t3987+t4530+t4854+t4856+t4881+t4910+t4937+t4997+t5017+t5133+t5173+t5239+t5339+t5410+t5420+t5499+t5606+t5631+t5637+t5655+t5683+t5731+t5880+t5936+t6013+t6151+t6202+t6349+t6361+t6458+t6509+t6559+t6583+t6616+t6644+t6649+t6663+t6701+t6726+t6733+t6749+t6772+t6787+t6818+t6905+t6953+t7048+t7112+t7126+t7186+t7216+t7289+t7326+t7442+t7488+t7496+t7533+t7569+t7756+t7769+t7809+t7919+t7969+t8051+t8091+t8151+t8291+t8299+t8316+t8440+t8675+t8692+t8699+t8785+t8887+t8896+t8937+t9041+t9096+t9117+t9120+t9149+t9201+t9349+t9597+t9615+t9703+t9719+t9948+t9949+t10014+t10053+t10068+t10075+t10155+t10351+t10354+t10504+t10505+t10616+t10775+t10778+t11141+t11353+t11381+t11520+t11536+t11556+t11568+t11816+t11820+t11924+t12130+t12227+t12229+t12233+t12237+t12580+t12581+t12583+t12584;
t16342 = q1d.*t16341;
t16347 = -xd.*(t7036+t7056-t7658+t8022+t8678-t9347+t9360-t9412+t9775+t9813+t10020+t10022+t10025+t10043+t10371+t10528+t10968+t11177-t11186+t11351-t11367+t11698+t11946+t11949+t12105-t12129-t12135+t12144+t12165+t12370-t12408-t12416-t12471+t12830-t12870-t13041-t13200-t13283-t13653-t13873+t13877+t13950+t13951+t14135+t14141+t14176-t14177+t14738+t14995+(t6677.*(t10158+t16.*(t4542-t6448)))./4.0+(t6540.*(t10403+t9.*(t10158+t16.*(t4542-t6448)).*7.35522e-1))./4.0+(t536.*(t5122+t5.*(t2425-t2468).*3.587895))./4.0+((t923-t1076).*(t5110-t6808))./4.0+((t2812-t2860).*(t4542-t6448))./4.0+(t5050.*(t10384+t16.*(t4542-t6448).*1.666555))./4.0+(t9048.*(t10174+t9.*(t10158+t16.*(t4542-t6448))))./4.0+t15.*t4286.*(t4542-t6448).*3.064865e-1+(t15.*t6196.*(t4542-t6448))./4.0);
t16353 = phid.*t16352;
t16354 = t4238+t4275+t4310+t4456+t4682+t4725+t4740+t4754+t4769+t4770+t4956+t4962+t5315+t5318+t5347+t5376+t5765+t5801+t6341+t6380+t6996+t7011+t7111+t7501+t7568+t7576+t7588+t8071+t8630+t8641+t8681+t8715+t12002+t12007+t13114+t13433+t13692+t13853+t14031+t14032+t14192+t14193+t14204+t14208+t14254+t14350+t14462+t14463+t14476+t14481+t14557+t14588+t14589+t14873+t14895+t14896+t15140+t15141+t15618+t15621+t15688+t15691;
t16358 = t2320+t2333+t2384+t3029+t3288+t3303+t3305+t3351+t3761+t4007+t4008+t4048+t4164+t4338+t4556+t4877+t4955+t4985+t5098+t5102+t5269+t5340+t5367+t5375+t5406+t5529+t5660+t5757+t5762+t5800+t5891+t5997+t6079+t6156+t6307+t6463+t6571+t6648+t6660+t6676+t6700+t6770+t6821+t6867+t6871+t6891+t6909+t6947+t6998+t7006+t7101+t7102+t7234+t7255+t7265+t7266+t7268+t7312+t7365+t7564+t7571+t7580+t7626+t7664+t7694+t7718+t7810+t7836+t7885+t7910+t7972+t8018+t8139+t8335+t8376+t8384+t8429+t8575+t8639+t8657+t8684+t8718+t8731+t8807+t8898+t8951+t8991+t9313+t9536+t9568+t9570+t9572+t9584+t9640+t9658+t9710+t9725+t9910+t9925+t9987+t10026+t10241+t10244+t10450+t10465+t10614+t10816+t10830+t10883+t10923+t10937+t10975+t10999+t11037+t11113+t11120+t11265+t11420+t11849+t12019+t12145+t12152+t12215+t12352+t12357+t12367+t12374+t12457+t12838+t12839+t12857+t12858+t12994+t12999+t13000+t13001;
t16359 = q1d.*t16357;
t16372 = t4831+t5358+t5377+t5506+t5767+t5926+t5959+t6083+t6962+t7012+t7072+t7107+t7324+t7380+t7725+t8074+t8098+t8629+t8815+t8961+t8990+t9054+t9089+t9863+t10700+t13242+t13256+t13341+t13360+t13651+t13945+t14568+t14574+t14660+t14670+t14870+t14970+t15709+t15710+t15723+t15725+t15818+t15835+t16086+t16088+t16089+t16090;
t16374 = t7903+t8015+t8017+t8302+t8327+t8442+t8445+t8486+t8502+t8620+t9033+t9035+t10868+t10873+t10906+t11231+t11237+t11993+t12551+t12554+t12948+t13016+t13023+t13545+t14571+t14577+t14681+t14838+t14845+t14977+t15685+t15687+t15745+t15747+t15752+t15810+t16077+t16078+t16094+t16095;
t16376 = t4379+t4397+t4412+t4427+t4435+t4440+t4492+t4826+t4836+t4921+t4940+t5338+t5379+t5403+t5811+t5893+t6326+t6378+t6416+t6528+t6532+t6575+t7027+t7140+t7189+t7610+t7619+t8021+t8164+t8580+t8645+t8663+t8691+t8880+t9611+t9619+t9979+t9989+t13123+t13703+t13855+t14099+t14287+t14288+t14290+t14291+t14326+t14330+t14506+t14507+t14580+t14654+t14665+t14696+t14724+t14730+t14731+t14760+t14769+t14907+t14972+t14975+t15660+t15661+t15704+t15706;
t16378 = t4397+t4399+t4408+t4414+t4416+t4433+t4468+t4826+t4836+t4935+t4950+t5338+t5379+t5403+t5811+t5893+t6326+t6378+t6416+t6528+t6532+t6575+t7027+t7140+t7189+t7610+t7619+t8005+t8150+t8580+t8645+t8663+t8691+t8880+t9621+t9628+t9982+t9985+t13123+t13703+t13857+t14101+t14287+t14288+t14290+t14291+t14326+t14330+t14506+t14507+t14580+t14656+t14662+t14696+t14724+t14730+t14731+t14760+t14769+t14907+t14973+t14974+t15660+t15661+t15704+t15706;
t16379 = t4231+t4233+t4242+t4303+t4309+t4452+t4460+t4893+t4902+t5736+t6031+t6048+t6325+t6363+t6480+t6482+t6550+t6587+t6670+t6740+t7160+t7232+t7346+t7364+t7382+t7448+t7755+t7783+t7873+t7938+t8501+t8507+t8698+t8701+t8763+t9649+t10106+t10940+t10954+t13593+t13891+t13975+t14189+t14399+t14402+t14407+t14408+t14438+t14445+t14623+t14629+t14642+t14722+t14734+t14921+t14927+t14928+t14932+t14971+t15009+t15019+t15220+t15225+t15719+t15721+t15759+t15761;
t16380 = t4203+t4260+t4266+t4283+t4317+t4469+t4480+t4880+t4913+t5736+t6031+t6048+t6325+t6363+t6480+t6482+t6550+t6587+t6670+t6740+t7160+t7232+t7346+t7364+t7382+t7448+t7755+t7783+t7861+t7950+t8510+t8520+t8698+t8701+t8763+t9649+t10106+t10946+t10950+t13593+t13895+t13975+t14191+t14399+t14402+t14407+t14408+t14438+t14445+t14623+t14629+t14642+t14722+t14734+t14921+t14926+t14930+t14932+t14971+t15009+t15019+t15221+t15223+t15719+t15721+t15759+t15761;
t16386 = t6599+t6875+t6901+t7556+t8004+t8135+t8212+t8251+t9009+t9011+t9036+t9397+t9432+t10720+t11378+t11382+t11437+t13490+t13600+t13795+t14049+t14790+t14793+t14795+t14799+t14883+t14889+t14897+t14898+t14901+t14902+t14949+t14955+t15101+t15112+t15256+t15257+t15434+t15440+t15453+t15457+t15808+t15811+t15819+t15821;
t16392 = phid.*t16391;
t16394 = phid.*t16393;
t16395 = t4232+t4409+t4413+t4417+t4698+t4715+t4813+t5184+t5238+t6075+t6379+t6394+t6485+t6572+t6618+t6635+t7123+t7183+t7243+t7432+t7449+t7565+t7640+t7921+t7941+t8134+t8184+t8284+t8528+t8542+t8579+t8659+t8767+t8814+t8909+t10120+t10287+t10300+t10856+t13638+t13698+t14012+t14077+t14644+t14646+t14650+t14652+t14674+t14679+t14742+t14743+t14763+t14768+t14882+t14950+t14962+t14965+t15081+t15132+t15197+t15199+t15267+t15268+t15771+t15776+t15790+t15792;
t16397 = t4259+t4380+t4434+t4441+t4663+t4685+t4794+t5160+t5245+t6075+t6379+t6394+t6485+t6572+t6618+t6635+t7123+t7183+t7243+t7432+t7449+t7565+t7640+t7921+t7941+t8134+t8184+t8284+t8544+t8549+t8601+t8652+t8767+t8814+t8909+t10120+t10293+t10298+t10856+t13638+t13702+t14012+t14082+t14643+t14647+t14650+t14652+t14674+t14679+t14742+t14743+t14763+t14768+t14882+t14950+t14963+t14964+t15081+t15132+t15197+t15199+t15267+t15268+t15771+t15776+t15790+t15792;
t16398 = t2886+t3390+t3442+t3518+t3568+t3602+t3605+t3642+t3707+t3844+t4095+t4100+t4148+t4224+t4241+t4293+t4294+t4296+t4497+t4606+t4626+t4665+t4736+t4742+t4834+t4901+t4911+t4963+t4998+t5088+t5093+t5222+t5278+t5469+t5480+t5525+t5526+t5667+t5669+t5873+t5881+t5890+t5998+t6026+t6053+t6054+t6065+t6071+t6072+t6088+t6118+t6120+t6153+t6179+t6186+t6192+t6231+t6305+t6585+t6594+t6669+t6728+t6755+t6894+t6946+t6992+t6993+t7001+t7002+t7015+t7059+t7179+t7184+t7208+t7238+t7239+t7302+t7317+t7349+t7403+t7406+t7421+t7463+t7465+t7478+t7499+t7607+t7712+t7747+t7787+t7793+t7898+t7904+t7923+t7930+t7946+t7953+t8087+t8157+t8197+t8322+t8345+t8456+t8493+t8503+t8607+t8695+t8727+t8832+t8840+t9006+t9030+t9311+t9381+t9428+t9860+t9872+t9898+t9902+t10086+t10109+t10110+t10116+t10196+t10197+t10385+t10420+t10426+t10456+t10605+t10659+t10814+t10819+t10860+t11206+t11213+t11224+t11249+t11250+t11273+t11274+t11600+t11606+t11618+t11621+t11636+t11644+t11912+t12140+t12418+t12419+t12634+t12637+t12650+t12658+t12660+t12661+t12871+t12872+t12878+t12884+t13296+t13297+t13299+t13303;
t16400 = t2987+t3390+t3442+t3518+t3568+t3602+t3605+t3679+t3707+t3892+t4100+t4115+t4126+t4224+t4264+t4293+t4294+t4296+t4497+t4606+t4626+t4665+t4736+t4742+t4834+t4898+t4901+t4972+t5018+t5088+t5093+t5237+t5278+t5469+t5480+t5525+t5526+t5653+t5680+t5873+t5890+t5892+t5998+t6043+t6053+t6054+t6065+t6071+t6072+t6088+t6118+t6120+t6153+t6179+t6186+t6192+t6231+t6291+t6584+t6596+t6678+t6741+t6745+t6894+t6946+t6992+t6993+t7001+t7002+t7015+t7059+t7179+t7184+t7208+t7239+t7250+t7293+t7323+t7349+t7403+t7406+t7410+t7463+t7465+t7478+t7499+t7593+t7712+t7757+t7801+t7811+t7878+t7904+t7923+t7930+t7946+t7953+t8067+t8157+t8197+t8322+t8345+t8456+t8493+t8503+t8607+t8703+t8732+t8832+t8858+t9006+t9030+t9302+t9394+t9408+t9860+t9872+t9898+t9902+t10101+t10109+t10110+t10112+t10196+t10197+t10385+t10426+t10428+t10464+t10605+t10659+t10815+t10824+t10865+t11206+t11213+t11233+t11249+t11250+t11273+t11274+t11600+t11606+t11618+t11621+t11636+t11644+t11921+t12148+t12418+t12419+t12634+t12637+t12652+t12668+t12672+t12673+t12871+t12872+t12878+t12884+t13296+t13297+t13299+t13303;
t16426 = t3909+t4005+t4089+t4146+t4154+t4166+t4246+t4257+t4307+t4325+t4454+t4458+t4463+t4523+t5019+t5071+t5129+t5136+t5202+t5342+t5369+t5473+t5512+t5549+t5676+t6228+t6321+t6328+t6354+t6553+t6664+t6692+t6702+t6708+t6714+t6757+t6944+t7046+t7510+t7582+t7594+t7615+t7696+t7752+t7974+t8037+t8078+t8196+t8417+t8655+t8686+t8730+t9599+t9605+t11366+t11735+t12257+t12295+t12364+t12371+t12582+t12591+t12747+t12753+t12901+t13126+t13129+t13164+t13165+t13170+t13173+t13202+t13203+t13234+t13237+t13512+t13515+t13722+t13750+t14073+t14087+t14100+t14377+t14382+t14570+t14573+t14860+t14864+t14942+t15024+t15061+t15064+t15340+t15341+t15348+t15349+t15700+t15703+t15726+t15729;
t16429 = t3929+t3935+t4039+t4053+t4109+t4131+t4172+t4179+t4222+t4263+t4276+t4311+t4377+t4982+t5057+t5090+t5143+t5417+t5425+t5444+t5493+t5584+t5686+t5752+t6252+t6344+t6401+t6428+t6443+t6459+t6639+t6748+t6779+t7082+t7093+t7096+t7158+t7164+t7514+t7551+t7574+t7617+t7647+t7650+t7767+t7838+t7892+t7902+t7948+t7973+t8228+t8236+t8394+t8412+t8422+t8668+t8707+t8761+t11399+t12275+t12377+t12894+t12900+t12943+t12955+t13002+t13032+t13035+t13219+t13231+t13338+t13339+t13340+t13344+t13349+t13351+t13412+t13591+t13594+t13734+t13738+t13828+t13847+t14096+t14148+t14187+t14439+t14440+t14622+t14624+t14986+t15098+t15120+t15121+t15269+t15270+t15445+t15450+t15460+t15463+t15741+t15742+t15762+t15763;
t16432 = t5871+t5932+t6011+t6547+t6771+t6825+t7106+t7173+t7872+t7979+t7989+t8042+t8045+t8234+t8523+t8627+t8915+t9073+t9097+t9364+t9383+t9580+t10145+t11824+t11834+t12218+t12604+t13210+t13216+t13321+t13323+t13464+t13483+t13605+t13606+t13619+t13620+t13817+t13818+t13839+t13840+t14019+t14020+t14023+t14025+t14104+t14105+t14106+t14107+t14640+t14694+t14812+t14815+t14905+t14909+t15020+t15022+t15067+t15071+t15370+t15398+t15649+t15651+t15667+t15668+t15837+t15838+t15844+t15846;
t16440 = t4108+t4155+t4171+t4184+t4245+t4316+t4343+t4431+t4439+t4766+t4803+t5368+t5513+t5566+t5647+t5717+t5754+t5775+t5799+t5805+t6078+t6177+t6254+t6370+t6383+t6391+t6418+t6424+t6549+t6555+t6920+t7014+t7136+t7201+t7214+t7353+t7592+t7616+t7691+t7723+t7802+t7827+t7829+t7890+t7914+t8181+t8241+t8369+t8396+t8432+t8436+t8611+t8625+t8664+t8720+t8932+t9000+t9297+t9933+t12038+t12097+t12535+t12692+t12954+t12980+t13288+t13290+t13363+t13368+t13399+t13408+t13451+t13462+t13610+t13623+t13632+t13791+t13822+t13829+t13851+t13982+t13996+t13997+t14006+t14069+t14395+t14457+t14676+t14683+t14767+t14776+t14853+t14856+t15044+t15045+t15196+t15229+t15550+t15551+t15584+t15585+t15786+t15791+t15798+t15801;
t16442 = phid.*t16441;
t16443 = t4816+t5349+t5391+t5498+t5611+t5616+t5774+t5905+t5938+t6073+t6890+t6976+t7032+t7088+t7121+t7347+t7367+t7648+t7675+t7726+t7746+t8094+t8114+t8623+t8834+t8972+t8994+t9060+t9094+t9875+t9975+t10146+t10709+t11268+t11277+t11391+t11393+t11459+t11461+t11466+t11474+t11575+t11583+t11657+t11662+t11895+t11947+t12016+t12083+t12317+t12454+t12597+t12614+t12828+t12850+t13223+t13423+t13568+t13573+t13633+t13641+t13720+t13728+t13845+t13849+t13864+t14083+t14136+t14190+t14296+t14300+t14347+t14349+t14847+t14849+t14857+t14878+t14880+t14891+t15161+t15162+t15287+t15314+t15323+t15369+t15603+t15604+t15605+t15606+t15847+t15848+t15851+t15852;
t16445 = -phid.*(t4831+t5358+t5377+t5506+t5611+t5616+t5767+t5926+t5959+t6083+t6861+t6962+t7012+t7072+t7107+t7324+t7380+t7648+t7675+t7709+t7725+t8074+t8098+t8629+t8815+t8961+t8990+t9054+t9089+t9864+t9975+t10146+t10701-t11268+t11269+t11391+t11393+t11458-t11461+t11463-t11474+t11575+t11583+t11655-t11657+t11895+t12016-t12317-t12454-t12597+t12609-t12828+t12844+t13221+t13420+t13568+t13573-t13633+t13637+t13720+t13728-t13845+t13848+t13864+t14078+t14136+t14188-t14296+t14298-t14347+t14348-t14847-t14849-t14878-t14880+t15161+t15162+t15314+t15323-t15605-t15606+t15849+t15850+(t6190.*(-t1053-t3327+t5081.*1.225946+t7731+t15.*t223.*1.4653732538e-2))./4.0+(t14541.*(t3418-t3879+t4324-t5228+t5802+t9.*(t71-t391).*4.5305948634e-2+t17.*(t426-t581).*7.35522e-1))./4.0+(t9187.*(t3418-t3879+t4324+t11855+t9.*(t71-t391).*4.5305948634e-2+t17.*(t426-t581).*7.35522e-1+t9.*(t9166-t11658).*7.35522e-1))./4.0+(t14918.*(t1987-t2621+t3452-t4730+t5359+t9.*(t71-t391).*6.1597e-2+t17.*(t426-t581)))./4.0+(t13273.*(t1589-t2213+t3195-t4346+t4355+t4748.*7.35522e-1+t2772.*(t71-t391)+t2775.*(t71-t391)))./4.0+(t10501.*(t985+t3399-t13.*t42.*1.01140545e-1-t7.*t223.*5.034347249e-2))./4.0+(t8433.*(t1589-t2213-t4346+t4355+t9454+t11863+t2772.*(t71-t391)+t2775.*(t71-t391)))./4.0+(t13974.*(t249-t391.*(1.1e+1./1.25e+2)-t1912.*4.252e-3+t3505+t5357+t693.*(t71-t391)+t784.*(t71-t391)))./4.0+(t10096.*(t249-t391.*(1.1e+1./1.25e+2)-t1912.*4.252e-3+t3505+t13496+t693.*(t71-t391)+t784.*(t71-t391)))./4.0+(t10753.*(t1987-t2621+t3452+t11654+t9.*(t71-t391).*6.1597e-2+t17.*(t426-t581)+t9.*(t9166-t11658)))./4.0);
t16446 = t2262+t2305+t2385+t2884+t2885+t3332+t3401+t3647+t3769+t3891+t3927+t3969+t3987+t4530+t4854+t4856+t4881+t4910+t4937+t4997+t5017+t5133+t5173+t5239+t5339+t5606+t5631+t5655+t5731+t5880+t5936+t6013+t6151+t6202+t6349+t6361+t6458+t6509+t6559+t6583+t6616+t6644+t6701+t6733+t6787+t6818+t6905+t6953+t7048+t7112+t7126+t7216+t7442+t7488+t7533+t7569+t7756+t7769+t7809+t7845+t7847+t7919+t7969+t8051+t8091+t8291+t8316+t8440+t8699+t8785+t8887+t9083+t10150+t10166+t10269+t10276+t10437+t10524+t10810+t10912+t10930+t11207+t11215+t11221+t11335+t11409+t11650+t11676+t11811+t11826+t11961+t11979+t12276+t12378+t12379+t12483+t12655+t12662+t13052+t13060+t13083+t13436+t13446+t13732+t13742+t13743+t13841+t13844+t13908+t13909+t13959+t13964+t14011+t14303+t14304+t14360+t14364+t14562+t14565+t14664+t14669+t15003+t15117+t15351+t15354+t15357+t15361+t15375+t15376+t15400+t15401+t15766+t15768+t15774+t15775;
t16448 = phid.*t16447;
t16459 = t3629+t3663+t3770+t4422+t4525+t4674+t4812+t4968+t5288+t5896+t5900+t5902+t5934+t5937+t5946+t6125+t6126+t6260+t6362+t6406+t6948+t7038+t7050+t7350+t7627+t7673+t7788+t7971+t8014+t8105+t8455+t8469+t8492+t8710+t8722+t8777+t8891+t8934+t8969+t9042+t9080+t9126+t9139+t9366+t9380+t9384+t9393+t9496+t9583+t9602+t9650+t9661+t9940+t9965+t9974+t10143+t10214+t10224+t10411+t10425+t10537+t11117+t11121+t11502+t11504+t11977+t11986+t12029+t12037+t12173+t12188+t12354+t12566+t12695+t12730+t13199+t13218+t13307+t13314+t13664+t13694+t13736+t13737+t13813+t13842+t13885+t13886+t13930+t13939+t13991+t14171+t14174+t14175+t14417+t14420+t14422+t14425+t14929+t14933+t14960+t14961+t14968+t14969+t15294+t15307+t15381+t15389+t15454+t15458+t15675+t15677+t15679+t15680+t15853+t15854+t15857+t15858;
t16474 = t559+t568+t2420+t2424+t4026+t4032+t4549+t4563+t4638+t4673+t5322+t5323+t5341+t5378+t5550+t5895+t5897+t5933+t6074+t6111+t6530+t6960+t6987+t7068+t7073+t7092+t7094+t7152+t7261+t7860+t7951+t8057+t8073+t8081+t8082+t8120+t8146+t8152+t8250+t8264+t8274+t8289+t8467+t8468+t8475+t8478+t8522+t8526+t8537+t8745+t9014+t9026+t9160+t9162+t9205+t9208+t9367+t9426+t9451+t9627+t9912+t9915+t9952+t9957+t10335+t10346+t10404+t10729+t10740+t10766+t10807+t10859+t10864+t11519+t11524+t11530+t11762+t11763+t12080+t12250+t12329+t12331+t12532+t12602+t12648+t12654+t12755+t13124+t13125+t13142+t13143+t13183+t13635+t13639+t14015+t14016+t14021+t14024+t14053+t14064+t14224+t14267+t14271+t14272+t14273+t14276+t14277+t14281+t14286+t14534+t14835+t14839+t15039+t15047+t15049+t15050+t15444+t15447+t15477+t15480+t15571+t15575+t15595+t15596+t15598+t15599+t15876+t15877+t15880+t15881;
t16477 = phid.*t16476;
t13397 = -t13393;
t13478 = -t13476;
t13481 = t9.*t13362.*1.539925e-2;
t13503 = t9.*t13377.*1.539925e-2;
t13504 = -t13498;
t13672 = (t3738.*t13377)./4.0;
t13673 = -t13668;
t13769 = -t13764;
t13926 = (t5329.*t13362)./4.0;
t13934 = -t13928;
t13944 = (t5329.*t13377)./4.0;
t13948 = -t13946;
t14111 = -t14108;
t14114 = (t6811.*t13362)./4.0;
t14123 = -t14121;
t14137 = -t14134;
t14353 = t17.*t14297.*1.539925e-2;
t14354 = t9.*t14299.*1.539925e-2;
t14386 = -t14383;
t14388 = -t14385;
t14394 = -t14391;
t14398 = (t2054.*t14297)./4.0;
t14400 = (t2044.*t14299)./4.0;
t14412 = (t8979.*t13362)./4.0;
t14414 = -t14410;
t14418 = (t8979.*t13377)./4.0;
t14419 = -t14416;
t14464 = (t3738.*t14297)./4.0;
t14465 = (t3743.*t14297)./4.0;
t14466 = (t3738.*t14299)./4.0;
t14468 = (t3743.*t14299)./4.0;
t14470 = (t3767.*t14297)./4.0;
t14472 = (t3763.*t14299)./4.0;
t14516 = -t14514;
t14517 = -t14515;
t14521 = -t14518;
t14523 = -t14519;
t14524 = -t14520;
t14527 = -t14525;
t14528 = (t4474.*t14299)./4.0;
t14533 = (t4517.*t14297)./4.0;
t14545 = (t4772.*t14297)./4.0;
t14550 = (t4798.*t14299)./4.0;
t14595 = (t5217.*t14297)./4.0;
t14596 = (t5213.*t14299)./4.0;
t14627 = (t5329.*t14297)./4.0;
t14630 = (t5329.*t14299)./4.0;
t14631 = (t5345.*t14297)./4.0;
t14633 = (t5345.*t14299)./4.0;
t14639 = -t14636;
t14641 = -t14638;
t14658 = (t5679.*t14299)./4.0;
t14666 = (t5719.*t14297)./4.0;
t14671 = (t5760.*t14297)./4.0;
t14680 = (t5782.*t14299)./4.0;
t14698 = -t14697;
t14702 = -t14700;
t14704 = (t6016.*t14299)./4.0;
t14705 = (t6038.*t14297)./4.0;
t14706 = -t14703;
t14715 = -t14713;
t14729 = t13362.*(t1987-t2621+t3452-t4730+t5359+t9.*(t71-t391).*6.1597e-2+t17.*(t426-t581)).*(-1.0./4.0);
t14735 = t13377.*(t1987-t2621+t3452-t4730+t5359+t9.*(t71-t391).*6.1597e-2+t17.*(t426-t581)).*(-1.0./4.0);
t14745 = (t6526.*t14297)./4.0;
t14749 = (t6540.*t14299)./4.0;
t14783 = -t14780;
t14811 = (t6761.*t14297)./4.0;
t14816 = (t6761.*t14299)./4.0;
t14825 = (t6811.*t14297)./4.0;
t14826 = (t6811.*t14299)./4.0;
t14834 = -t14832;
t14840 = -t14836;
t14843 = -t14841;
t14844 = -t14842;
t14850 = -t14848;
t14874 = (t7348.*t14297)./4.0;
t14876 = t14299.*(t1468-t1988-t2498+t4565+t17.*(t208-t427)).*(-1.0./4.0);
t14877 = (t14299.*(t1468-t1988-t2498+t4565+t17.*(t208-t427)))./4.0;
t14908 = -t14906;
t14913 = -t14911;
t14931 = (t14297.*(t2056+t2203+t2351+t3433+t3503+t16.*t389.*(1.1e+1./1.25e+2)))./4.0;
t14936 = (t7799.*t14299)./4.0;
t14946 = (t7940.*t14297)./4.0;
t14951 = (t7949.*t14299)./4.0;
t14956 = (t7982.*t14297)./4.0;
t14958 = (t7987.*t14299)./4.0;
t15010 = -t15007;
t15011 = -t15008;
t15052 = -t15051;
t15055 = -t15053;
t15056 = -t15054;
t15057 = (t8725.*t14297)./4.0;
t15060 = -t15058;
t15062 = (t8743.*t14299)./4.0;
t15093 = (t8979.*t14297)./4.0;
t15094 = (t8981.*t14297)./4.0;
t15095 = -t15092;
t15096 = (t8979.*t14299)./4.0;
t15099 = (t8981.*t14299)./4.0;
t15109 = -t15102;
t15113 = (t9001.*t14297)./4.0;
t15114 = (t8999.*t14299)./4.0;
t15127 = -t15125;
t15148 = t14299.*(t824+t2543+t2699+t2707-t4767+t17.*(t260+t468+t570+t2298)).*(-1.0./4.0);
t15150 = t14297.*(-t2550+t2696+t2698+t4771+t9.*(t260+t468+t570+t2298)+t147.*(t71-t391)).*(-1.0./4.0);
t15151 = (t14297.*(-t2550+t2696+t2698+t4771+t9.*(t260+t468+t570+t2298)+t147.*(t71-t391)))./4.0;
t15152 = (t9187.*t14299)./4.0;
t15159 = (t9197.*t14297)./4.0;
t15169 = (t9233.*t14297)./4.0;
t15172 = (t9252.*t14299)./4.0;
t15181 = t14297.*(t3452-t4730+t5359+t9.*(t71-t391).*6.1597e-2+t17.*(t426-t581)).*(-1.0./4.0);
t15182 = (t9292.*t14299)./4.0;
t15183 = (t14297.*(t3452-t4730+t5359+t9.*(t71-t391).*6.1597e-2+t17.*(t426-t581)))./4.0;
t15190 = -t15189;
t15195 = -t15193;
t15204 = -t15202;
t15209 = -t15206;
t15297 = -t15293;
t15300 = -t15295;
t15301 = -t15296;
t15305 = -t15303;
t15306 = -t15304;
t15352 = (t10149.*t14297)./4.0;
t15355 = t14297.*(t1987-t2621+t3452-t4730+t5359+t9.*(t71-t391).*6.1597e-2+t17.*(t426-t581)).*(-1.0./4.0);
t15358 = (t10149.*t14299)./4.0;
t15362 = t14299.*(t1987-t2621+t3452-t4730+t5359+t9.*(t71-t391).*6.1597e-2+t17.*(t426-t581)).*(-1.0./4.0);
t15366 = (t14299.*(t1987-t2621+t3452-t4730+t5359+t9.*(t71-t391).*6.1597e-2+t17.*(t426-t581)))./4.0;
t15368 = (t10170.*t14299)./4.0;
t15371 = (t10180.*t14297)./4.0;
t15387 = -t15384;
t15397 = -t15395;
t15474 = -t15473;
t15484 = -t15483;
t15871 = (t14156.*t14297)./4.0;
t15873 = (t14161.*t14299)./4.0;
t15887 = -t15886;
t15889 = -t15888;
t15898 = t14297.*(t2189+t2495+t2635+t2646+t3580+t9.*(t258+t2289+t5392+t7559)+t17.*(t7693+t9904)).*(-1.0./4.0);
t15899 = (t14297.*(t2189+t2495+t2635+t2646+t3580+t9.*(t258+t2289+t5392+t7559)+t17.*(t7693+t9904)))./4.0;
t15900 = t14299.*(t2148+t2513+t2649+t2661+t3582+t11950+t17.*(t258+t2289+t5392+t7559)).*(-1.0./4.0);
t15902 = (t14299.*(t2148+t2513+t2649+t2661+t3582+t11950+t17.*(t258+t2289+t5392+t7559)))./4.0;
t15904 = (t14299.*t14541)./4.0;
t15905 = (t14297.*t14542)./4.0;
t15931 = (t14297.*t14752)./4.0;
t15935 = -t15932;
t15938 = t14299.*(t13026+t17.*(t8963+t7.*(t5026+t5.*(t2959-t2967)))).*(-1.0./4.0);
t15940 = (t14299.*(t13026+t17.*(t8963+t7.*(t5026+t5.*(t2959-t2967)))))./4.0;
t15942 = t14297.*(-t2550+t2696+t2698+t11659+t8.*t11672+t147.*(t71-t391)).*(-1.0./4.0);
t15943 = (t14299.*t14770)./4.0;
t15944 = (t14297.*(-t2550+t2696+t2698+t11659+t8.*t11672+t147.*(t71-t391)))./4.0;
t15956 = (t14297.*t14823)./4.0;
t15959 = (t14299.*t14821)./4.0;
t15960 = -t15958;
t15987 = -t15986;
t15993 = -t15992;
t15996 = t13362.*(t1987-t2621+t3452+t11654+t9.*(t71-t391).*6.1597e-2+t17.*(t426-t581)+t9.*(t9166-t11658)).*(-1.0./4.0);
t15997 = (t13362.*(t1987-t2621+t3452+t11654+t9.*(t71-t391).*6.1597e-2+t17.*(t426-t581)+t9.*(t9166-t11658)))./4.0;
t16000 = t13377.*(t1987-t2621+t3452+t11654+t9.*(t71-t391).*6.1597e-2+t17.*(t426-t581)+t9.*(t9166-t11658)).*(-1.0./4.0);
t16031 = t14299.*(t2497+t2680+t3516+t9.*(t210+t2107+t7423+t9121)+t17.*(t9166-t11658)).*(-1.0./4.0);
t16032 = t14297.*(t3452+t11654+t9.*(t71-t391).*6.1597e-2+t17.*(t426-t581)+t9.*(t9166-t11658)).*(-1.0./4.0);
t16033 = (t14297.*(t3452+t11654+t9.*(t71-t391).*6.1597e-2+t17.*(t426-t581)+t9.*(t9166-t11658)))./4.0;
t16047 = t14297.*(t2091+t2497+t2579+t2680+t3516+t9.*(t210+t2107+t7423+t9121)+t17.*(t9166-t11658)).*(-1.0./4.0);
t16048 = t14297.*(t1987-t2621+t3452+t11654+t9.*(t71-t391).*6.1597e-2+t17.*(t426-t581)+t9.*(t9166-t11658)).*(-1.0./4.0);
t16049 = t14299.*(t2091+t2497+t2579+t2680+t3516+t9.*(t210+t2107+t7423+t9121)+t17.*(t9166-t11658)).*(-1.0./4.0);
t16050 = t14299.*(t1987-t2621+t3452+t11654+t9.*(t71-t391).*6.1597e-2+t17.*(t426-t581)+t9.*(t9166-t11658)).*(-1.0./4.0);
t16051 = (t14299.*(t2091+t2497+t2579+t2680+t3516+t9.*(t210+t2107+t7423+t9121)+t17.*(t9166-t11658)))./4.0;
t16072 = t16070.*xd;
t16165 = q1d.*t16164;
t16171 = q1d.*t16170;
t16174 = q1d.*t16172;
t16183 = t10579+t10590+t10618+t10636+t12762+t12777+t14361+t14363+t14369+t14372+t14449+t14455+t14495+t14500;
t16184 = t10579+t10590+t10618+t10636+t12767+t12780+t14362+t14366+t14373+t14376+t14446+t14450+t14493+t14497;
t16191 = t8845+t8862+t11361+t11363+t13105+t13266+t14536+t14540+t14599+t14609+t14686+t14688+t14797+t14810;
t16192 = t8863+t8883+t11354+t11371+t13105+t13266+t14536+t14540+t14599+t14609+t14686+t14688+t14797+t14810;
t16200 = t9771+t9778+t11407+t11422+t13166+t13322+t14645+t14649+t14779+t14789+t14818+t14819+t15032+t15033;
t16201 = t9771+t9778+t11407+t11422+t13168+t13325+t14648+t14651+t14777+t14784+t14822+t14824+t15030+t15031;
t16208 = t8918+t8923+t10661+t10664+t13304+t13486+t14937+t14939+t15070+t15073+t15077+t15083+t15274+t15280;
t16209 = t8918+t8923+t10661+t10664+t13306+t13492+t14934+t14938+t15069+t15075+t15079+t15082+t15277+t15282;
t16219 = t10639+t10655+t12521+t12527+t13534+t13699+t15167+t15170+t15272+t15276+t15328+t15329+t15464+t15468;
t16220 = -xd.*(t10657+t10678+t12523+t12525-t13534-t13699+t15165+t15166+t15271+t15273+(t10149.*(t10403+t9.*(t10158+t16.*(t4542-t6448)).*7.35522e-1))./4.0+(t14185.*(t3418-t3879+t4324-t5228+t5802+t9.*(t71-t391).*4.5305948634e-2+t17.*(t426-t581).*7.35522e-1))./4.0+(t14280.*(t1987-t2621+t3452-t4730+t5359+t9.*(t71-t391).*6.1597e-2+t17.*(t426-t581)))./4.0+(t11470.*(t10174+t9.*(t10158+t16.*(t4542-t6448))))./4.0);
t16221 = t10657+t10678+t12523+t12525+t13534+t13699+t15167+t15170+t15272+t15276+t15328+t15329+t15464+t15468;
t16229 = q1d.*t16228;
t16248 = q1d.*t16247;
t16251 = q1d.*t16250;
t16253 = q1d.*t16252;
t16272 = t8786+t8793+t8857+t8867+t11055+t11066+t11847+t11974+t12691+t12699+t12799+t12807+t12847+t12854+t12881+t12969+t12975+t12997+t13009+t13057+t13073+t13078+t13096+t13100+t13185+t13468+t13474+t13645+t14505+t14513+t14620+t14621;
t16273 = -xd.*(-t8786-t8793+t8848+t11052+t11062-t11847-t11974+t12684+t12708+t12795+t12810+t12855+t12863+t12875-t12969-t12975+t13003+t13004+t13061+t13075+t13076-t13096-t13100+t13188+t13469+t13473+t13648+t14509+t14510+t14618+t14625+t7.*t8.*(t4542-t6448).*1.17633784675e-2);
t16274 = t8786+t8793+t8857+t8867+t11052+t11062+t11847+t11974+t12684+t12708+t12795+t12810+t12855+t12863+t12875+t12969+t12975+t13003+t13004+t13061+t13075+t13076+t13096+t13100+t13188+t13469+t13473+t13648+t14509+t14510+t14618+t14625;
t16287 = t7373+t7381+t9783+t9819+t11549+t11889+t11904+t11995+t12921+t12933+t13020+t13043+t13051+t13087+t13088+t13128+t13247+t13252+t13310+t13330+t13336+t13398+t13400+t13516+t13517+t13701+t13957+t13961+t14653+t14659+t14828+t14833;
t16288 = t7351+t7368+t9796+t9808+t11549+t11891+t11904+t11999+t12921+t12933+t13020+t13043+t13051+t13087+t13088+t13128+t13247+t13252+t13310+t13330+t13336+t13395+t13403+t13510+t13524+t13701+t13957+t13961+t14653+t14659+t14828+t14833;
t16289 = xd.*(-t7373-t7381+t9796+t9808+t11549+t11891+t11904+t11999+t12921+t12933+t13020+t13043+t13051+t13087+t13088+t13128+t13247+t13252+t13310+t13330+t13336+t13395+t13403+t13510+t13524+t13701+t13957+t13961+t14653+t14659+t14828+t14833);
t16293 = t10639+t10655+t12521+t12527+t13534+t13699+t16028+t16030+t16035+t16036+t16041+t16045+t16059+t16063;
t16295 = -xd.*(t10657+t10678+t12523+t12525-t13534-t13699-t16028+t16029+t16034-t16035+t16042+t16061+(t14185.*(t3418-t3879+t4324+t11855+t9.*(t71-t391).*4.5305948634e-2+t17.*(t426-t581).*7.35522e-1+t9.*(t9166-t11658).*7.35522e-1))./4.0+(t14280.*(t1987-t2621+t3452+t11654+t9.*(t71-t391).*6.1597e-2+t17.*(t426-t581)+t9.*(t9166-t11658)))./4.0);
t16296 = t10657+t10678+t12523+t12525+t13534+t13699+t16028+t16030+t16035+t16036+t16041+t16045+t16059+t16063;
t16297 = q1d.*t16294;
t16302 = t7304+t7318+t8897+t8905+t11098+t11281+t11688+t12005+t12529+t12537+t12620+t12622+t13224+t13225+t13329+t13422+t13427+t13521+t13536+t13559+t13796+t13897+t13903+t13910+t13911+t14170+t14250+t14251+t14859+t14867+t14996+t15006;
t16303 = t7304+t7318+t8897+t8905+t11098+t11281+t11693+t12012+t12529+t12537+t12620+t12622+t13229+t13230+t13332+t13426+t13428+t13514+t13527+t13562+t13788+t13893+t13899+t13907+t13913+t14167+t14249+t14252+t14861+t14863+t14999+t15005;
t16315 = phid.*t16314;
t16318 = q1d.*t16317;
t16346 = t7041+t7054+t7658+t7686+t8006+t8672+t9347+t9374+t9375+t9382+t9412+t9427+t9787+t9799+t10028+t10029+t10031+t10036+t10041+t10389+t10533+t10980+t11181+t11186+t11355+t11367+t11705+t11942+t11944+t12107+t12129+t12135+t12138+t12160+t12365+t12408+t12416+t12471+t12827+t12870+t13041+t13049+t13200+t13208+t13283+t13653+t13873+t13880+t13954+t13955+t14138+t14144+t14177+t14178+t14739+t14741+t14998+t15004;
t16348 = t7036+t7056+t7658+t7686+t8022+t8678+t9347+t9374+t9375+t9382+t9412+t9427+t9775+t9813+t10022+t10028+t10036+t10041+t10043+t10371+t10528+t10980+t11181+t11186+t11355+t11367+t11705+t11946+t11949+t12107+t12129+t12135+t12144+t12165+t12370+t12408+t12416+t12471+t12830+t12870+t13041+t13049+t13200+t13208+t13283+t13653+t13873+t13880+t13950+t13951+t14135+t14141+t14177+t14178+t14739+t14741+t14998+t15004;
t16355 = -phid.*(-t4238+t4295-t4456+t4713+t4744+t4783+t4797+t4947+t5325+t5330+t5336+t5390+t5749+t5814+t6360+t6396+t7007+t7031+t7103+t7491+t7572+t7583+t8090+t8624+t8648+t8676+t8721+t11997+t13108-t13433+t13688-t13853+t14033+t14034+t14196+t14197+t14200+t14205+t14255+t14351+t14460+t14461+t14479+t14483+t14554+t14591+t14592+t14871-t14895-t15140+t15619+t15620+t15689+t15690+(t9.*(t578.*4.28e-4+t2566-t2597+t905.*(t71-t391)+t1021.*(t71-t391)))./4.0+t8.*(t210+t2107+t7423+t9121).*1.17633784675e-2+t17.*(-t2550+t2696+t2698+t11659+t8.*t11672+t147.*(t71-t391)).*1.13264871585e-2+t17.*(-t3823+t3970+t11861+t8.*t11864+t972.*(t71-t391)+t2777.*(t71-t391)).*1.539925e-2+t8.*(t71-t391).*5.187945860934245e-5+t16.*(t71-t391).*4.67845486573025e-5+(t2522.*(t689-t740))./4.0+(t16.*t3286.*(t71-t391))./4.0);
t16356 = t4238+t4295+t4310+t4456+t4713+t4725+t4740+t4744+t4783+t4797+t4956+t4962+t5325+t5330+t5336+t5390+t5749+t5814+t6360+t6396+t7007+t7031+t7103+t7501+t7572+t7576+t7583+t8090+t8624+t8648+t8676+t8721+t12002+t12007+t13108+t13433+t13688+t13853+t14033+t14034+t14196+t14197+t14200+t14205+t14255+t14351+t14460+t14461+t14479+t14483+t14554+t14591+t14592+t14871+t14895+t14896+t15140+t15141+t15619+t15620+t15689+t15690;
t16360 = t5263+t5265+t5284+t5289+t7700+t7740+t8427+t8660+t8906+t8925+t9111+t9118+t9237+t9249+t9344+t9371+t9513+t9524+t9552+t9631+t9701+t9827+t9861+t9972+t9984+t9986+t10227+t10472+t10882+t10890+t11065+t11201+t11217+t11419+t11425+t11521+t11551+t11740+t11755+t11760+t11819+t11917+t12413+t12426+t12617+t12626+t12952+t13113+t13115+t13152+t13158+t13226+t13233+t13523+t13535+t13543+t13558+t13565+t13567+t13995+t14218+t14219+t14478+t14480+t14941+t14944+t15171+t15177;
t16362 = t5263+t5265+t5284+t5289+t7720+t7753+t8427+t8660+t8906+t8925+t9111+t9118+t9223+t9239+t9355+t9359+t9507+t9518+t9552+t9641+t9701+t9839+t9851+t9978+t9980+t9981+t10222+t10467+t10878+t10886+t11061+t11201+t11217+t11417+t11426+t11521+t11551+t11744+t11746+t11749+t11819+t11910+t12413+t12422+t12619+t12623+t12958+t13107+t13117+t13152+t13158+t13232+t13235+t13523+t13541+t13543+t13561+t13569+t13572+t13998+t14217+t14220+t14473+t14482+t14943+t14945+t15173+t15179;
t16373 = phid.*t16372;
t16375 = phid.*t16374;
t16377 = phid.*t16376;
t16381 = phid.*t16380;
t16382 = t5536+t5542+t5619+t6200+t6510+t6570+t7339+t7363+t7803+t7804+t7891+t7897+t7957+t7958+t8295+t8304+t8381+t8421+t8977+t8987+t9092+t9339+t9388+t9674+t9678+t9826+t9865+t10056+t10076+t10237+t10273+t10319+t10981+t10986+t11015+t11071+t11440+t11553+t11563+t11669+t11673+t11711+t11741+t11906+t11913+t11989+t12082+t12234+t12245+t12320+t12463+t12632+t12641+t12745+t12977+t13131+t13133+t13480+t13493+t13499+t13528+t13587+t13744+t13889+t13898+t13986+t13989+t14143+t14426+t14427+t14716+t14720+t15084+t15085+t15283+t15284;
t16383 = xd.*(t5536+t5542+t5619+t6200-t6503+t6570+t7339+t7363+t7803+t7804+t7891+t7897+t7957+t7958+t8295+t8304+t8381+t8421+t8977+t8987+t9092+t9339+t9388+t9674+t9678+t9826+t9865+t10056+t10076+t10237+t10273+t10319+t10981+t10986+t11015+t11071+t11440+t11553+t11563+t11669+t11673+t11711+t11741+t11906+t11913+t11989+t12082+t12234+t12245+t12320+t12463+t12632+t12641+t12745+t12977+t13131+t13133+t13480+t13493+t13499+t13528+t13587+t13744+t13889+t13898+t13986+t13989+t14143+t14426+t14427+t14716+t14720+t15084+t15085+t15283+t15284);
t16384 = t5555+t5560+t5600+t6200+t6503+t6570+t7316+t7379+t7790+t7818+t7891+t7897+t7957+t7958+t8295+t8304+t8388+t8426+t8977+t8987+t9092+t9339+t9388+t9670+t9684+t9826+t9865+t10048+t10090+t10237+t10263+t10319+t10981+t10986+t11009+t11071+t11440+t11565+t11576+t11669+t11673+t11711+t11741+t11908+t11922+t11994+t12082+t12234+t12245+t12320+t12468+t12632+t12641+t12745+t12977+t13131+t13133+t13487+t13489+t13499+t13528+t13587+t13744+t13889+t13898+t13985+t13990+t14143+t14426+t14427+t14716+t14720+t15084+t15085+t15283+t15284;
t16385 = t6599+t6875+t6901+t7556+t8004+t8135+t8212+t8251+t9009+t9011+t9036+t9387+t9414+t10720+t11373+t11386+t11437+t13484+t13597+t13795+t14049+t14790+t14793+t14795+t14799+t14885+t14887+t14897+t14898+t14901+t14902+t14952+t14953+t15101+t15112+t15256+t15257+t15434+t15440+t15453+t15457+t15808+t15811+t15819+t15821;
t16387 = phid.*t16386;
t16396 = phid.*t16395;
t16399 = q1d.*t16398;
t16427 = phid.*t16426;
t16430 = phid.*t16429;
t16431 = t5871+t5932+t6011+t6547+t6771+t6825+t7106+t7173+t7872+t7979+t7989+t8032+t8034+t8234+t8523+t8627+t8915+t9073+t9097+t9368+t9378+t9580+t10145+t11829+t11837+t12218+t12604+t13207+t13213+t13317+t13320+t13459+t13479+t13605+t13606+t13619+t13620+t13817+t13818+t13839+t13840+t14019+t14020+t14023+t14025+t14104+t14105+t14106+t14107+t14640+t14694+t14812+t14815+t14905+t14909+t15023+t15025+t15068+t15076+t15370+t15398+t15649+t15651+t15667+t15668+t15837+t15838+t15844+t15846;
t16433 = phid.*t16432;
t16444 = t4816+t5349+t5391+t5498+t5591+t5594+t5774+t5905+t5938+t6073+t6890+t6976+t7032+t7088+t7121+t7347+t7367+t7661+t7663+t7726+t7746+t8094+t8114+t8623+t8834+t8972+t8994+t9060+t9094+t9875+t9983+t10148+t10709+t11268+t11277+t11383+t11401+t11459+t11461+t11466+t11474+t11574+t11584+t11657+t11662+t11898+t11947+t12021+t12083+t12317+t12454+t12597+t12614+t12828+t12850+t13223+t13423+t13564+t13570+t13633+t13641+t13719+t13723+t13845+t13849+t13859+t14083+t14132+t14190+t14296+t14300+t14347+t14349+t14847+t14849+t14857+t14878+t14880+t14891+t15163+t15164+t15287+t15318+t15326+t15369+t15603+t15604+t15605+t15606+t15847+t15848+t15851+t15852;
t16458 = t3629+t3663+t3770+t4422+t4525+t4674+t4812+t4968+t5288+t5889+t5896+t5913+t5916+t5918+t5946+t6125+t6126+t6260+t6362+t6406+t6948+t7038+t7050+t7350+t7627+t7673+t7788+t7971+t8014+t8105+t8448+t8469+t8492+t8706+t8722+t8777+t8891+t8934+t8969+t9042+t9080+t9126+t9139+t9379+t9380+t9384+t9410+t9496+t9583+t9602+t9659+t9669+t9940+t9959+t9971+t10143+t10214+t10224+t10411+t10425+t10537+t11117+t11121+t11502+t11504+t11972+t11984+t12029+t12037+t12167+t12181+t12359+t12566+t12695+t12735+t13199+t13218+t13307+t13314+t13664+t13694+t13731+t13741+t13813+t13842+t13885+t13886+t13924+t13943+t13987+t14171+t14172+t14174+t14417+t14420+t14422+t14425+t14929+t14933+t14960+t14961+t14968+t14969+t15298+t15309+t15381+t15389+t15456+t15459+t15675+t15677+t15679+t15680+t15853+t15854+t15857+t15858;
t16460 = phid.*t16459;
t16473 = t559+t568+t2420+t2424+t4026+t4032+t4549+t4563+t4638+t4673+t5322+t5323+t5341+t5378+t5531+t5895+t5897+t5911+t6074+t6111+t6542+t6974+t6987+t7068+t7073+t7092+t7094+t7152+t7261+t7860+t7951+t8046+t8081+t8082+t8092+t8120+t8146+t8152+t8250+t8264+t8274+t8289+t8457+t8475+t8478+t8482+t8522+t8526+t8548+t8754+t9014+t9026+t9160+t9162+t9205+t9208+t9367+t9426+t9451+t9627+t9912+t9915+t9946+t9951+t10327+t10337+t10404+t10729+t10740+t10768+t10807+t10859+t10864+t11522+t11524+t11530+t11762+t11763+t12080+t12250+t12326+t12337+t12536+t12602+t12646+t12664+t12755+t13124+t13125+t13142+t13143+t13187+t13635+t13639+t14015+t14016+t14021+t14024+t14046+t14061+t14222+t14266+t14270+t14271+t14273+t14276+t14277+t14281+t14286+t14529+t14835+t14839+t15039+t15047+t15049+t15050+t15444+t15447+t15481+t15482+t15574+t15576+t15595+t15596+t15598+t15599+t15876+t15877+t15880+t15881;
t13509 = -t13503;
t13676 = -t13672;
t13931 = -t13926;
t13947 = -t13944;
t14115 = -t14114;
t14401 = -t14398;
t14404 = -t14400;
t14415 = -t14412;
t14421 = -t14418;
t14467 = -t14464;
t14469 = -t14465;
t14471 = -t14466;
t14474 = -t14468;
t14475 = -t14470;
t14477 = -t14472;
t14532 = -t14528;
t14538 = -t14533;
t14546 = -t14545;
t14556 = -t14550;
t14600 = -t14595;
t14632 = -t14630;
t14634 = -t14631;
t14663 = -t14658;
t14667 = -t14666;
t14685 = -t14680;
t14707 = -t14704;
t14708 = -t14705;
t14747 = -t14745;
t14817 = -t14811;
t14820 = -t14816;
t14827 = -t14825;
t14829 = -t14826;
t14875 = -t14874;
t14935 = -t14931;
t14948 = -t14946;
t14954 = -t14951;
t14957 = -t14956;
t14959 = -t14958;
t15059 = -t15057;
t15065 = -t15062;
t15097 = -t15093;
t15100 = -t15094;
t15104 = -t15096;
t15107 = -t15099;
t15160 = -t15159;
t15175 = -t15172;
t15184 = -t15182;
t15359 = -t15352;
t15372 = -t15368;
t15872 = -t15871;
t15874 = -t15873;
t15906 = -t15905;
t15934 = -t15931;
t15945 = -t15943;
t15961 = -t15959;
t16185 = t16184.*xd;
t16193 = t16192.*xd;
t16196 = -yd.*(t8886+t8907+t11429+t11431-t13130-t13291+t14545+t14550-t14627-t14633+t14697+t14700-t14831-t14837);
t16202 = t16201.*xd;
t16210 = t16209.*xd;
t16227 = -yd.*(t10600+t10609+t12501+t12510-t13551-t13712+t15181+t15182+t15289+t15293-t15358-t15476+(t14209.*(t3418-t3879+t4324-t5228+t5802+t9.*(t71-t391).*4.5305948634e-2+t17.*(t426-t581).*7.35522e-1))./4.0+(t14297.*(t1987-t2621+t3452-t4730+t5359+t9.*(t71-t391).*6.1597e-2+t17.*(t426-t581)))./4.0);
t16230 = t10602+t10617+t10877+t11038+t11048+t11243+t12656+t12663+t12765+t12776+t12778+t12789+t12908+t12912+t13379+t13384+t13478+t13481+t14454+t14456+t14499+t14502;
t16232 = t10602+t10617+t10877+t11044+t11050+t11243+t12653+t12666+t12770+t12773+t12782+t12784+t12907+t12913+t13379+t13384+t13478+t13481+t14452+t14458+t14496+t14503;
t16299 = t10600+t10609+t12501+t12510+t13551+t13712+t16031+t16033+t16038+t16039+t16048+t16051+t16066+t16069;
t16300 = t10610+t10619+t12505+t12507+t13551+t13712+t16031+t16033+t16038+t16039+t16048+t16051+t16066+t16069;
t16301 = -yd.*(t10600+t10609+t12501+t12510-t13551-t13712+t16032+t16037+t16049+t16067+(t14299.*(t2497+t2680+t3516+t9.*(t210+t2107+t7423+t9121)+t17.*(t9166-t11658)))./4.0+(t14209.*(t3418-t3879+t4324+t11855+t9.*(t71-t391).*4.5305948634e-2+t17.*(t426-t581).*7.35522e-1+t9.*(t9166-t11658).*7.35522e-1))./4.0+(t14213.*(t3845+t3925+t4339+t9.*(t210+t2107+t7423+t9121).*7.35522e-1+t17.*(t9166-t11658).*7.35522e-1))./4.0+(t14297.*(t1987-t2621+t3452+t11654+t9.*(t71-t391).*6.1597e-2+t17.*(t426-t581)+t9.*(t9166-t11658)))./4.0);
t16304 = t16303.*xd;
t16305 = t7383+t7395+t8957+t8962+t11170+t11346+t11716+t12025+t12567+t12569+t12682+t12690+t13249+t13250+t13354+t13438+t13447+t13548+t13553+t13576+t13823+t13920+t13925+t13932+t13937+t14184+t14257+t14258+t14874+t14877+t15008+t15018;
t16310 = -xd.*(t8808+t8820+t9138+t9343-t10997-t10998+t11097+t11101+t11270+t11284+t11360+t11384-t11511-t11517+t11528+t11542-t11550+t11840+t11853-t12393-t12803-t12903-t13160+t13238+t13251+t13324+t13334-t13538+t13926+t13928+t14116+t14121+t14584+t14754+(t5441.*(t10158+t16.*(t4542-t6448)))./4.0+(t5213.*(t10403+t9.*(t10158+t16.*(t4542-t6448)).*7.35522e-1))./4.0+(t3266.*(t5110-t6808))./4.0+(t4879.*(t4542-t6448))./4.0+(t3780.*(t10384+t16.*(t4542-t6448).*1.666555))./4.0+(t7538.*(t10174+t9.*(t10158+t16.*(t4542-t6448))))./4.0);
t16313 = -yd.*(t8846+t8856+t9151-t9348+t9369-t9396+t11122+t11125+t11303+t11314+t11427+t11445+t11598+t11610+t11880+t11894-t12825-t12840-t12922-t12932-t13174+t13287+t13295+t13366+t13378-t13555+t13962+t13965+t14139+t14145+t14595-t14596+t14780-t14787+t8.*t4024.*(t6452-t8229).*4.1663875e-1+t16.*t4021.*(t6452-t8229).*4.1663875e-1+t16.*t5696.*(t6452-t8229).*1.838805e-1+(t8.*t6046.*(t6452-t8229))./4.0+(t16.*t6069.*(t6452-t8229))./4.0+(t16.*t8477.*(t6452-t8229))./4.0);
t16319 = t8850+t8864+t10622+t10637+t11928+t12142+t12808+t12904+t13461+t13472+t13649+t13660+t13669+t13797+t13799+t13856+t14045+t14051+t14065+t14233+t14240+t14301+t14305+t14353+t14354+t14371+t14563+t14564+t15034+t15048+t15185+t15192;
t16320 = t8850+t8864+t10622+t10637+t11930+t12151+t12808+t12904+t13457+t13467+t13647+t13656+t13665+t13802+t13803+t13854+t14047+t14055+t14070+t14235+t14238+t14301+t14305+t14353+t14354+t14375+t14560+t14566+t15036+t15043+t15188+t15191;
t16321 = -xd.*(-t8850-t8864-t10622+t10627+t11928+t12142-t12808-t12904+t13461+t13472+t13649+t13660+t13669+t13797+t13799+t13856+t14045+t14051+t14065+t14233+t14240-t14301-t14305-t14353-t14354+t14371+t14563+t14564+t15034+t15048+t15185+t15192);
t16332 = t7281+t7284+t7361+t7369+t9376+t9430+t10274+t10296+t11017+t11024+t11139+t11152+t11230+t11234+t11300+t11369+t11374+t11412+t11428+t11548+t11554+t11581+t11591+t11649+t11756+t11835+t11869+t11883+t11901+t11902+t12293+t12453+t12923+t12925+t13046+t13047+t13263+t13644+t13682+t13686+t13768+t13789+t14108+t14114+t14368+t14383+t14689+t14690+t14884+t14888;
t16339 = -xd.*(-t5605-t5612+t7342+t7377+t9411+t9440+t10010+t10405+t10660+t10693+t10828+t10837+t11089+t11096-t11471+t11485+t11690+t11728-t11733-t11939+t11954+t12055-t12061-t12070+t12238-t12244+t12259-t12412-t12612-t12613+t12713+t12851+t12868+t12950+t12967-t13153-t13222-t13424-t13598-t14014+t14410+t14412+t14699+t14703+t14910+t15116+(t7646.*(t10158+t16.*(t4542-t6448)))./4.0+(t7799.*(t10403+t9.*(t10158+t16.*(t4542-t6448)).*7.35522e-1))./4.0+(t6014.*(t10384+t16.*(t4542-t6448).*1.666555))./4.0+(t9537.*(t10174+t9.*(t10158+t16.*(t4542-t6448))))./4.0);
t16344 = -yd.*(t5642+t5652+t7414+t7417+t9495+t9508+t10037+t10422+t10746+t10750+t10869+t10870+t11140+t11154-t11488+t11503+t11719+t11754-t11960+t11981+t12064+t12263+t12280+t12728+t12910+t12911+t13017+t13022-t13245-t13272-t13439-t13452-t13602-t14026+t14428+t14430+t14717+t14721+t14931-t14936+t15125-t15129+(t5634.*(t6806-t8574))./4.0+(t8050.*(t6452-t8229))./4.0+t16.*t7079.*(t6452-t8229).*4.1663875e-1+t8.*t7116.*(t6452-t8229).*4.1663875e-1+t16.*t8191.*(t6452-t8229).*1.838805e-1+(t8.*t9112.*(t6452-t8229))./4.0+(t16.*t9110.*(t6452-t8229))./4.0+(t16.*t10141.*(t6452-t8229))./4.0);
t16350 = -yd.*(t6999+t7020-t7671+t7995+t8667+t9389-t9402-t9415-t9444-t9473-t9484+t9776+t9814+t10023+t10040+t10044+t10049-t10060+t10372+t10529+t10992+t11198+t11379+t11729+t11936+t11940+t12114+t12131+t12154-t12180+t12363-t12436+t12822-t13053-t13066-t13220-t13227-t13301-t13678+t13900+t13944+t13946+t14128+t14134+t14194+t14745-t14749+t15007-t15014+(t6430.*(t1748-t1821))./4.0+(t4064.*(t6806-t8574))./4.0+(t5646.*(t6452-t8229))./4.0+(t5234.*(t8589-t8592))./4.0+(t6884.*(t8219-t8226))./4.0+(t6302.*(t8582-t8586))./4.0+(t8640.*(t8219-t8226))./4.0+(t6761.*(t8583-t11188))./4.0+(t9185.*(t8221-t11008))./4.0);
t16361 = t16360.*xd;
t16363 = t5281+t5286+t5299+t5308+t7666+t7719+t8453+t8683+t8964+t8986+t9155+t9159+t9267+t9274+t9418+t9421+t9542+t9551+t9573+t9651+t9763+t9886+t9889+t9988+t10000+t10002+t10262+t10479+t10891+t10902+t11093+t11262+t11288+t11443+t11446+t11602+t11622+t11771+t11776+t11790+t11859+t11931+t12439+t12450+t12639+t12649+t12982+t13139+t13141+t13186+t13191+t13253+t13260+t13552+t13575+t13582+t13583+t13595+t13596+t14002+t14232+t14234+t14487+t14489+t14956+t14958+t15189+t15193;
t16365 = -yd.*(t5297+t7666+t7719-t9159+t9267+t9274+t9418+t9421+t9542+t9551-t9573+t9651+t9886+t9889+t9988+t10000+t10002+t10262+t10479+t10891+t10902+t11093+t11279+t11443+t11446+t11620+t11771+t11776+t11790+t11851+t11931+t12439+t12445+t12639+t12649+t12982+t13139+t13141+t13190+t13253+t13260+t13552+t13575+t13583+t13592+t13596+t14002+t14232+t14234+t14487+t14489+t14956+t14958+t15189+t15193+(t7796.*(t9.*(t16.*(t30.*(t2425-t2468)+t68.*(t2425-t2468))+t8.*(t7.*(t4650+t34.*(t2425-t2468))+t47.*(t2425-t2468)))+t17.*(t4654+t15.*(t4650+t34.*(t2425-t2468)))))./4.0+(t5331.*(t30.*(t2425-t2468)+t68.*(t2425-t2468)))./4.0+(t6046.*(t16.*(t30.*(t2425-t2468)+t68.*(t2425-t2468))+t8.*(t7.*(t4650+t34.*(t2425-t2468))+t47.*(t2425-t2468))))./4.0+(t4024.*(t16.*(t30.*(t2425-t2468)+t68.*(t2425-t2468)).*1.666555+t8.*(t7.*(t4650+t34.*(t2425-t2468))+t47.*(t2425-t2468)).*1.666555))./4.0+t7.*(t7.*(t4650+t34.*(t2425-t2468)).*1.225946+t47.*(t2425-t2468).*1.225946).*8.639075e-2+t30.*(t2425-t2468).*9.5384188575e-2+t34.*(t2425-t2468).*1.8732399795e-1+t68.*(t2425-t2468).*9.5384188575e-2+(t3424.*(t30.*(t2425-t2468).*1.225946+t68.*(t2425-t2468).*1.225946))./4.0+t15.*(t4654+t15.*(t4650+t34.*(t2425-t2468))).*1.059103943995e-1+(t5443.*(t4654+t15.*(t4650+t34.*(t2425-t2468))))./4.0+t7.*(t7.*(t4650+t34.*(t2425-t2468))+t47.*(t2425-t2468)).*1.059103943995e-1+(t5329.*(t9.*(t16.*(t30.*(t2425-t2468)+t68.*(t2425-t2468))+t8.*(t7.*(t4650+t34.*(t2425-t2468))+t47.*(t2425-t2468))).*7.35522e-1+t17.*(t4654+t15.*(t4650+t34.*(t2425-t2468))).*7.35522e-1))./4.0);
t16369 = t7309+t7314+t8781+t8789+t10195+t10551+t11032+t11043+t11843+t11858+t12052+t12168+t12176+t12200+t12214+t12433+t12438+t12446+t12496+t12502+t12509+t12592+t12598+t12703+t12704+t12766+t12779+t12852+t12970+t12972+t13077+t13511+t13526+t13584+t13697+t13704+t13966+t14216+t14447+t14453+t14492+t14501+t14736+t14740+t14992+t15000+t15148+t15151+t15315+t15319;
t16370 = -yd.*(t7328+t7338+t8774+t8795+t10202+t10562+t11039+t11047-t12176-t12438+t12441+t12499+t12504+t12595+t12596-t12703+t12771+t12783-t12852-t12972+t13074+t13505-t13584+t13693+t13958+t14215+t14448+t14451+t14494+t14498-t14736-t14992+t15150+t15312+((t6806-t8574).*(t921+t1317-t5853))./4.0+((t6452-t8229).*(t2810+t2988-t7937))./4.0+(t14213.*(t2740+t3849+t3968+t3972-t5255+t17.*(t260+t468+t570+t2298).*7.35522e-1))./4.0+(t13189.*(t3418-t3879+t4324-t5228+t5802+t9.*(t71-t391).*4.5305948634e-2+t17.*(t426-t581).*7.35522e-1))./4.0+(t13391.*(t1987-t2621+t3452-t4730+t5359+t9.*(t71-t391).*6.1597e-2+t17.*(t426-t581)))./4.0+(t12508.*(t1492+t2158+t2696-t4727))./4.0+(t12307.*(t3063+t3528+t3966-t5230))./4.0+(t10577.*(t495+t572+t1838+t2069+t2107))./4.0+(t10164.*(t2437+t2648+t3129+t3384+t3574))./4.0+(t5853.*(t6806-t8574))./4.0+(t6535.*(t6801-t8594))./4.0+(t7937.*(t6452-t8229))./4.0+(t8791.*(t6452-t8229))./4.0+(t14299.*(t824+t2543+t2699+t2707-t4767+t17.*(t260+t468+t570+t2298)))./4.0+t16.*t8227.*(t6452-t8229).*4.1663875e-1+(t16.*t9744.*(t6452-t8229))./4.0);
t16371 = t7328+t7338+t8774+t8795+t10195+t10551+t11039+t11047+t11843+t11858+t12052+t12168+t12176+t12200+t12214+t12433+t12438+t12446+t12499+t12502+t12504+t12595+t12596+t12703+t12704+t12771+t12783+t12852+t12970+t12972+t13077+t13511+t13526+t13584+t13697+t13704+t13966+t14216+t14448+t14451+t14494+t14498+t14736+t14740+t14992+t15000+t15148+t15151+t15315+t15319;
t16390 = -yd.*(t5572+t5576+t5657+t6529+t7405+t7415+t7864+t7865-t7874+t7896+t7917+t7918-t8279+t8307+t8423+t8444+t8946+t8954-t9082-t9403+t9422+t9690+t9693+t9876-t9888+t10114+t10123+t10245+t10304-t10308+t10970+t11046+t11077+t11435+t11624+t11627+t11664-t11670-t11743+t11943+t11956+t12030+t12091-t12258+t12312+t12473-t12633+t12760-t13122-t13540-t13550+t13560+t13571-t13762-t13912-t13921+t14005+t14007-t14158+t14416+t14418+t14711+t14713-t15113-t15114-t15308-t15310+(t5634.*(t6853-t6864))./4.0+(t5648.*(t6806-t8574))./4.0+(t8053.*(t6452-t8229))./4.0+(t7079.*(t6847-t9563))./4.0+(t8191.*(t6834-t9565))./4.0+(t9110.*(t6472-t9256))./4.0+(t10141.*(t6472-t9256))./4.0+t12.*t3243.*(t2425-t2468).*8.07151e-1+(t12.*t4860.*(t2425-t2468))./4.0);
t16401 = t8850+t8864+t10622+t10637+t11928+t12142+t12808+t12904+t14301+t14305+t14353+t14354+t15516+t15519+t15537+t15539+t15543+t15568+t15569+t15587+t15625+t15626+t15634+t15736+t15867+t15870+t15882+t15885+t15909+t15910+t15967+t15969;
t16402 = t8850+t8864+t10622+t10637+t11930+t12151+t12808+t12904+t14301+t14305+t14353+t14354+t15517+t15518+t15538+t15540+t15541+t15566+t15572+t15588+t15623+t15628+t15636+t15737+t15868+t15869+t15883+t15884+t15907+t15908+t15966+t15968;
t16403 = -xd.*(-t8850-t8864-t10622+t10627+t11928+t12142-t12808-t12904-t14301-t14305-t14353-t14354+t15516+t15519+t15537+t15539+t15543+t15568+t15569+t15587+t15625+t15626+t15634+t15736+t15867+t15870+t15882+t15885+t15909+t15910+t15967+t15969);
t16414 = -yd.*(t5538+t5554+t5559+t5562-t6622+t7372+t7789+t7820+t7954+t8207+t8336+t8356+t8364+t8391+t8402+t8473-t8490-t8514+t8776+t8806+t9051+t9058+t9281+t9390+t9445+t9465-t9494-t9503-t9504-t9911-t9921+t10336+t10508+t11155+t11226+t11229+t11537+t11557-t11571+t11777-t11838+t11920-t12287-t12289+t12310-t12334+t12577+t13086+t13093+t13246+t13261+t13309-t13388-t13612+t13626+t13696-t13914-t13973-t13999+t14000-t14248-t14732+t14778+t14788-t14984+t15029+t15035-t15169+t15172-t15393+t15395+((t6853-t6864).*(t921+t1317-t5853))./4.0+(t11356.*(-t1476-t1540+t2091+t2165+t2579+t8.*(t260+t468+t570+t2298)))./4.0+(t13178.*(t3418-t3879+t4324-t5228+t5802+t9.*(t71-t391).*4.5305948634e-2+t17.*(t426-t581).*7.35522e-1))./4.0+(t13377.*(t1987-t2621+t3452-t4730+t5359+t9.*(t71-t391).*6.1597e-2+t17.*(t426-t581)))./4.0+(t5860.*(t6806-t8574))./4.0+(t6970.*(t6801-t8594))./4.0+(t8310.*(t6452-t8229))./4.0+(t9525.*(t6452-t8229))./4.0+(t8227.*(t6847-t9563))./4.0+(t9744.*(t6472-t9256))./4.0+(t8794.*(t263-t283-t310+t1265))./4.0+(t10942.*(-t3045-t3218+t3458+t3539+t3878+t8.*(t260+t468+t570+t2298).*1.666555))./4.0+t12.*(t881-t912).*(t2425-t2468).*8.07151e-1-t5.*t12.*t6447.*2.01382560198e-1-t5.*t12.*t7236.*6.23745e-2);
t16424 = -yd.*(t5229+t5533+t6212+t6293+t6300+t6319+t6357+t6437+t6577+t6643+t6647+t7330+t7388+t7791+t7823+t7908+t8313+t8353-t8367-t8392+t8400+t8447-t8452+t8849+t9346+t9356-t9417+t9526+t9623-t9756+t9757+t9836+t9846+t10236+t10350-t10364+t10451+t10535+t10867+t11076-t11235+t11244+t11724+t11736+t11784+t12057-t12155+t12235+t12247-t12544+t12545-t12679+t12721-t12996+t13010+t13024+t13506+t13542+t13603+t13776-t13814-t13836+t13892+t13906-t14052-t14060-t14075+t14163-t14310+t14312-t14365+t14604+t15072+t15080+t15275+t15281+t15368-t15371-t15479+t15483+((t7.*(t4650+t34.*(t2425-t2468)).*1.225946+t47.*(t2425-t2468).*1.225946).*(t921+t1317-t5853))./4.0+(t6767.*(t30.*(t2425-t2468)+t68.*(t2425-t2468)))./4.0+((t7.*(t4650+t34.*(t2425-t2468))+t47.*(t2425-t2468)).*(t2810+t2988-t7937))./4.0+(t6988.*(t6806-t8574))./4.0+(t7875.*(t6801-t8594))./4.0+(t9216.*(t6452-t8229))./4.0+(t9992.*(t6452-t8229))./4.0+(t4611.*(t30.*(t2425-t2468).*3.587895+t68.*(t2425-t2468).*3.587895))./4.0+(t9967.*(t4654+t15.*(t4650+t34.*(t2425-t2468))))./4.0+(t11470.*(t8329+t17.*(t16.*(t30.*(t2425-t2468)+t68.*(t2425-t2468))+t8.*(t7.*(t4650+t34.*(t2425-t2468))+t47.*(t2425-t2468)))))./4.0+t4.*t3318.*(t2425-t2468).*8.07151e-1+t12.*t3316.*(t2425-t2468).*8.07151e-1+(t4.*t4908.*(t2425-t2468))./4.0+(t12.*t4906.*(t2425-t2468))./4.0);
t16438 = -yd.*(t7328+t7338+t8774+t8795+t10202+t10562+t11039+t11047+t12499+t12504+t12595+t12596+t12771+t12783+t14211+t14214+t14269+t14328+t14335+t14342+t14344+t14437+t14448+t14451+t14490+t14494+t14498+t14614+t14615+t14751+t14988+t14991+t15105+t15110+t15207+t15208+t15224+t15392+t15413+t15415+t15416+t15532+t15942+t15943+t15981+t15986+t16004+t16007+t16023+t16027);
t16439 = t7309+t7314+t8781+t8789+t10202+t10562+t11032+t11043+t12496+t12509+t12592+t12598+t12766+t12779+t14211+t14214+t14269+t14328+t14335+t14342+t14344+t14437+t14447+t14453+t14490+t14492+t14501+t14614+t14615+t14751+t14988+t14991+t15105+t15110+t15207+t15208+t15224+t15392+t15413+t15415+t15416+t15532+t15942+t15943+t15981+t15986+t16004+t16007+t16023+t16027;
t16462 = -yd.*(t5538+t5554+t5559+t5562-t6622+t7789+t8207+t8776+t8806+t9051+t9058+t9390+t9445-t10331+t10339+t10373+t10519-t10526+t10558+t10574+t10650+t10898+t10905+t10908+t11226+t11229-t11392-t11526-t11527+t11537+t11557+t11722-t11732+t11777+t12051+t12072-t12297-t12302+t12310+t12559+t12832+t13086+t13093+t13246+t13261+t13309+t13696-t13936-t14110-t14129+t14231-t14357-t14359+t14548+t14778+t14788+t15029+t15035-t15264+t15265-t15402+t15420-t15441+t15442+t15503-t15513-t15527-t15612-t15956+t15959-t15991+t15992+t15998+t16017+(t8794.*(t263+t1265-t7252-t5.*t12.*1.0442e-1))./4.0+(t13178.*(t3418-t3879+t4324+t11855+t9.*(t71-t391).*4.5305948634e-2+t17.*(t426-t581).*7.35522e-1+t9.*(t9166-t11658).*7.35522e-1))./4.0+(t12385.*(t6853-t6864))./4.0+(t11247.*(t6806-t8574))./4.0+(t12185.*(t6452-t8229))./4.0+(t11720.*(t6801-t8594))./4.0+(t12669.*(t6452-t8229))./4.0+(t14380.*(t6472-t9256))./4.0+(t14057.*(t6847-t9563))./4.0+(t8166.*(t1786+t2973-t7703-t5.*t12.*3.746479959e-1))./4.0+(t13377.*(t1987-t2621+t3452+t11654+t9.*(t71-t391).*6.1597e-2+t17.*(t426-t581)+t9.*(t9166-t11658)))./4.0+t12.*(t881-t912).*(t2425-t2468).*8.07151e-1);
t16470 = t5229+t5533+t6212+t6293+t6357+t6577+t7330+t7388+t7791+t7823+t7908+t8258+t8260+t8313+t8875+t8877+t9346+t9356+t9522+t9540+t9574+t9591+t9603+t9665+t9801+t9829+t9836+t9846+t10156+t10175+t10236+t10704+t10976+t11076+t11640+t11642+t11724+t11736+t11808+t11809+t12057+t12103+t12197+t12220+t12235+t12247+t12251+t12335+t12343+t12721+t12740+t12859+t13506+t13542+t13716+t13729+t13776+t13884+t13887+t13892+t13906+t13963+t14030+t14085+t14095+t14163+t14173+t14180+t14261+t14329+t15072+t15080+t15147+t15157+t15236+t15237+t15275+t15281+t15316+t15322+t15338+t15428+t15430+t15436+t15487+t15533+t15898+t15902+t15917+t15918+t15946+t15955+t15980+t15983;
t16472 = t5229+t5533+t6212+t6277+t6340+t6577+t7330+t7388+t7791+t7823+t7908+t8242+t8243+t8313+t8855+t8859+t9346+t9356+t9528+t9550+t9578+t9593+t9600+t9657+t9815+t9817+t9836+t9846+t10165+t10181+t10236+t10695+t10985+t11076+t11635+t11648+t11724+t11736+t11796+t11818+t12057+t12104+t12205+t12211+t12235+t12247+t12260+t12327+t12348+t12721+t12743+t12865+t13506+t13542+t13718+t13724+t13776+t13882+t13888+t13892+t13906+t13956+t14029+t14088+t14094+t14163+t14169+t14182+t14260+t14327+t15072+t15080+t15146+t15153+t15241+t15242+t15275+t15281+t15313+t15317+t15334+t15429+t15431+t15439+t15486+t15534+t15899+t15900+t15919+t15920+t15950+t15953+t15982+t15985;
t16475 = phid.*t16473;
t16479 = t3860+t3982+t4535+t4632+t5577+t5579+t6236+t6324+t6371+t6593+t7145+t7153+t7436+t7437+t7459+t7492+t7504+t7532+t7602+t7632+t7637+t7966+t8007+t8125+t8130+t8211+t8293+t8337+t8357+t8372+t8393+t8414+t8487+t8811+t8824+t9477+t9707+t9741+t10082+t10083+t10088+t10097+t10099+t10102+t10316+t10344+t10455+t10571+t10575+t10670+t10909+t10913+t11255+t11730+t11801+t11803+t11804+t11813+t11814+t11815+t12134+t12164+t12324+t12330+t12430+t12629+t12657+t12693+t12706+t12715+t13065+t13264+t13790+t13792+t13793+t13800+t13801+t13805+t13806+t13810+t14043+t14056+t14062+t14313+t14325+t14367+t14433+t14587+t14606+t14748+t15252+t15253+t15254+t15255+t15259+t15260+t15330+t15331+t15466+t15467+t15565+t15570+t15622+t15627+t15630+t15734+t15931+t15932+t15940+t15941+t16040+t16044+t16058+t16062;
t16481 = -yd.*(-t3860+t3958-t4535-t4632-t5577-t5579-t6236-t6371-t6593+t7145+t7153+t7436+t7437+t7459+t7492+t7504+t7532+t7602+t7632+t7637+t7966+t8007+t8125+t8130+t8211+t8293+t8337-t8357+t8363-t8393+t8401+t8472+t8811+t8824+t9464+t9699+t9730+t10082+t10083+t10088+t10097+t10099+t10102+t10311+t10334+t10571+t10575+t10670+t10909+t10913+t11730+t11801+t11803+t11804+t11813+t11814+t11815-t12134+t12158+t12324+t12330-t12430+t12629-t12657+t12685+t12706+t12715-t13065+t13264-t13790+t13792+t13793+t13800+t13801+t13804+t13805+t13806-t14043+t14054+t14313+t14325+t14433+t14587+t14606+t14748+t15252+t15253+t15254+t15255+t15259+t15260+t15327-t15331+t15465-t15467+t15565+t15570+t15622+t15627+t15630+t15734+t15931+t15932+t15940+t15941+t16040+t16044+t16058+t16062+(t12279.*(t1589-t2213+t3195-t4346+t4355+t4748.*7.35522e-1+t2772.*(t71-t391)+t2775.*(t71-t391)))./4.0+(t4356.*(t2425-t2468))./4.0+(t6190.*(t5110-t6808))./4.0+(t8711.*(t4542-t6448))./4.0+(t12484.*(t249-t391.*(1.1e+1./1.25e+2)-t1912.*4.252e-3+t3505+t5357+t693.*(t71-t391)+t784.*(t71-t391)))./4.0);
t16482 = t3857+t3964+t4559+t4628+t5620+t5622+t6259+t6308+t6372+t6614+t7131+t7137+t7418+t7443+t7468+t7477+t7503+t7531+t7590+t7681+t7683+t7943+t8039+t8169+t8171+t8262+t8281+t8340+t8370+t8387+t8389+t8420+t8461+t8784+t8879+t9435+t9750+t9760+t10063+t10064+t10098+t10100+t10103+t10104+t10353+t10357+t10476+t10556+t10584+t10648+t10899+t10925+t11282+t11712+t11750+t11751+t11778+t11779+t11780+t11781+t12169+t12183+t12345+t12351+t12451+t12635+t12694+t12714+t12722+t12729+t13085+t13271+t13759+t13760+t13778+t13779+t13781+t13782+t13825+t13832+t14071+t14079+t14091+t14320+t14338+t14387+t14443+t14602+t14617+t14755+t15232+t15233+t15234+t15235+t15244+t15245+t15352+t15366+t15473+t15478+t15577+t15582+t15631+t15638+t15640+t15738+t15923+t15924+t15925+t15926+t16047+t16050+t16065+t16068;
t16186 = t10620+t10630+t10675+t10690+t12781+t12798+t14385+t14391+t14398+t14400+t14467+t14474+t14517+t14523;
t16187 = t10620+t10630+t10675+t10690+t12788+t12802+t14388+t14394+t14401+t14404+t14464+t14468+t14515+t14519;
t16194 = t8886+t8907+t11429+t11431+t13130+t13291+t14546+t14556+t14627+t14633+t14698+t14702+t14831+t14837;
t16195 = t8910+t8920+t11424+t11433+t13130+t13291+t14546+t14556+t14627+t14633+t14698+t14702+t14831+t14837;
t16203 = t9772+t9779+t11385+t11406+t13176+t13345+t14658+t14666+t14820+t14827+t14841+t14842+t15055+t15056;
t16204 = t9772+t9779+t11385+t11406+t13179+t13350+t14663+t14667+t14816+t14825+t14843+t14844+t15053+t15054;
t16211 = t8971+t8980+t10742+t10743+t13312+t13522+t14948+t14954+t15093+t15095+t15099+t15109+t15295+t15304;
t16212 = -yd.*(t8350.*3.867742437e-3+t10735+t13315+t13529+t14946+t14951+t15092+t15097+t15102+t15107+t15300+t15306+t9.*(t16.*(t30.*(t2425-t2468)+t68.*(t2425-t2468))+t8.*(t7.*(t4650+t34.*(t2425-t2468))+t47.*(t2425-t2468))).*1.563719772e-3+t17.*(t4654+t15.*(t4650+t34.*(t2425-t2468))).*1.563719772e-3);
t16213 = t8971+t8980+t10742+t10743+t13315+t13529+t14946+t14951+t15092+t15097+t15102+t15107+t15300+t15306;
t16225 = t10600+t10609+t12501+t12510+t13551+t13712+t15183+t15184+t15291+t15297+t15355+t15358+t15472+t15476;
t16226 = t10610+t10619+t12505+t12507+t13551+t13712+t15183+t15184+t15291+t15297+t15355+t15358+t15472+t15476;
t16231 = t16230.*xd;
t16233 = t10642+t10673+t10896+t11056+t11064+t11276+t12702+t12707+t12786+t12797+t12800+t12809+t12929+t12935+t13404+t13405+t13525+t13533+t14472+t14475+t14521+t14525;
t16234 = -yd.*(t10652+t11059+t11068+t12698+t12710+t12791+t12794+t12804+t12806+t12928+t12936+t13402-t13405+t13520-t13533+t14470+t14477+t14518+t14527+t16.*(t6452-t8229).*5.01208083475e-2+t16.*t3489.*(t6452-t8229).*1.838805e-1+(t16.*t5365.*(t6452-t8229))./4.0);
t16235 = t10642+t10673+t10896+t11059+t11068+t11276+t12698+t12710+t12791+t12794+t12804+t12806+t12928+t12936+t13404+t13405+t13525+t13533+t14470+t14477+t14518+t14527;
t16275 = t8893+t8900+t8911+t8914+t11074+t11085+t11892+t12006+t12723+t12726+t12820+t12829+t12874+t12877+t12896+t13006+t13014+t13021+t13034+t13084+t13099+t13103+t13132+t13135+t13194+t13495+t13502+t13659+t14528+t14538+t14638+t14639;
t16277 = t8893+t8900+t8911+t8914+t11069+t11081+t11892+t12006+t12720+t12731+t12816+t12831+t12879+t12883+t12892+t13006+t13014+t13028+t13030+t13091+t13101+t13102+t13132+t13135+t13195+t13497+t13501+t13663+t14532+t14533+t14636+t14641;
t16290 = t7329+t7343+t9784+t9820+t11592+t11878+t11925+t11987+t12944+t12964+t13045+t13054+t13071+t13110+t13111+t13147+t13279+t13280+t13319+t13356+t13367+t13392+t13393+t13503+t13504+t13713+t13976+t13977+t14671+t14685+t14846+t14850;
t16291 = t7311+t7321+t9797+t9809+t11592+t11884+t11925+t11990+t12944+t12964+t13045+t13054+t13071+t13110+t13111+t13147+t13279+t13280+t13319+t13356+t13367+t13389+t13397+t13498+t13509+t13713+t13976+t13977+t14671+t14685+t14846+t14850;
t16306 = t7383+t7395+t8957+t8962+t11170+t11346+t11723+t12027+t12567+t12569+t12682+t12690+t13257+t13258+t13361+t13443+t13450+t13547+t13549+t13581+t13820+t13917+t13922+t13929+t13938+t14183+t14256+t14259+t14875+t14876+t15011+t15015;
t16307 = -yd.*(t8952-t11170+t11723+t12027-t12690+t13257+t13258+t13361+t13443+t13450+t13547+t13549+t13581+t13820+t13917+t13922+t13929+t13938+t14183+t14256+t14259+t14875+t14876+t15011+t15015+t9.*(t9.*(t16.*(t30.*(t2425-t2468)+t68.*(t2425-t2468))+t8.*(t7.*(t4650+t34.*(t2425-t2468))+t47.*(t2425-t2468)))+t17.*(t4654+t15.*(t4650+t34.*(t2425-t2468)))).*1.13264871585e-2+t8.*(t30.*(t2425-t2468)+t68.*(t2425-t2468)).*5.01208083475e-2+t16.*(t30.*(t2425-t2468)+t68.*(t2425-t2468)).*1.17633784675e-2+t8.*(t7.*(t4650+t34.*(t2425-t2468))+t47.*(t2425-t2468)).*1.17633784675e-2+(t5365.*(t8315+t8.*(t30.*(t2425-t2468)+t68.*(t2425-t2468))))./4.0+t17.*(t8329+t17.*(t16.*(t30.*(t2425-t2468)+t68.*(t2425-t2468))+t8.*(t7.*(t4650+t34.*(t2425-t2468))+t47.*(t2425-t2468)))).*1.13264871585e-2+t9.*(t9.*(t16.*(t30.*(t2425-t2468)+t68.*(t2425-t2468))+t8.*(t7.*(t4650+t34.*(t2425-t2468))+t47.*(t2425-t2468))).*7.35522e-1+t17.*(t4654+t15.*(t4650+t34.*(t2425-t2468))).*7.35522e-1).*1.539925e-2);
t16308 = t8804+t8829+t9145+t9335+t9353+t9354+t10997+t10998+t11102+t11108+t11278+t11293+t11370+t11376+t11511+t11517+t11533+t11535+t11550+t11836+t11844+t12393+t12803+t12814+t12903+t12909+t13160+t13243+t13244+t13328+t13331+t13538+t13931+t13934+t14119+t14123+t14585+t14586+t14756+t14758;
t16309 = t8808+t8820+t9138+t9335+t9343+t9353+t10997+t10998+t11102+t11108+t11278+t11293+t11360+t11384+t11511+t11517+t11528+t11542+t11550+t11840+t11853+t12393+t12803+t12814+t12903+t12909+t13160+t13238+t13251+t13324+t13334+t13538+t13931+t13934+t14119+t14123+t14585+t14586+t14756+t14758;
t16311 = t8837+t8865+t9158+t9348+t9386+t9396+t11020+t11025+t11127+t11135+t11308+t11324+t11432+t11439+t11529+t11538+t11593+t11603+t11604+t11877+t11890+t12410+t12825+t12840+t12922+t12932+t13174+t13292+t13293+t13369+t13374+t13555+t13968+t13970+t14142+t14147+t14596+t14600+t14783+t14787;
t16312 = t8846+t8856+t9151+t9348+t9369+t9396+t11020+t11025+t11127+t11135+t11308+t11324+t11427+t11445+t11529+t11538+t11593+t11598+t11610+t11880+t11894+t12410+t12825+t12840+t12922+t12932+t13174+t13287+t13295+t13366+t13378+t13555+t13968+t13970+t14142+t14147+t14596+t14600+t14783+t14787;
t16322 = t8812+t8828+t10580+t10598+t11941+t12170+t12785+t12888+t13491+t13500+t13666+t13687+t13695+t13826+t13827+t13872+t14068+t14076+t14092+t14242+t14246+t14289+t14292+t14345+t14346+t14390+t14576+t14578+t15057+t15065+t15202+t15209;
t16323 = -yd.*(-t10580+t10587+t11945+t12174-t12785-t12888+t13485+t13494+t13662+t13685+t13690+t13830+t13831+t13870+t14072+t14081+t14093+t14243+t14245-t14289-t14345+t14393+t14575+t14579+t15059+t15062+t15204+t15206+t9.*(t10403+t9.*(t10158+t16.*(t4542-t6448)).*7.35522e-1).*1.539925e-2+t8.*(t4542-t6448).*5.01208083475e-2+t16.*(t4542-t6448).*1.17633784675e-2+t9.*(t10174+t9.*(t10158+t16.*(t4542-t6448))).*1.13264871585e-2);
t16324 = t8812+t8828+t10580+t10598+t11945+t12174+t12785+t12888+t13485+t13494+t13662+t13685+t13690+t13830+t13831+t13870+t14072+t14081+t14093+t14243+t14245+t14289+t14292+t14345+t14346+t14393+t14575+t14579+t15059+t15062+t15204+t15206;
t16331 = t7281+t7284+t7361+t7369+t9363+t9413+t10274+t10296+t11012+t11019+t11131+t11145+t11222+t11225+t11291+t11368+t11375+t11412+t11428+t11541+t11545+t11581+t11591+t11641+t11768+t11831+t11869+t11883+t11900+t11903+t12300+t12449+t12918+t12930+t13044+t13050+t13267+t13646+t13682+t13686+t13768+t13789+t14111+t14115+t14370+t14386+t14691+t14693+t14886+t14890;
t16333 = -xd.*(-t7281-t7284+t7345+t9363+t9413+t10264+t10290+t11012+t11019+t11131+t11145+t11222+t11225+t11291+t11368+t11375-t11412-t11428+t11541+t11545-t11581-t11591+t11641+t11768+t11831-t11869-t11883+t11900+t11903+t12300+t12449+t12918+t12930+t13044+t13050+t13267+t13646+t13677+t13681+t13763+t13777+t14111+t14115+t14370+t14386+t14691+t14693+t14886+t14890+t6.*t15.*(t4540+t5.*(t2425-t2468)).*7.326866269e-3);
t16334 = t7310+t7313+t7315+t7322+t9391+t9462+t10275+t10297+t11030+t11040+t11163+t11178+t11248+t11253+t11322+t11394+t11404+t11414+t11416+t11559+t11572+t11580+t11586+t11677+t11799+t11842+t11850+t11875+t11911+t11923+t12328+t12467+t12941+t12963+t13056+t13069+t13294+t13661+t13673+t13676+t13761+t13769+t14120+t14130+t14396+t14409+t14707+t14708+t14908+t14913;
t16335 = t7310+t7313+t7315+t7322+t9405+t9475+t10275+t10297+t11036+t11045+t11172+t11183+t11259+t11260+t11330+t11394+t11405+t11413+t11416+t11559+t11572+t11588+t11595+t11681+t11789+t11845+t11850+t11875+t11914+t11918+t12318+t12470+t12949+t12957+t13059+t13062+t13289+t13658+t13673+t13676+t13761+t13769+t14117+t14127+t14392+t14406+t14704+t14705+t14906+t14911;
t16337 = t5581+t5592+t7342+t7377+t9411+t9440+t10019+t10409+t10660+t10693+t10828+t10837+t11089+t11096+t11471+t11489+t11697+t11733+t11737+t11939+t11962+t12056+t12061+t12070+t12242+t12244+t12264+t12412+t12612+t12613+t12716+t12851+t12868+t12950+t12967+t13153+t13222+t13240+t13424+t13431+t13598+t14014+t14414+t14415+t14701+t14706+t14912+t14915+t15118+t15119;
t16338 = t5605+t5612+t7358+t7366+t9429+t9456+t10019+t10409+t10681+t10688+t10832+t10833+t11083+t11094+t11471+t11489+t11697+t11733+t11737+t11939+t11962+t12056+t12061+t12070+t12242+t12244+t12264+t12412+t12612+t12613+t12716+t12861+t12862+t12956+t12962+t13153+t13222+t13240+t13424+t13431+t13598+t14014+t14414+t14415+t14701+t14706+t14912+t14915+t15118+t15119;
t16343 = t5624+t5630+t7408+t7426+t9491+t9500+t10050+t10432+t10741+t10752+t10866+t10874+t11146+t11167+t11488+t11507+t11727+t11757+t11766+t11960+t11985+t12065+t12075+t12086+t12268+t12270+t12281+t12425+t12621+t12624+t12733+t12906+t12914+t13015+t13029+t13161+t13245+t13272+t13439+t13452+t13602+t14026+t14431+t14434+t14719+t14723+t14935+t14936+t15127+t15129;
t16345 = t5642+t5652+t7414+t7417+t9495+t9508+t10050+t10432+t10746+t10750+t10869+t10870+t11140+t11154+t11488+t11507+t11727+t11757+t11766+t11960+t11985+t12065+t12075+t12086+t12268+t12270+t12281+t12425+t12621+t12624+t12733+t12910+t12911+t13017+t13022+t13161+t13245+t13272+t13439+t13452+t13602+t14026+t14431+t14434+t14719+t14723+t14935+t14936+t15127+t15129;
t16349 = t7004+t7016+t7623+t7671+t7985+t8661+t9401+t9402+t9415+t9444+t9473+t9484+t9788+t9800+t10030+t10032+t10052+t10057+t10060+t10390+t10534+t11000+t11205+t11211+t11387+t11403+t11739+t11932+t11935+t12118+t12126+t12147+t12180+t12187+t12358+t12436+t12443+t12479+t12819+t12893+t13053+t13066+t13220+t13227+t13301+t13678+t13894+t13904+t13947+t13948+t14131+t14137+t14195+t14198+t14747+t14749+t15010+t15014;
t16351 = t6999+t7020+t7623+t7671+t7995+t8667+t9401+t9402+t9415+t9444+t9473+t9484+t9776+t9814+t10023+t10044+t10052+t10057+t10060+t10372+t10529+t11000+t11205+t11211+t11387+t11403+t11739+t11936+t11940+t12118+t12131+t12154+t12180+t12187+t12363+t12436+t12443+t12479+t12822+t12893+t13053+t13066+t13220+t13227+t13301+t13678+t13894+t13904+t13944+t13946+t14128+t14134+t14195+t14198+t14747+t14749+t15010+t15014;
t16364 = t5281+t5286+t5299+t5308+t7682+t7739+t8453+t8683+t8964+t8986+t9155+t9159+t9258+t9265+t9399+t9438+t9529+t9541+t9573+t9662+t9763+t9873+t9899+t9993+t9994+t9995+t10251+t10477+t10887+t10897+t11090+t11262+t11288+t11442+t11447+t11602+t11622+t11767+t11783+t11785+t11859+t11929+t12437+t12450+t12644+t12647+t12986+t13136+t13144+t13186+t13191+t13259+t13265+t13556+t13580+t13582+t13589+t13595+t13599+t14003+t14229+t14239+t14486+t14491+t14957+t14959+t15190+t15195;
t16366 = t7280+t7283+t8889+t8899+t10169+t10541+t11053+t11058+t11833+t11839+t12036+t12141+t12153+t12179+t12192+t12420+t12423+t12429+t12492+t12514+t12526+t12607+t12615+t12676+t12677+t12787+t12801+t12835+t12947+t12951+t13058+t13477+t13488+t13574+t13671+t13683+t13940+t14207+t14465+t14471+t14514+t14524+t14728+t14729+t14979+t14982+t15133+t15135+t15288+t15290;
t16367 = t7290+t7292+t8876+t8913+t10169+t10541+t11057+t11063+t11833+t11839+t12036+t12141+t12153+t12179+t12192+t12420+t12423+t12429+t12492+t12519+t12522+t12610+t12611+t12676+t12677+t12793+t12805+t12835+t12947+t12951+t13058+t13477+t13488+t13574+t13671+t13683+t13940+t14207+t14466+t14469+t14516+t14520+t14728+t14729+t14979+t14982+t15133+t15135+t15288+t15290;
t16388 = t5572+t5576+t5657+t6213+t6529+t6578+t7405+t7415+t7864+t7865+t7874+t7909+t7928+t7929+t8279+t8314+t8423+t8444+t8956+t8966+t9082+t9403+t9442+t9690+t9693+t9888+t9890+t10114+t10123+t10254+t10304+t10308+t10982+t10987+t11046+t11082+t11441+t11624+t11627+t11670+t11674+t11743+t11772+t11943+t11956+t12030+t12094+t12258+t12271+t12321+t12473+t12628+t12633+t12763+t12974+t13122+t13127+t13540+t13550+t13560+t13571+t13577+t13762+t13912+t13921+t14005+t14007+t14158+t14419+t14421+t14712+t14715+t15113+t15114+t15308+t15310;
t16389 = t5593+t5599+t5638+t6213+t6519+t6578+t7392+t7427+t7852+t7874+t7879+t7909+t7928+t7929+t8279+t8314+t8428+t8450+t8956+t8966+t9082+t9403+t9442+t9687+t9700+t9888+t9890+t10108+t10129+t10254+t10302+t10308+t10982+t10987+t11041+t11082+t11441+t11629+t11634+t11670+t11674+t11743+t11772+t11948+t11966+t12031+t12094+t12258+t12271+t12321+t12476+t12628+t12633+t12763+t12974+t13122+t13127+t13540+t13550+t13563+t13566+t13577+t13762+t13912+t13921+t14004+t14008+t14158+t14419+t14421+t14712+t14715+t15113+t15114+t15308+t15310;
t16404 = t8812+t8828+t10580+t10598+t11941+t12170+t12785+t12888+t14289+t14292+t14345+t14346+t15520+t15523+t15542+t15545+t15548+t15579+t15581+t15593+t15635+t15637+t15642+t15739+t15871+t15874+t15886+t15889+t15913+t15914+t15971+t15973;
t16405 = -yd.*(-t10580+t10587+t11945+t12174-t12785-t12888-t14289-t14345+t15521+t15522+t15544+t15546+t15547+t15578+t15583+t15594+t15632+t15639+t15644+t15740+t15872+t15873+t15887+t15888+t15911+t15912+t15970+t15972+t9.*(t10403+t9.*(t10158+t16.*(t4542-t6448)).*7.35522e-1).*1.539925e-2+t8.*(t4542-t6448).*5.01208083475e-2+t16.*(t4542-t6448).*1.17633784675e-2+t9.*(t10174+t9.*(t10158+t16.*(t4542-t6448))).*1.13264871585e-2);
t16406 = t8812+t8828+t10580+t10598+t11945+t12174+t12785+t12888+t14289+t14292+t14345+t14346+t15521+t15522+t15544+t15546+t15547+t15578+t15583+t15594+t15632+t15639+t15644+t15740+t15872+t15873+t15887+t15888+t15911+t15912+t15970+t15972;
t16407 = t5292+t5293+t7037+t7057+t8240+t8799+t9488+t9620+t9635+t9636+t9708+t9729+t9780+t10012+t10046+t10138+t10325+t10326+t10448+t10631+t10632+t10663+t10668+t10834+t10839+t10983+t11128+t11241+t11316+t11692+t11701+t11873+t11885+t12122+t12190+t12231+t12255+t12608+t12873+t12885+t12966+t12971+t13092+t13097+t13192+t13348+t13359+t13373+t13425+t13432+t13652+t13727+t13733+t13850+t13969+t14140+t14511+t14512+t14631+t14632+t14766+t14774+t14832+t14840+t15139+t15144+t15377+t15379;
t16408 = -xd.*(t5283+t5287+t7042+t7055+t9480-t9620+t9626+t9629+t9718-t10012+t10034-t10138+t10317-t10448+t10621+t10643+t10682+t10838+t10843+t10972+t11138-t11241+t11325+t11687-t11873-t11885+t12119+t12184-t12231-t12255+t12605+t12876+t12880-t12966+t12968+t13094+t13095+t13193+t13342-t13359-t13425+t13655-t13727-t13850-t14140+t14508+t14630+t14634+t14771+t14834+t14836+t15143+t15378+(t5598.*(t4540+t5.*(t2425-t2468)))./4.0+(t8713.*(t10158+t16.*(t4542-t6448)))./4.0+(t9187.*(t10403+t9.*(t10158+t16.*(t4542-t6448)).*7.35522e-1))./4.0+(t12689.*(t3418-t3879+t4324-t5228+t5802+t9.*(t71-t391).*4.5305948634e-2+t17.*(t426-t581).*7.35522e-1))./4.0+(t12945.*(t1987-t2621+t3452-t4730+t5359+t9.*(t71-t391).*6.1597e-2+t17.*(t426-t581)))./4.0+(t10936.*(t1589-t2213+t3195-t4346+t4355+t4748.*7.35522e-1+t2772.*(t71-t391)+t2775.*(t71-t391)))./4.0+(t2701.*(t5122+t5.*(t2425-t2468).*3.587895))./4.0+(t4557.*(t5124-t6795))./4.0+(t4774.*(t5110-t6808))./4.0+(t6750.*(t4542-t6448))./4.0+(t6744.*(t10384+t16.*(t4542-t6448).*1.666555))./4.0+(t11340.*(t249-t391.*(1.1e+1./1.25e+2)-t1912.*4.252e-3+t3505+t5357+t693.*(t71-t391)+t784.*(t71-t391)))./4.0+(t10753.*(t10174+t9.*(t10158+t16.*(t4542-t6448))))./4.0+t15.*t7039.*(t4542-t6448).*3.064865e-1+(t15.*t9236.*(t4542-t6448))./4.0);
t16409 = t5283+t5287+t7042+t7055+t8240+t8799+t9480+t9620+t9626+t9636+t9708+t9729+t9780+t10012+t10046+t10138+t10325+t10326+t10448+t10631+t10643+t10668+t10682+t10838+t10843+t10983+t11138+t11241+t11325+t11692+t11701+t11873+t11885+t12122+t12190+t12231+t12255+t12608+t12876+t12880+t12966+t12971+t13094+t13095+t13193+t13348+t13359+t13373+t13425+t13432+t13655+t13727+t13733+t13850+t13969+t14140+t14511+t14512+t14630+t14634+t14766+t14774+t14834+t14836+t15139+t15144+t15377+t15379;
t16410 = t5264+t5266+t7000+t7021+t8223+t8769+t9452+t9617+t9655+t9656+t9740+t9777+t9822+t10061+t10067+t10142+t10340+t10369+t10475+t10593+t10611+t10658+t10689+t10817+t10823+t11002+t11103+t11286+t11290+t11707+t11714+t11888+t11896+t12128+t12210+t12256+t12278+t12618+t12846+t12864+t12992+t12998+t13063+t13072+t13180+t13385+t13390+t13401+t13442+t13455+t13642+t13751+t13756+t13861+t13983+t14152+t14535+t14537+t14605+t14607+t14794+t14798+t14807+t14814+t15152+t15160+t15383+t15387;
t16411 = t5272+t5273+t7005+t7017+t8223+t8769+t9437+t9610+t9655+t9656+t9740+t9777+t9822+t10061+t10067+t10142+t10340+t10369+t10475+t10603+t10623+t10658+t10689+t10822+t10826+t11002+t11111+t11290+t11295+t11707+t11714+t11888+t11896+t12128+t12210+t12256+t12278+t12618+t12853+t12856+t12992+t12998+t13068+t13070+t13184+t13385+t13390+t13401+t13442+t13455+t13643+t13751+t13756+t13861+t13983+t14152+t14535+t14537+t14603+t14610+t14794+t14803+t14807+t14809+t15152+t15160+t15383+t15387;
t16413 = t5534+t5541+t5544+t5557+t6273+t6622+t7385+t7398+t7778+t7837+t7839+t7964+t8193+t8348+t8366+t8373+t8405+t8416+t8488+t8490+t8514+t8790+t8826+t9057+t9063+t9288+t9377+t9431+t9478+t9494+t9503+t9504+t9512+t9911+t9921+t10345+t10514+t11168+t11220+t11238+t11531+t11547+t11569+t11571+t11769+t11838+t11866+t11927+t12159+t12287+t12289+t12306+t12334+t12353+t12587+t12826+t12978+t12979+t13081+t13089+t13239+t13255+t13308+t13364+t13372+t13388+t13612+t13628+t13691+t13914+t13973+t13999+t14001+t14248+t14732+t14735+t14775+t14791+t14984+t14989+t15027+t15038+t15169+t15175+t15393+t15397;
t16415 = t5538+t5554+t5559+t5562+t6273+t6622+t7385+t7398+t7789+t7837+t7839+t7964+t8207+t8348+t8366+t8373+t8405+t8416+t8488+t8490+t8514+t8776+t8806+t9051+t9058+t9288+t9390+t9445+t9478+t9494+t9503+t9504+t9512+t9911+t9921+t10345+t10514+t11168+t11226+t11229+t11537+t11547+t11557+t11571+t11777+t11838+t11866+t11927+t12159+t12287+t12289+t12310+t12334+t12353+t12587+t12826+t12978+t12979+t13086+t13093+t13246+t13261+t13309+t13364+t13372+t13388+t13612+t13628+t13696+t13914+t13973+t13999+t14001+t14248+t14732+t14735+t14778+t14788+t14984+t14989+t15029+t15035+t15169+t15175+t15393+t15397;
t16416 = t5516+t5522+t5589+t5597+t6258+t6613+t7371+t7412+t7763+t7817+t7851+t7976+t8161+t8352+t8368+t8386+t8403+t8419+t8474+t8513+t8534+t8861+t8902+t9085+t9088+t9307+t9406+t9449+t9474+t9476+t9482+t9510+t9514+t9905+t9906+t10318+t10531+t11150+t11246+t11267+t11546+t11566+t11570+t11601+t11800+t11825+t11841+t11926+t12132+t12286+t12288+t12303+t12336+t12338+t12586+t12811+t12983+t12985+t13104+t13112+t13270+t13282+t13316+t13370+t13383+t13394+t13601+t13611+t13708+t13890+t13979+t13984+t13992+t14241+t14733+t14737+t14811+t14829+t14987+t14994+t15051+t15060+t15149+t15158+t15380+t15388;
t16417 = t5514+t5527+t5571+t5575+t6258+t6613+t7371+t7412+t7777+t7817+t7851+t7976+t8172+t8352+t8368+t8386+t8403+t8419+t8474+t8513+t8534+t8844+t8878+t9078+t9084+t9307+t9425+t9449+t9474+t9482+t9485+t9510+t9514+t9905+t9906+t10318+t10531+t11150+t11254+t11258+t11546+t11570+t11578+t11596+t11812+t11825+t11841+t11926+t12132+t12286+t12288+t12303+t12338+t12340+t12586+t12811+t12983+t12985+t13109+t13116+t13277+t13286+t13318+t13370+t13383+t13394+t13601+t13611+t13710+t13890+t13979+t13984+t13992+t14241+t14733+t14737+t14817+t14826+t14987+t14994+t15052+t15058+t15149+t15158+t15380+t15388;
t16418 = xd.*(-t5516-t5522-t5589-t5597-t6249-t6602-t7400-t7763-t7840-t7965-t8161+t8352+t8368+t8386+t8403+t8419+t8474+t8513+t8534+t8844+t8878+t9078+t9084+t9307+t9425+t9449+t9474+t9482+t9485+t9510+t9514+t9905+t9906+t10318+t10531+t11150+t11254+t11258+t11546+t11570+t11578+t11596+t11812+t11825+t11841+t11926+t12132+t12286+t12288+t12303+t12338+t12340+t12586+t12811+t12983+t12985+t13109+t13116+t13277+t13286+t13318+t13370+t13383+t13394+t13601+t13611+t13710+t13890+t13979+t13984+t13992+t14241+t14733+t14737+t14817+t14826+t14987+t14994+t15052+t15058+t15149+t15158+t15380+t15388+t5.*t12.*t6431.*2.01382560198e-1+t5.*t12.*t7224.*6.23745e-2);
t16419 = t5262+t5587+t6225+t6245+t6247+t6267+t6287+t6309+t6356+t6427+t6586+t6598+t6600+t6624+t6625+t7355+t7374+t7805+t7807+t7894+t8294+t8347+t8382+t8383+t8424+t8431+t8462+t8782+t8810+t9398+t9420+t9450+t9509+t9511+t9590+t9705+t9738+t9862+t9897+t10252+t10323+t10341+t10442+t10506+t10836+t10846+t11084+t11209+t11239+t11710+t11738+t11748+t11765+t12066+t12127+t12136+t12139+t12261+t12274+t12442+t12516+t12517+t12651+t12675+t12736+t12965+t12973+t12981+t13079+t13544+t13557+t13586+t13767+t13807+t13815+t13916+t13927+t14040+t14041+t14050+t14179+t14294+t14295+t14352+t14581+t14583+t15094+t15104+t15296+t15305+t15344+t15345+t15469+t15471;
t16421 = t5252+t5569+t6239+t6245+t6247+t6267+t6287+t6309+t6356+t6427+t6597+t6598+t6600+t6624+t6625+t7332+t7387+t7792+t7821+t7876+t8282+t8347+t8382+t8383+t8424+t8431+t8462+t8782+t8810+t9419+t9441+t9450+t9509+t9511+t9590+t9705+t9738+t9874+t9901+t10242+t10323+t10341+t10442+t10506+t10836+t10846+t11080+t11209+t11239+t11710+t11738+t11758+t11775+t12071+t12127+t12136+t12139+t12265+t12277+t12442+t12516+t12517+t12651+t12675+t12739+t12965+t12973+t12981+t13079+t13546+t13554+t13586+t13767+t13807+t13819+t13919+t13923+t14040+t14041+t14050+t14181+t14294+t14295+t14352+t14581+t14583+t15096+t15100+t15301+t15303+t15344+t15345+t15469+t15471;
t16422 = t5229+t5533+t6212+t6256+t6257+t6277+t6317+t6337+t6340+t6444+t6577+t6609+t6611+t6655+t6658+t7330+t7388+t7791+t7823+t7908+t8313+t8362+t8367+t8392+t8413+t8452+t8454+t8868+t8869+t9346+t9356+t9417+t9520+t9531+t9632+t9756+t9765+t9836+t9846+t10236+t10358+t10364+t10459+t10539+t10852+t10872+t11076+t11235+t11251+t11724+t11736+t11745+t11787+t12057+t12155+t12162+t12171+t12235+t12247+t12461+t12544+t12546+t12679+t12701+t12721+t12996+t13012+t13031+t13098+t13506+t13542+t13608+t13776+t13814+t13836+t13892+t13906+t14052+t14060+t14075+t14163+t14310+t14315+t14365+t14608+t14613+t15072+t15080+t15275+t15281+t15371+t15372+t15479+t15484;
t16423 = t5241+t5551+t6199+t6256+t6257+t6277+t6317+t6337+t6340+t6444+t6569+t6609+t6611+t6655+t6658+t7352+t7376+t7806+t7808+t7895+t8306+t8362+t8367+t8392+t8413+t8452+t8454+t8868+t8869+t9358+t9370+t9417+t9520+t9531+t9632+t9756+t9765+t9845+t9852+t10228+t10358+t10364+t10459+t10539+t10852+t10872+t11070+t11235+t11251+t11734+t11742+t11745+t11787+t12058+t12155+t12162+t12171+t12240+t12253+t12461+t12544+t12546+t12679+t12701+t12724+t12996+t13012+t13031+t13098+t13513+t13537+t13608+t13787+t13814+t13836+t13896+t13901+t14052+t14060+t14075+t14165+t14310+t14315+t14365+t14608+t14613+t15074+t15078+t15278+t15279+t15371+t15372+t15479+t15484;
t16434 = t7280+t7283+t8889+t8899+t10169+t10541+t11053+t11058+t12514+t12526+t12607+t12615+t12787+t12801+t14199+t14202+t14263+t14316+t14319+t14331+t14336+t14432+t14465+t14471+t14484+t14514+t14524+t14593+t14594+t14746+t14978+t14983+t15086+t15091+t15198+t15203+t15213+t15382+t15404+t15405+t15408+t15528+t15929+t15930+t15977+t15979+t15995+t15996+t16015+t16016;
t16435 = t7280+t7283+t8889+t8899+t10176+t10545+t11053+t11058+t12514+t12526+t12607+t12615+t12787+t12801+t14201+t14206+t14265+t14318+t14322+t14333+t14339+t14429+t14465+t14471+t14485+t14514+t14524+t14597+t14598+t14744+t14980+t14981+t15087+t15090+t15200+t15201+t15212+t15386+t15403+t15406+t15407+t15529+t15927+t15928+t15976+t15978+t15994+t15997+t16014+t16018;
t16436 = -xd.*(t7290+t7292+t8876+t8913+t10169+t10541+t11057+t11063+t12519+t12522+t12610+t12611+t12793+t12805+t14199+t14202+t14263+t14316+t14319+t14331+t14336+t14432+t14466+t14469+t14484+t14516+t14520+t14593+t14594+t14746+t14978+t14983+t15086+t15091+t15198+t15203+t15213+t15382+t15404+t15405+t15408+t15528+t15929+t15930+t15977+t15979+t15995+t15996+t16015+t16016);
t16437 = t7309+t7314+t8781+t8789+t10195+t10551+t11032+t11043+t12496+t12509+t12592+t12598+t12766+t12779+t14210+t14212+t14268+t14324+t14332+t14341+t14343+t14442+t14447+t14453+t14488+t14492+t14501+t14611+t14612+t14753+t14985+t14993+t15103+t15111+t15205+t15210+t15226+t15391+t15411+t15417+t15418+t15531+t15944+t15945+t15984+t15987+t16005+t16006+t16025+t16026;
t16449 = t5292+t5293+t7037+t7057+t8240+t8799+t9488+t9635+t10632+t10663+t10834+t10839+t11128+t11316+t12230+t12252+t12322+t12325+t12355+t12541+t12549+t12593+t12625+t12709+t12711+t12873+t12885+t13092+t13097+t13192+t13254+t13453+t13465+t13652+t13725+t13745+t13754+t13755+t13765+t13960+t14037+t14151+t14155+t14307+t14631+t14632+t14832+t14840+t15211+t15214+t15339+t15346+t15390+t15410+t15412+t15492+t15493+t15497+t15508+t15611+t15897+t15903+t15948+t15952+t15962+t15963+t16010+t16011;
t16450 = -xd.*(t5283+t5287+t7042+t7055+t9480+t9626+t10643+t10682+t10838+t10843+t11138+t11325-t12230+t12246+t12314-t12541+t12547-t12593-t12625+t12700+t12876+t12880+t13094+t13095+t13193-t13254-t13453-t13465+t13655+t13721+t13739-t13754-t13765+t13953+t14036+t14149+t14306+t14630+t14634+t14834+t14836-t15211-t15339-t15390-t15410-t15412-t15492-t15493-t15497+t15901+t15949+(t5598.*(t4540+t5.*(t2425-t2468)))./4.0+(t13380.*(t10158+t16.*(t4542-t6448)))./4.0+(t14541.*(t10403+t9.*(t10158+t16.*(t4542-t6448)).*7.35522e-1))./4.0+(t12689.*(t3418-t3879+t4324+t11855+t9.*(t71-t391).*4.5305948634e-2+t17.*(t426-t581).*7.35522e-1+t9.*(t9166-t11658).*7.35522e-1))./4.0+(t2701.*(t5122+t5.*(t2425-t2468).*3.587895))./4.0+(t9830.*(t5124-t6795))./4.0+(t9884.*(t5110-t6808))./4.0+(t10964.*(t4542-t6448))./4.0+(t10936.*(t1589-t2213-t4346+t4355+t9454+t11863+t2772.*(t71-t391)+t2775.*(t71-t391)))./4.0+(t12705.*(t3423+t3845+t3888+t3925+t4339+t9.*(t210+t2107+t7423+t9121).*7.35522e-1+t17.*(t9166-t11658).*7.35522e-1))./4.0+(t12867.*(t10384+t16.*(t4542-t6448).*1.666555))./4.0+(t11340.*(t249-t391.*(1.1e+1./1.25e+2)-t1912.*4.252e-3+t3505+t13496+t693.*(t71-t391)+t784.*(t71-t391)))./4.0+(t14918.*(t10174+t9.*(t10158+t16.*(t4542-t6448))))./4.0+(t12953.*(t2091+t2497+t2579+t2680+t3516+t9.*(t210+t2107+t7423+t9121)+t17.*(t9166-t11658)))./4.0+(t12945.*(t1987-t2621+t3452+t11654+t9.*(t71-t391).*6.1597e-2+t17.*(t426-t581)+t9.*(t9166-t11658)))./4.0+t15.*t12396.*(t4542-t6448).*3.064865e-1+(t15.*t13140.*(t4542-t6448))./4.0);
t16451 = t5283+t5287+t7042+t7055+t8240+t8799+t9480+t9626+t10643+t10682+t10838+t10843+t11138+t11325+t12230+t12252+t12322+t12325+t12355+t12541+t12549+t12593+t12625+t12709+t12711+t12876+t12880+t13094+t13095+t13193+t13254+t13453+t13465+t13655+t13725+t13745+t13754+t13755+t13765+t13960+t14037+t14151+t14155+t14307+t14630+t14634+t14834+t14836+t15211+t15214+t15339+t15346+t15390+t15410+t15412+t15492+t15493+t15497+t15508+t15611+t15897+t15903+t15948+t15952+t15962+t15963+t16010+t16011;
t16452 = t5264+t5266+t7000+t7021+t8223+t8769+t9452+t9617+t10593+t10611+t10817+t10823+t11103+t11286+t12262+t12273+t12342+t12350+t12368+t12557+t12558+t12600+t12638+t12718+t12732+t12846+t12864+t13063+t13072+t13180+t13281+t13470+t13482+t13642+t13740+t13752+t13758+t13766+t13798+t13971+t14039+t14160+t14162+t14309+t14605+t14607+t14798+t14814+t15222+t15227+t15350+t15365+t15394+t15426+t15427+t15507+t15511+t15512+t15515+t15614+t15904+t15906+t15957+t15960+t15964+t15965+t16012+t16013;
t16453 = t5272+t5273+t7005+t7017+t8223+t8769+t9437+t9610+t10603+t10623+t10822+t10826+t11111+t11295+t12262+t12273+t12342+t12350+t12368+t12557+t12558+t12600+t12638+t12718+t12732+t12853+t12856+t13068+t13070+t13184+t13281+t13470+t13482+t13643+t13740+t13752+t13758+t13766+t13798+t13971+t14039+t14160+t14162+t14309+t14603+t14610+t14803+t14809+t15222+t15227+t15350+t15365+t15394+t15426+t15427+t15507+t15511+t15512+t15515+t15614+t15904+t15906+t15957+t15960+t15964+t15965+t16012+t16013;
t16461 = t5534+t5541+t5544+t5557+t6273+t6622+t7778+t8193+t8790+t8826+t9057+t9063+t9377+t9431+t10331+t10348+t10391+t10526+t10527+t10572+t10582+t10671+t10903+t10914+t10916+t11220+t11238+t11392+t11402+t11526+t11527+t11531+t11569+t11731+t11732+t11747+t11769+t12054+t12076+t12297+t12302+t12306+t12561+t12837+t13081+t13089+t13239+t13255+t13308+t13691+t13936+t13949+t14074+t14103+t14110+t14129+t14146+t14237+t14357+t14359+t14389+t14552+t14775+t14791+t15027+t15038+t15264+t15266+t15402+t15419+t15421+t15441+t15443+t15504+t15505+t15513+t15527+t15612+t15956+t15961+t15991+t15993+t15999+t16000+t16019+t16021;
